simulink model "model3robots"  (R2022a)
settings: Solver=VariableStepAuto  StartTime=0.0  StopTime=Inf  RelTol=1e-3
(part 2 of 2)

== stateflow chart model3robots/Supervisor ==
  settings: executeAtInitialization=1
  state s1
  state s2
  state s3
  state s4
  state s5
  state s6
  state s7
  state s8
  state s9
  state s10
  state s11
  state s12
  state s13
  state s14
  state s15
  state s16
  state s17
  state s18
  state s19
  state s20
  state s21
  state s22
  state s23
  state s24
  state s25
  state s26
  state s27
  state s28
  state s29
  state s30
  state s31
  state s32
  state s33
  state s34
  state s35
  state s36
  state s37
  state s38
  state s39
  state s40
  state s41
  state s42
  state s43
  state s44
  state s45
  state s46
  state s47
  state s48
  state s49
  state s50
  state s51
  state s52
  state s53
  state s54
  state s55
  state s56
  state s57
  state s58
  state s59
  state s60
  state s61
  state s62
  state s63
  state s64
  state s65
  state s66
  state s67
  state s68
  state s69
  state s70
  state s71
  state s72
  state s73
  state s74
  state s75
  state s76
  state s77
  state s78
  state s79
  state s80
  state s81
  state s82
  state s83
  state s84
  state s85
  state s86
  state s87
  state s88
  state s89
  state s90
  state s91
  state s92
  state s93
  state s94
  state s95
  state s96
  state s97
  state s98
  state s99
  state s100
  state s101
  state s102
  state s103
  state s104
  state s105
  state s106
  state s107
  state s108
  state s109
  state s110
  state s111
  state s112
  state s113
  state s114
  state s115
  state s116
  state s117
  state s118
  state s119
  state s120
  state s121
  state s122
  state s123
  state s124
  state s125
  state s126
  state s127
  state s128
  state s129
  state s130
  state s131
  state s132
  state s133
  state s134
  state s135
  state s136
  state s137
  state s138
  state s139
  state s140
  state s141
  state s142
  state s143
  state s144
  state s145
  state s146
  state s147
  state s148
  state s149
  state s150
  state s151
  state s152
  state s153
  state s154
  state s155
  state s156
  state s157
  state s158
  state s159
  state s160
  state s161
  state s162
  state s163
  state s164
  state s165
  state s166
  state s167
  state s168
  state s169
  state s170
  state s171
  state s172
  state s173
  state s174
  state s175
  state s176
  state s177
  state s178
  state s179
  state s180
  state s181
  state s182
  state s183
  state s184
  state s185
  state s186
  state s187
  state s188
  state s189
  state s190
  state s191
  state s192
  state s193
  state s194
  state s195
  state s196
  state s197
  state s198
  state s199
  state s200
  state s201
  state s202
  state s203
  state s204
  state s205
  state s206
  state s207
  state s208
  state s209
  state s210
  state s211
  state s212
  state s213
  state s214
  state s215
  state s216
  state s217
  state s218
  state s219
  state s220
  state s221
  state s222
  state s223
  state s224
  state s225
  state s226
  state s227
  state s228
  state s229
  state s230
  state s231
  state s232
  state s233
  state s234
  state s235
  state s236
  state s237
  state s238
  state s239
  state s240
  state s241
  state s242
  state s243
  state s244
  state s245
  state s246
  state s247
  state s248
  state s249
  state s250
  state s251
  state s252
  state s253
  state s254
  state s255
  state s256
  state s257
  state s258
  state s259
  state s260
  state s261
  state s262
  state s263
  state s264
  state s265
  state s266
  state s267
  state s268
  state s269
  state s270
  state s271
  state s272
  state s273
  state s274
  state s275
  state s276
  state s277
  state s278
  state s279
  state s280
  state s281
  state s282
  state s283
  state s284
  state s285
  state s286
  state s287
  state s288
  state s289
  state s290
  state s291
  state s292
  state s293
  state s294
  state s295
  state s296
  state s297
  state s298
  state s299
  state s300
  state s301
  state s302
  state s303
  state s304
  state s305
  state s306
  state s307
  state s308
  state s309
  state s310
  state s311
  state s312
  state s313
  state s314
  state s315
  state s316
  state s317
  state s318
  state s319
  state s320
  state s321
  state s322
  state s323
  state s324
  state s325
  state s326
  state s327
  state s328
  state s329
  state s330
  state s331
  state s332
  state s333
  state s334
  state s335
  state s336
  state s337
  state s338
  state s339
  state s340
  state s341
  state s342
  state s343
  state s344
  state s345
  state s346
  state s347
  state s348
  state s349
  state s350
  state s351
  state s352
  state s353
  state s354
  state s355
  state s356
  state s357
  state s358
  state s359
  state s360
  state s361
  state s362
  state s363
  state s364
  state s365
  state s366
  state s367
  state s368
  state s369
  state s370
  state s371
  state s372
  state s373
  state s374
  state s375
  state s376
  state s377
  state s378
  state s379
  state s380
  state s381
  state s382
  state s383
  state s384
  state s385
  state s386
  state s387
  state s388
  state s389
  state s390
  state s391
  state s392
  state s393
  state s394
  state s395
  state s396
  state s397
  state s398
  state s399
  state s400
  state s401
  state s402
  state s403
  state s404
  state s405
  state s406
  state s407
  state s408
  state s409
  state s410
  state s411
  state s412
  state s413
  state s414
  state s415
  state s416
  state s417
  state s418
  state s419
  state s420
  state s421
  state s422
  state s423
  state s424
  state s425
  state s426
  state s427
  state s428
  state s429
  state s430
  state s431
  state s432
  state s433
  state s434
  state s435
  state s436
  state s437
  state s438
  state s439
  state s440
  state s441
  state s442
  state s443
  state s444
  state s445
  state s446
  state s447
  state s448
  state s449
  state s450
  state s451
  state s452
  state s453
  state s454
  state s455
  state s456
  state s457
  state s458
  state s459
  state s460
  state s461
  state s462
  (default) -> s19
  s4 -> s1 [order 4] : R3l {send(R3l_o);}
  s23 -> s1 [order 3] : R2l {send(R2l_o);}
  s157 -> s1 [order 1] : R1l {send(R1l_o);}
  s1 -> s157 [order 1] : R1r {send(R1r_o);}
  s1 -> s23 [order 2] : R2r {send(R2r_o);}
  s1 -> s4 [order 3] : R3r {send(R3r_o);}
  s3 -> s2 [order 3] : R3d {send(R3d_o);}
  s5 -> s2 [order 4] : R3l {send(R3l_o);}
  s9 -> s2 [order 1] : R2d {send(R2d_o);}
  s24 -> s2 [order 2] : R2l {send(R2l_o);}
  s2 -> s24 [order 1] : R2r {send(R2r_o);}
  s2 -> s9 [order 2] : R2u {send(R2u_o);}
  s2 -> s5 [order 3] : R3r {send(R3r_o);}
  s2 -> s3 [order 4] : R3u {send(R3u_o);}
  s4 -> s3 [order 3] : R3d {send(R3d_o);}
  s6 -> s3 [order 5] : R3l {send(R3l_o);}
  s10 -> s3 [order 2] : R2d {send(R2d_o);}
  s158 -> s3 [order 1] : R1l {send(R1l_o);}
  s3 -> s158 [order 1] : R1r {send(R1r_o);}
  s3 -> s10 [order 2] : R2u {send(R2u_o);}
  s3 -> s6 [order 4] : R3r {send(R3r_o);}
  s3 -> s4 [order 5] : R3u {send(R3u_o);}
  s7 -> s4 [order 5] : R3l {send(R3l_o);}
  s11 -> s4 [order 2] : R2d {send(R2d_o);}
  s159 -> s4 [order 1] : R1l {send(R1l_o);}
  s4 -> s159 [order 1] : R1r {send(R1r_o);}
  s4 -> s11 [order 2] : R2u {send(R2u_o);}
  s4 -> s7 [order 5] : R3r {send(R3r_o);}
  s6 -> s5 [order 4] : R3d {send(R3d_o);}
  s12 -> s5 [order 2] : R2d {send(R2d_o);}
  s25 -> s5 [order 4] : R2l {send(R2l_o);}
  s160 -> s5 [order 1] : R1l {send(R1l_o);}
  s5 -> s160 [order 1] : R1r {send(R1r_o);}
  s5 -> s25 [order 2] : R2r {send(R2r_o);}
  s5 -> s12 [order 3] : R2u {send(R2u_o);}
  s5 -> s6 [order 5] : R3u {send(R3u_o);}
  s7 -> s6 [order 4] : R3d {send(R3d_o);}
  s13 -> s6 [order 2] : R2d {send(R2d_o);}
  s26 -> s6 [order 4] : R2l {send(R2l_o);}
  s161 -> s6 [order 1] : R1l {send(R1l_o);}
  s6 -> s161 [order 1] : R1r {send(R1r_o);}
  s6 -> s26 [order 2] : R2r {send(R2r_o);}
  s6 -> s13 [order 3] : R2u {send(R2u_o);}
  s6 -> s7 [order 6] : R3u {send(R3u_o);}
  s6 -> s7 [order 7] : R3ureq {send(R3ureq_o);}
  s14 -> s7 [order 2] : R2d {send(R2d_o);}
  s27 -> s7 [order 4] : R2l {send(R2l_o);}
  s162 -> s7 [order 1] : R1l {send(R1l_o);}
  s7 -> s162 [order 1] : R1r {send(R1r_o);}
  s7 -> s27 [order 2] : R2r {send(R2r_o);}
  s7 -> s14 [order 3] : R2u {send(R2u_o);}
  s10 -> s8 [order 5] : R3l {send(R3l_o);}
  s28 -> s8 [order 3] : R2l {send(R2l_o);}
  s164 -> s8 [order 1] : R1l {send(R1l_o);}
  s8 -> s164 [order 1] : R1r {send(R1r_o);}
  s8 -> s28 [order 2] : R2r {send(R2r_o);}
  s8 -> s10 [order 3] : R3r {send(R3r_o);}
  s10 -> s9 [order 4] : R3d {send(R3d_o);}
  s12 -> s9 [order 4] : R3l {send(R3l_o);}
  s30 -> s9 [order 3] : R2l {send(R2l_o);}
  s9 -> s30 [order 2] : R2r {send(R2r_o);}
  s9 -> s12 [order 3] : R3r {send(R3r_o);}
  s9 -> s10 [order 4] : R3u {send(R3u_o);}
  s11 -> s10 [order 3] : R3d {send(R3d_o);}
  s13 -> s10 [order 5] : R3l {send(R3l_o);}
  s31 -> s10 [order 3] : R2l {send(R2l_o);}
  s165 -> s10 [order 1] : R1l {send(R1l_o);}
  s10 -> s165 [order 1] : R1r {send(R1r_o);}
  s10 -> s31 [order 3] : R2r {send(R2r_o);}
  s10 -> s13 [order 6] : R3r {send(R3r_o);}
  s10 -> s11 [order 7] : R3u {send(R3u_o);}
  s14 -> s11 [order 5] : R3l {send(R3l_o);}
  s166 -> s11 [order 1] : R1l {send(R1l_o);}
  s11 -> s166 [order 1] : R1r {send(R1r_o);}
  s11 -> s14 [order 4] : R3r {send(R3r_o);}
  s13 -> s12 [order 4] : R3d {send(R3d_o);}
  s32 -> s12 [order 4] : R2l {send(R2l_o);}
  s167 -> s12 [order 1] : R1l {send(R1l_o);}
  s12 -> s167 [order 1] : R1r {send(R1r_o);}
  s12 -> s32 [order 3] : R2r {send(R2r_o);}
  s12 -> s13 [order 5] : R3u {send(R3u_o);}
  s14 -> s13 [order 4] : R3d {send(R3d_o);}
  s33 -> s13 [order 4] : R2l {send(R2l_o);}
  s168 -> s13 [order 1] : R1l {send(R1l_o);}
  s13 -> s168 [order 1] : R1r {send(R1r_o);}
  s13 -> s33 [order 3] : R2r {send(R2r_o);}
  s13 -> s14 [order 6] : R3u {send(R3u_o);}
  s13 -> s14 [order 7] : R3ureq {send(R3ureq_o);}
  s34 -> s14 [order 4] : R2l {send(R2l_o);}
  s169 -> s14 [order 1] : R1l {send(R1l_o);}
  s14 -> s169 [order 1] : R1r {send(R1r_o);}
  s14 -> s34 [order 3] : R2r {send(R2r_o);}
  s16 -> s15 [order 3] : R3d {send(R3d_o);}
  s17 -> s15 [order 3] : R3l {send(R3l_o);}
  s22 -> s15 [order 2] : R2d {send(R2d_o);}
  s35 -> s15 [order 2] : R2l {send(R2l_o);}
  s15 -> s35 [order 1] : R2r {send(R2r_o);}
  s15 -> s22 [order 2] : R2u {send(R2u_o);}
  s15 -> s17 [order 3] : R3r {send(R3r_o);}
  s15 -> s16 [order 4] : R3u {send(R3u_o);}
  s18 -> s16 [order 4] : R3l {send(R3l_o);}
  s23 -> s16 [order 2] : R2d {send(R2d_o);}
  s36 -> s16 [order 2] : R2l {send(R2l_o);}
  s16 -> s36 [order 1] : R2r {send(R2r_o);}
  s16 -> s23 [order 2] : R2u {send(R2u_o);}
  s16 -> s18 [order 4] : R3r {send(R3r_o);}
  s18 -> s17 [order 3] : R3d {send(R3d_o);}
  s20 -> s17 [order 5] : R3l {send(R3l_o);}
  s38 -> s17 [order 3] : R2l {send(R2l_o);}
  s62 -> s17 [order 1] : R1d {send(R1d_o);}
  s17 -> s62 [order 1] : R1u {send(R1u_o);}
  s17 -> s38 [order 2] : R2r {send(R2r_o);}
  s17 -> s20 [order 4] : R3r {send(R3r_o);}
  s17 -> s18 [order 5] : R3u {send(R3u_o);}
  s21 -> s18 [order 5] : R3l {send(R3l_o);}
  s39 -> s18 [order 3] : R2l {send(R2l_o);}
  s63 -> s18 [order 1] : R1d {send(R1d_o);}
  s18 -> s63 [order 1] : R1u {send(R1u_o);}
  s18 -> s39 [order 2] : R2r {send(R2r_o);}
  s18 -> s21 [order 5] : R3r {send(R3r_o);}
  s20 -> s19 [order 4] : R3d {send(R3d_o);}
  s25 -> s19 [order 3] : R2d {send(R2d_o);}
  s64 -> s19 [order 1] : R1d {send(R1d_o);}
  s19 -> s64 [order 1] : R1u {send(R1u_o);}
  s19 -> s25 [order 2] : R2u {send(R2u_o);}
  s19 -> s20 [order 3] : R3u {send(R3u_o);}
  s21 -> s20 [order 4] : R3d {send(R3d_o);}
  s26 -> s20 [order 3] : R2d {send(R2d_o);}
  s40 -> s20 [order 3] : R2l {send(R2l_o);}
  s65 -> s20 [order 1] : R1d {send(R1d_o);}
  s20 -> s65 [order 1] : R1u {send(R1u_o);}
  s20 -> s40 [order 2] : R2r {send(R2r_o);}
  s20 -> s26 [order 3] : R2u {send(R2u_o);}
  s20 -> s21 [order 6] : R3u {send(R3u_o);}
  s20 -> s21 [order 7] : R3ureq {send(R3ureq_o);}
  s27 -> s21 [order 3] : R2d {send(R2d_o);}
  s41 -> s21 [order 3] : R2l {send(R2l_o);}
  s66 -> s21 [order 1] : R1d {send(R1d_o);}
  s21 -> s66 [order 1] : R1u {send(R1u_o);}
  s21 -> s41 [order 2] : R2r {send(R2r_o);}
  s21 -> s27 [order 3] : R2u {send(R2u_o);}
  s23 -> s22 [order 7] : R3d {send(R3d_o);}
  s28 -> s22 [order 2] : R2d {send(R2d_o);}
  s42 -> s22 [order 3] : R2l {send(R2l_o);}
  s171 -> s22 [order 1] : R1l {send(R1l_o);}
  s22 -> s171 [order 1] : R1r {send(R1r_o);}
  s22 -> s42 [order 3] : R2r {send(R2r_o);}
  s22 -> s28 [order 4] : R2u {send(R2u_o);}
  s22 -> s28 [order 5] : R2ureq {send(R2ureq_o);}
  s22 -> s23 [order 6] : R3u {send(R3u_o);}
  s29 -> s23 [order 2] : R2d {send(R2d_o);}
  s43 -> s23 [order 3] : R2l {send(R2l_o);}
  s172 -> s23 [order 1] : R1l {send(R1l_o);}
  s23 -> s172 [order 1] : R1r {send(R1r_o);}
  s23 -> s43 [order 4] : R2r {send(R2r_o);}
  s23 -> s29 [order 5] : R2u {send(R2u_o);}
  s23 -> s29 [order 6] : R2ureq {send(R2ureq_o);}
  s25 -> s24 [order 8] : R3l {send(R3l_o);}
  s30 -> s24 [order 2] : R2d {send(R2d_o);}
  s44 -> s24 [order 3] : R2l {send(R2l_o);}
  s68 -> s24 [order 1] : R1d {send(R1d_o);}
  s24 -> s68 [order 1] : R1u {send(R1u_o);}
  s24 -> s44 [order 3] : R2r {send(R2r_o);}
  s24 -> s30 [order 4] : R2u {send(R2u_o);}
  s24 -> s30 [order 5] : R2ureq {send(R2ureq_o);}
  s24 -> s25 [order 6] : R3r {send(R3r_o);}
  s26 -> s25 [order 7] : R3d {send(R3d_o);}
  s32 -> s25 [order 3] : R2d {send(R2d_o);}
  s47 -> s25 [order 3] : R2l {send(R2l_o);}
  s69 -> s25 [order 1] : R1d {send(R1d_o);}
  s173 -> s25 [order 1] : R1l {send(R1l_o);}
  s25 -> s173 [order 1] : R1r {send(R1r_o);}
  s25 -> s69 [order 2] : R1u {send(R1u_o);}
  s25 -> s47 [order 5] : R2r {send(R2r_o);}
  s25 -> s32 [order 6] : R2u {send(R2u_o);}
  s25 -> s32 [order 7] : R2ureq {send(R2ureq_o);}
  s25 -> s26 [order 9] : R3u {send(R3u_o);}
  s27 -> s26 [order 8] : R3d {send(R3d_o);}
  s33 -> s26 [order 3] : R2d {send(R2d_o);}
  s70 -> s26 [order 1] : R1d {send(R1d_o);}
  s174 -> s26 [order 1] : R1l {send(R1l_o);}
  s26 -> s174 [order 1] : R1r {send(R1r_o);}
  s26 -> s70 [order 2] : R1u {send(R1u_o);}
  s26 -> s33 [order 5] : R2u {send(R2u_o);}
  s26 -> s33 [order 6] : R2ureq {send(R2ureq_o);}
  s26 -> s27 [order 8] : R3u {send(R3u_o);}
  s26 -> s27 [order 9] : R3ureq {send(R3ureq_o);}
  s34 -> s27 [order 3] : R2d {send(R2d_o);}
  s48 -> s27 [order 4] : R2l {send(R2l_o);}
  s71 -> s27 [order 1] : R1d {send(R1d_o);}
  s175 -> s27 [order 1] : R1l {send(R1l_o);}
  s27 -> s175 [order 1] : R1r {send(R1r_o);}
  s27 -> s71 [order 2] : R1u {send(R1u_o);}
  s27 -> s48 [order 5] : R2r {send(R2r_o);}
  s27 -> s34 [order 6] : R2u {send(R2u_o);}
  s27 -> s34 [order 7] : R2ureq {send(R2ureq_o);}
  s29 -> s28 [order 4] : R3d {send(R3d_o);}
  s31 -> s28 [order 6] : R3l {send(R3l_o);}
  s49 -> s28 [order 3] : R2l {send(R2l_o);}
  s177 -> s28 [order 1] : R1l {send(R1l_o);}
  s28 -> s177 [order 1] : R1r {send(R1r_o);}
  s28 -> s49 [order 4] : R2r {send(R2r_o);}
  s28 -> s31 [order 5] : R3r {send(R3r_o);}
  s28 -> s29 [order 6] : R3u {send(R3u_o);}
  s50 -> s29 [order 3] : R2l {send(R2l_o);}
  s178 -> s29 [order 1] : R1l {send(R1l_o);}
  s29 -> s178 [order 1] : R1r {send(R1r_o);}
  s29 -> s50 [order 3] : R2r {send(R2r_o);}
  s31 -> s30 [order 5] : R3d {send(R3d_o);}
  s32 -> s30 [order 6] : R3l {send(R3l_o);}
  s51 -> s30 [order 3] : R2l {send(R2l_o);}
  s73 -> s30 [order 1] : R1d {send(R1d_o);}
  s30 -> s73 [order 1] : R1u {send(R1u_o);}
  s30 -> s51 [order 4] : R2r {send(R2r_o);}
  s30 -> s32 [order 5] : R3r {send(R3r_o);}
  s30 -> s31 [order 6] : R3u {send(R3u_o);}
  s33 -> s31 [order 6] : R3l {send(R3l_o);}
  s52 -> s31 [order 4] : R2l {send(R2l_o);}
  s74 -> s31 [order 1] : R1d {send(R1d_o);}
  s179 -> s31 [order 1] : R1l {send(R1l_o);}
  s31 -> s179 [order 1] : R1r {send(R1r_o);}
  s31 -> s74 [order 2] : R1u {send(R1u_o);}
  s31 -> s52 [order 4] : R2r {send(R2r_o);}
  s31 -> s33 [order 7] : R3r {send(R3r_o);}
  s33 -> s32 [order 5] : R3d {send(R3d_o);}
  s54 -> s32 [order 4] : R2l {send(R2l_o);}
  s75 -> s32 [order 1] : R1d {send(R1d_o);}
  s180 -> s32 [order 1] : R1l {send(R1l_o);}
  s32 -> s180 [order 1] : R1r {send(R1r_o);}
  s32 -> s75 [order 2] : R1u {send(R1u_o);}
  s32 -> s54 [order 5] : R2r {send(R2r_o);}
  s32 -> s33 [order 7] : R3u {send(R3u_o);}
  s34 -> s33 [order 5] : R3d {send(R3d_o);}
  s76 -> s33 [order 1] : R1d {send(R1d_o);}
  s181 -> s33 [order 1] : R1l {send(R1l_o);}
  s33 -> s181 [order 1] : R1r {send(R1r_o);}
  s33 -> s76 [order 2] : R1u {send(R1u_o);}
  s33 -> s34 [order 7] : R3u {send(R3u_o);}
  s33 -> s34 [order 8] : R3ureq {send(R3ureq_o);}
  s77 -> s34 [order 1] : R1d {send(R1d_o);}
  s182 -> s34 [order 1] : R1l {send(R1l_o);}
  s34 -> s182 [order 1] : R1r {send(R1r_o);}
  s34 -> s77 [order 2] : R1u {send(R1u_o);}
  s36 -> s35 [order 4] : R3d {send(R3d_o);}
  s38 -> s35 [order 6] : R3l {send(R3l_o);}
  s42 -> s35 [order 2] : R2d {send(R2d_o);}
  s184 -> s35 [order 1] : R1l {send(R1l_o);}
  s35 -> s184 [order 1] : R1r {send(R1r_o);}
  s35 -> s42 [order 3] : R2u {send(R2u_o);}
  s35 -> s38 [order 4] : R3r {send(R3r_o);}
  s35 -> s36 [order 5] : R3u {send(R3u_o);}
  s39 -> s36 [order 6] : R3l {send(R3l_o);}
  s43 -> s36 [order 2] : R2d {send(R2d_o);}
  s185 -> s36 [order 1] : R1l {send(R1l_o);}
  s36 -> s185 [order 1] : R1r {send(R1r_o);}
  s36 -> s43 [order 3] : R2u {send(R2u_o);}
  s36 -> s39 [order 5] : R3r {send(R3r_o);}
  s38 -> s37 [order 5] : R3d {send(R3d_o);}
  s44 -> s37 [order 2] : R2d {send(R2d_o);}
  s79 -> s37 [order 1] : R1d {send(R1d_o);}
  s37 -> s79 [order 1] : R1u {send(R1u_o);}
  s37 -> s44 [order 2] : R2u {send(R2u_o);}
  s37 -> s38 [order 3] : R3u {send(R3u_o);}
  s39 -> s38 [order 5] : R3d {send(R3d_o);}
  s40 -> s38 [order 4] : R3l {send(R3l_o);}
  s45 -> s38 [order 3] : R2d {send(R2d_o);}
  s80 -> s38 [order 1] : R1d {send(R1d_o);}
  s186 -> s38 [order 1] : R1l {send(R1l_o);}
  s38 -> s186 [order 1] : R1r {send(R1r_o);}
  s38 -> s80 [order 2] : R1u {send(R1u_o);}
  s38 -> s45 [order 4] : R2u {send(R2u_o);}
  s38 -> s40 [order 7] : R3r {send(R3r_o);}
  s38 -> s39 [order 8] : R3u {send(R3u_o);}
  s41 -> s39 [order 6] : R3l {send(R3l_o);}
  s46 -> s39 [order 3] : R2d {send(R2d_o);}
  s81 -> s39 [order 1] : R1d {send(R1d_o);}
  s187 -> s39 [order 1] : R1l {send(R1l_o);}
  s39 -> s187 [order 1] : R1r {send(R1r_o);}
  s39 -> s81 [order 2] : R1u {send(R1u_o);}
  s39 -> s46 [order 4] : R2u {send(R2u_o);}
  s39 -> s41 [order 7] : R3r {send(R3r_o);}
  s41 -> s40 [order 5] : R3d {send(R3d_o);}
  s82 -> s40 [order 1] : R1d {send(R1d_o);}
  s188 -> s40 [order 1] : R1l {send(R1l_o);}
  s40 -> s188 [order 1] : R1r {send(R1r_o);}
  s40 -> s82 [order 2] : R1u {send(R1u_o);}
  s40 -> s41 [order 5] : R3u {send(R3u_o);}
  s40 -> s41 [order 6] : R3ureq {send(R3ureq_o);}
  s48 -> s41 [order 3] : R2d {send(R2d_o);}
  s83 -> s41 [order 1] : R1d {send(R1d_o);}
  s189 -> s41 [order 1] : R1l {send(R1l_o);}
  s41 -> s189 [order 1] : R1r {send(R1r_o);}
  s41 -> s83 [order 2] : R1u {send(R1u_o);}
  s41 -> s48 [order 4] : R2u {send(R2u_o);}
  s43 -> s42 [order 5] : R3d {send(R3d_o);}
  s45 -> s42 [order 6] : R3l {send(R3l_o);}
  s49 -> s42 [order 2] : R2d {send(R2d_o);}
  s191 -> s42 [order 1] : R1l {send(R1l_o);}
  s42 -> s191 [order 1] : R1r {send(R1r_o);}
  s42 -> s49 [order 4] : R2u {send(R2u_o);}
  s42 -> s45 [order 5] : R3r {send(R3r_o);}
  s42 -> s43 [order 6] : R3u {send(R3u_o);}
  s46 -> s43 [order 6] : R3l {send(R3l_o);}
  s50 -> s43 [order 2] : R2d {send(R2d_o);}
  s192 -> s43 [order 1] : R1l {send(R1l_o);}
  s43 -> s192 [order 1] : R1r {send(R1r_o);}
  s43 -> s50 [order 4] : R2u {send(R2u_o);}
  s43 -> s46 [order 6] : R3r {send(R3r_o);}
  s45 -> s44 [order 5] : R3d {send(R3d_o);}
  s47 -> s44 [order 5] : R3l {send(R3l_o);}
  s51 -> s44 [order 2] : R2d {send(R2d_o);}
  s85 -> s44 [order 1] : R1d {send(R1d_o);}
  s44 -> s85 [order 1] : R1u {send(R1u_o);}
  s44 -> s51 [order 4] : R2u {send(R2u_o);}
  s44 -> s47 [order 5] : R3r {send(R3r_o);}
  s44 -> s45 [order 6] : R3u {send(R3u_o);}
  s46 -> s45 [order 5] : R3d {send(R3d_o);}
  s52 -> s45 [order 3] : R2d {send(R2d_o);}
  s86 -> s45 [order 1] : R1d {send(R1d_o);}
  s193 -> s45 [order 1] : R1l {send(R1l_o);}
  s45 -> s193 [order 1] : R1r {send(R1r_o);}
  s45 -> s86 [order 2] : R1u {send(R1u_o);}
  s45 -> s52 [order 4] : R2u {send(R2u_o);}
  s45 -> s46 [order 7] : R3u {send(R3u_o);}
  s48 -> s46 [order 5] : R3l {send(R3l_o);}
  s53 -> s46 [order 3] : R2d {send(R2d_o);}
  s87 -> s46 [order 1] : R1d {send(R1d_o);}
  s194 -> s46 [order 1] : R1l {send(R1l_o);}
  s46 -> s194 [order 1] : R1r {send(R1r_o);}
  s46 -> s87 [order 2] : R1u {send(R1u_o);}
  s46 -> s53 [order 4] : R2u {send(R2u_o);}
  s46 -> s48 [order 7] : R3r {send(R3r_o);}
  s54 -> s47 [order 3] : R2d {send(R2d_o);}
  s88 -> s47 [order 1] : R1d {send(R1d_o);}
  s195 -> s47 [order 1] : R1l {send(R1l_o);}
  s47 -> s195 [order 1] : R1r {send(R1r_o);}
  s47 -> s88 [order 2] : R1u {send(R1u_o);}
  s47 -> s54 [order 4] : R2u {send(R2u_o);}
  s89 -> s48 [order 1] : R1d {send(R1d_o);}
  s196 -> s48 [order 1] : R1l {send(R1l_o);}
  s48 -> s196 [order 1] : R1r {send(R1r_o);}
  s48 -> s89 [order 2] : R1u {send(R1u_o);}
  s50 -> s49 [order 4] : R3d {send(R3d_o);}
  s52 -> s49 [order 6] : R3l {send(R3l_o);}
  s198 -> s49 [order 1] : R1l {send(R1l_o);}
  s49 -> s198 [order 1] : R1r {send(R1r_o);}
  s49 -> s52 [order 4] : R3r {send(R3r_o);}
  s49 -> s50 [order 5] : R3u {send(R3u_o);}
  s53 -> s50 [order 5] : R3l {send(R3l_o);}
  s199 -> s50 [order 1] : R1l {send(R1l_o);}
  s50 -> s199 [order 1] : R1r {send(R1r_o);}
  s50 -> s53 [order 5] : R3r {send(R3r_o);}
  s52 -> s51 [order 5] : R3d {send(R3d_o);}
  s54 -> s51 [order 5] : R3l {send(R3l_o);}
  s91 -> s51 [order 1] : R1d {send(R1d_o);}
  s51 -> s91 [order 1] : R1u {send(R1u_o);}
  s51 -> s54 [order 4] : R3r {send(R3r_o);}
  s51 -> s52 [order 5] : R3u {send(R3u_o);}
  s53 -> s52 [order 4] : R3d {send(R3d_o);}
  s92 -> s52 [order 1] : R1d {send(R1d_o);}
  s200 -> s52 [order 1] : R1l {send(R1l_o);}
  s52 -> s200 [order 1] : R1r {send(R1r_o);}
  s52 -> s92 [order 2] : R1u {send(R1u_o);}
  s52 -> s53 [order 7] : R3u {send(R3u_o);}
  s93 -> s53 [order 1] : R1d {send(R1d_o);}
  s201 -> s53 [order 1] : R1l {send(R1l_o);}
  s53 -> s201 [order 1] : R1r {send(R1r_o);}
  s53 -> s93 [order 2] : R1u {send(R1u_o);}
  s94 -> s54 [order 1] : R1d {send(R1d_o);}
  s202 -> s54 [order 1] : R1l {send(R1l_o);}
  s54 -> s202 [order 1] : R1r {send(R1r_o);}
  s54 -> s94 [order 2] : R1u {send(R1u_o);}
  s56 -> s55 [order 4] : R3d {send(R3d_o);}
  s58 -> s55 [order 5] : R3l {send(R3l_o);}
  s96 -> s55 [order 1] : R1d {send(R1d_o);}
  s205 -> s55 [order 1] : R1l {send(R1l_o);}
  s55 -> s205 [order 1] : R1r {send(R1r_o);}
  s55 -> s96 [order 2] : R1u {send(R1u_o);}
  s55 -> s96 [order 3] : R1ureq {send(R1ureq_o);}
  s55 -> s58 [order 4] : R3r {send(R3r_o);}
  s55 -> s56 [order 5] : R3u {send(R3u_o);}
  s57 -> s56 [order 5] : R3d {send(R3d_o);}
  s59 -> s56 [order 6] : R3l {send(R3l_o);}
  s62 -> s56 [order 4] : R2l {send(R2l_o);}
  s97 -> s56 [order 1] : R1d {send(R1d_o);}
  s56 -> s97 [order 1] : R1u {send(R1u_o);}
  s56 -> s97 [order 2] : R1ureq {send(R1ureq_o);}
  s56 -> s62 [order 3] : R2r {send(R2r_o);}
  s56 -> s59 [order 5] : R3r {send(R3r_o);}
  s56 -> s57 [order 6] : R3u {send(R3u_o);}
  s60 -> s57 [order 6] : R3l {send(R3l_o);}
  s63 -> s57 [order 5] : R2l {send(R2l_o);}
  s98 -> s57 [order 1] : R1d {send(R1d_o);}
  s206 -> s57 [order 2] : R1l {send(R1l_o);}
  s57 -> s206 [order 1] : R1r {send(R1r_o);}
  s57 -> s98 [order 2] : R1u {send(R1u_o);}
  s57 -> s98 [order 3] : R1ureq {send(R1ureq_o);}
  s57 -> s63 [order 4] : R2r {send(R2r_o);}
  s57 -> s60 [order 6] : R3r {send(R3r_o);}
  s59 -> s58 [order 5] : R3d {send(R3d_o);}
  s64 -> s58 [order 5] : R2l {send(R2l_o);}
  s99 -> s58 [order 1] : R1d {send(R1d_o);}
  s207 -> s58 [order 2] : R1l {send(R1l_o);}
  s58 -> s207 [order 1] : R1r {send(R1r_o);}
  s58 -> s99 [order 2] : R1u {send(R1u_o);}
  s58 -> s99 [order 3] : R1ureq {send(R1ureq_o);}
  s58 -> s64 [order 4] : R2r {send(R2r_o);}
  s58 -> s59 [order 6] : R3u {send(R3u_o);}
  s60 -> s59 [order 5] : R3d {send(R3d_o);}
  s65 -> s59 [order 5] : R2l {send(R2l_o);}
  s100 -> s59 [order 1] : R1d {send(R1d_o);}
  s208 -> s59 [order 2] : R1l {send(R1l_o);}
  s59 -> s208 [order 1] : R1r {send(R1r_o);}
  s59 -> s100 [order 2] : R1u {send(R1u_o);}
  s59 -> s100 [order 3] : R1ureq {send(R1ureq_o);}
  s59 -> s65 [order 4] : R2r {send(R2r_o);}
  s59 -> s60 [order 7] : R3u {send(R3u_o);}
  s59 -> s60 [order 8] : R3ureq {send(R3ureq_o);}
  s66 -> s60 [order 5] : R2l {send(R2l_o);}
  s101 -> s60 [order 1] : R1d {send(R1d_o);}
  s209 -> s60 [order 2] : R1l {send(R1l_o);}
  s60 -> s209 [order 1] : R1r {send(R1r_o);}
  s60 -> s101 [order 2] : R1u {send(R1u_o);}
  s60 -> s101 [order 3] : R1ureq {send(R1ureq_o);}
  s60 -> s66 [order 4] : R2r {send(R2r_o);}
  s67 -> s61 [order 3] : R2d {send(R2d_o);}
  s78 -> s61 [order 4] : R2l {send(R2l_o);}
  s109 -> s61 [order 1] : R1d {send(R1d_o);}
  s224 -> s61 [order 1] : R1l {send(R1l_o);}
  s61 -> s224 [order 1] : R1r {send(R1r_o);}
  s61 -> s109 [order 2] : R1u {send(R1u_o);}
  s61 -> s109 [order 3] : R1ureq {send(R1ureq_o);}
  s61 -> s78 [order 4] : R2r {send(R2r_o);}
  s61 -> s67 [order 5] : R2u {send(R2u_o);}
  s63 -> s62 [order 7] : R3d {send(R3d_o);}
  s65 -> s62 [order 9] : R3l {send(R3l_o);}
  s80 -> s62 [order 4] : R2l {send(R2l_o);}
  s111 -> s62 [order 1] : R1d {send(R1d_o);}
  s62 -> s111 [order 2] : R1u {send(R1u_o);}
  s62 -> s111 [order 3] : R1ureq {send(R1ureq_o);}
  s62 -> s80 [order 5] : R2r {send(R2r_o);}
  s62 -> s65 [order 6] : R3r {send(R3r_o);}
  s62 -> s63 [order 7] : R3u {send(R3u_o);}
  s66 -> s63 [order 9] : R3l {send(R3l_o);}
  s81 -> s63 [order 5] : R2l {send(R2l_o);}
  s112 -> s63 [order 1] : R1d {send(R1d_o);}
  s227 -> s63 [order 1] : R1l {send(R1l_o);}
  s63 -> s227 [order 2] : R1r {send(R1r_o);}
  s63 -> s112 [order 3] : R1u {send(R1u_o);}
  s63 -> s112 [order 4] : R1ureq {send(R1ureq_o);}
  s63 -> s81 [order 6] : R2r {send(R2r_o);}
  s63 -> s66 [order 8] : R3r {send(R3r_o);}
  s65 -> s64 [order 8] : R3d {send(R3d_o);}
  s69 -> s64 [order 4] : R2d {send(R2d_o);}
  s113 -> s64 [order 1] : R1d {send(R1d_o);}
  s228 -> s64 [order 1] : R1l {send(R1l_o);}
  s64 -> s228 [order 2] : R1r {send(R1r_o);}
  s64 -> s113 [order 3] : R1u {send(R1u_o);}
  s64 -> s113 [order 4] : R1ureq {send(R1ureq_o);}
  s64 -> s69 [order 6] : R2u {send(R2u_o);}
  s64 -> s65 [order 7] : R3u {send(R3u_o);}
  s66 -> s65 [order 8] : R3d {send(R3d_o);}
  s70 -> s65 [order 4] : R2d {send(R2d_o);}
  s82 -> s65 [order 5] : R2l {send(R2l_o);}
  s114 -> s65 [order 1] : R1d {send(R1d_o);}
  s229 -> s65 [order 1] : R1l {send(R1l_o);}
  s65 -> s229 [order 2] : R1r {send(R1r_o);}
  s65 -> s114 [order 3] : R1u {send(R1u_o);}
  s65 -> s114 [order 4] : R1ureq {send(R1ureq_o);}
  s65 -> s82 [order 6] : R2r {send(R2r_o);}
  s65 -> s70 [order 7] : R2u {send(R2u_o);}
  s65 -> s66 [order 10] : R3u {send(R3u_o);}
  s65 -> s66 [order 11] : R3ureq {send(R3ureq_o);}
  s71 -> s66 [order 4] : R2d {send(R2d_o);}
  s83 -> s66 [order 5] : R2l {send(R2l_o);}
  s115 -> s66 [order 1] : R1d {send(R1d_o);}
  s230 -> s66 [order 1] : R1l {send(R1l_o);}
  s66 -> s230 [order 2] : R1r {send(R1r_o);}
  s66 -> s115 [order 3] : R1u {send(R1u_o);}
  s66 -> s115 [order 4] : R1ureq {send(R1ureq_o);}
  s66 -> s83 [order 6] : R2r {send(R2r_o);}
  s66 -> s71 [order 7] : R2u {send(R2u_o);}
  s68 -> s67 [order 7] : R3l {send(R3l_o);}
  s72 -> s67 [order 4] : R2d {send(R2d_o);}
  s84 -> s67 [order 5] : R2l {send(R2l_o);}
  s116 -> s67 [order 1] : R1d {send(R1d_o);}
  s67 -> s116 [order 1] : R1u {send(R1u_o);}
  s67 -> s116 [order 2] : R1ureq {send(R1ureq_o);}
  s67 -> s84 [order 4] : R2r {send(R2r_o);}
  s67 -> s72 [order 5] : R2u {send(R2u_o);}
  s67 -> s72 [order 6] : R2ureq {send(R2ureq_o);}
  s67 -> s68 [order 7] : R3r {send(R3r_o);}
  s69 -> s68 [order 8] : R3l {send(R3l_o);}
  s73 -> s68 [order 5] : R2d {send(R2d_o);}
  s85 -> s68 [order 6] : R2l {send(R2l_o);}
  s118 -> s68 [order 1] : R1d {send(R1d_o);}
  s68 -> s118 [order 2] : R1u {send(R1u_o);}
  s68 -> s118 [order 3] : R1ureq {send(R1ureq_o);}
  s68 -> s85 [order 4] : R2r {send(R2r_o);}
  s68 -> s73 [order 5] : R2u {send(R2u_o);}
  s68 -> s73 [order 6] : R2ureq {send(R2ureq_o);}
  s68 -> s69 [order 8] : R3r {send(R3r_o);}
  s70 -> s69 [order 7] : R3d {send(R3d_o);}
  s75 -> s69 [order 5] : R2d {send(R2d_o);}
  s88 -> s69 [order 5] : R2l {send(R2l_o);}
  s119 -> s69 [order 1] : R1d {send(R1d_o);}
  s69 -> s119 [order 2] : R1u {send(R1u_o);}
  s69 -> s119 [order 3] : R1ureq {send(R1ureq_o);}
  s69 -> s88 [order 5] : R2r {send(R2r_o);}
  s69 -> s75 [order 6] : R2u {send(R2u_o);}
  s69 -> s75 [order 7] : R2ureq {send(R2ureq_o);}
  s69 -> s70 [order 9] : R3u {send(R3u_o);}
  s71 -> s70 [order 8] : R3d {send(R3d_o);}
  s76 -> s70 [order 5] : R2d {send(R2d_o);}
  s120 -> s70 [order 1] : R1d {send(R1d_o);}
  s70 -> s120 [order 2] : R1u {send(R1u_o);}
  s70 -> s120 [order 3] : R1ureq {send(R1ureq_o);}
  s70 -> s76 [order 5] : R2u {send(R2u_o);}
  s70 -> s76 [order 6] : R2ureq {send(R2ureq_o);}
  s70 -> s71 [order 8] : R3u {send(R3u_o);}
  s70 -> s71 [order 9] : R3ureq {send(R3ureq_o);}
  s77 -> s71 [order 5] : R2d {send(R2d_o);}
  s89 -> s71 [order 6] : R2l {send(R2l_o);}
  s121 -> s71 [order 1] : R1d {send(R1d_o);}
  s71 -> s121 [order 2] : R1u {send(R1u_o);}
  s71 -> s121 [order 3] : R1ureq {send(R1ureq_o);}
  s71 -> s89 [order 5] : R2r {send(R2r_o);}
  s71 -> s77 [order 6] : R2u {send(R2u_o);}
  s71 -> s77 [order 7] : R2ureq {send(R2ureq_o);}
  s73 -> s72 [order 7] : R3l {send(R3l_o);}
  s90 -> s72 [order 5] : R2l {send(R2l_o);}
  s122 -> s72 [order 1] : R1d {send(R1d_o);}
  s231 -> s72 [order 2] : R1l {send(R1l_o);}
  s72 -> s231 [order 1] : R1r {send(R1r_o);}
  s72 -> s122 [order 2] : R1u {send(R1u_o);}
  s72 -> s122 [order 3] : R1ureq {send(R1ureq_o);}
  s72 -> s90 [order 5] : R2r {send(R2r_o);}
  s72 -> s73 [order 6] : R3r {send(R3r_o);}
  s74 -> s73 [order 5] : R3d {send(R3d_o);}
  s75 -> s73 [order 7] : R3l {send(R3l_o);}
  s91 -> s73 [order 6] : R2l {send(R2l_o);}
  s124 -> s73 [order 1] : R1d {send(R1d_o);}
  s234 -> s73 [order 1] : R1l {send(R1l_o);}
  s73 -> s234 [order 2] : R1r {send(R1r_o);}
  s73 -> s124 [order 3] : R1u {send(R1u_o);}
  s73 -> s124 [order 4] : R1ureq {send(R1ureq_o);}
  s73 -> s91 [order 6] : R2r {send(R2r_o);}
  s73 -> s75 [order 8] : R3r {send(R3r_o);}
  s73 -> s74 [order 9] : R3u {send(R3u_o);}
  s76 -> s74 [order 7] : R3l {send(R3l_o);}
  s92 -> s74 [order 5] : R2l {send(R2l_o);}
  s125 -> s74 [order 1] : R1d {send(R1d_o);}
  s74 -> s125 [order 2] : R1u {send(R1u_o);}
  s74 -> s125 [order 3] : R1ureq {send(R1ureq_o);}
  s74 -> s92 [order 4] : R2r {send(R2r_o);}
  s74 -> s76 [order 6] : R3r {send(R3r_o);}
  s76 -> s75 [order 6] : R3d {send(R3d_o);}
  s94 -> s75 [order 6] : R2l {send(R2l_o);}
  s126 -> s75 [order 1] : R1d {send(R1d_o);}
  s235 -> s75 [order 2] : R1l {send(R1l_o);}
  s75 -> s235 [order 2] : R1r {send(R1r_o);}
  s75 -> s126 [order 3] : R1u {send(R1u_o);}
  s75 -> s126 [order 4] : R1ureq {send(R1ureq_o);}
  s75 -> s94 [order 6] : R2r {send(R2r_o);}
  s75 -> s76 [order 8] : R3u {send(R3u_o);}
  s77 -> s76 [order 6] : R3d {send(R3d_o);}
  s127 -> s76 [order 1] : R1d {send(R1d_o);}
  s236 -> s76 [order 2] : R1l {send(R1l_o);}
  s76 -> s236 [order 2] : R1r {send(R1r_o);}
  s76 -> s127 [order 3] : R1u {send(R1u_o);}
  s76 -> s127 [order 4] : R1ureq {send(R1ureq_o);}
  s76 -> s77 [order 8] : R3u {send(R3u_o);}
  s76 -> s77 [order 9] : R3ureq {send(R3ureq_o);}
  s128 -> s77 [order 1] : R1d {send(R1d_o);}
  s237 -> s77 [order 2] : R1l {send(R1l_o);}
  s77 -> s237 [order 2] : R1r {send(R1r_o);}
  s77 -> s128 [order 3] : R1u {send(R1u_o);}
  s77 -> s128 [order 4] : R1ureq {send(R1ureq_o);}
  s79 -> s78 [order 6] : R3l {send(R3l_o);}
  s84 -> s78 [order 4] : R2d {send(R2d_o);}
  s129 -> s78 [order 1] : R1d {send(R1d_o);}
  s238 -> s78 [order 2] : R1l {send(R1l_o);}
  s78 -> s238 [order 1] : R1r {send(R1r_o);}
  s78 -> s129 [order 2] : R1u {send(R1u_o);}
  s78 -> s129 [order 3] : R1ureq {send(R1ureq_o);}
  s78 -> s84 [order 5] : R2u {send(R2u_o);}
  s78 -> s79 [order 6] : R3r {send(R3r_o);}
  s80 -> s79 [order 6] : R3d {send(R3d_o);}
  s85 -> s79 [order 5] : R2d {send(R2d_o);}
  s131 -> s79 [order 1] : R1d {send(R1d_o);}
  s241 -> s79 [order 1] : R1l {send(R1l_o);}
  s79 -> s241 [order 2] : R1r {send(R1r_o);}
  s79 -> s131 [order 3] : R1u {send(R1u_o);}
  s79 -> s131 [order 4] : R1ureq {send(R1ureq_o);}
  s79 -> s85 [order 5] : R2u {send(R2u_o);}
  s79 -> s80 [order 7] : R3u {send(R3u_o);}
  s81 -> s80 [order 7] : R3d {send(R3d_o);}
  s82 -> s80 [order 6] : R3l {send(R3l_o);}
  s86 -> s80 [order 4] : R2d {send(R2d_o);}
  s132 -> s80 [order 1] : R1d {send(R1d_o);}
  s80 -> s132 [order 2] : R1u {send(R1u_o);}
  s80 -> s132 [order 3] : R1ureq {send(R1ureq_o);}
  s80 -> s86 [order 5] : R2u {send(R2u_o);}
  s80 -> s82 [order 7] : R3r {send(R3r_o);}
  s80 -> s81 [order 8] : R3u {send(R3u_o);}
  s83 -> s81 [order 8] : R3l {send(R3l_o);}
  s87 -> s81 [order 5] : R2d {send(R2d_o);}
  s133 -> s81 [order 1] : R1d {send(R1d_o);}
  s242 -> s81 [order 2] : R1l {send(R1l_o);}
  s81 -> s242 [order 2] : R1r {send(R1r_o);}
  s81 -> s133 [order 3] : R1u {send(R1u_o);}
  s81 -> s133 [order 4] : R1ureq {send(R1ureq_o);}
  s81 -> s87 [order 6] : R2u {send(R2u_o);}
  s81 -> s83 [order 8] : R3r {send(R3r_o);}
  s83 -> s82 [order 7] : R3d {send(R3d_o);}
  s134 -> s82 [order 1] : R1d {send(R1d_o);}
  s243 -> s82 [order 2] : R1l {send(R1l_o);}
  s82 -> s243 [order 2] : R1r {send(R1r_o);}
  s82 -> s134 [order 3] : R1u {send(R1u_o);}
  s82 -> s134 [order 4] : R1ureq {send(R1ureq_o);}
  s82 -> s83 [order 7] : R3u {send(R3u_o);}
  s82 -> s83 [order 8] : R3ureq {send(R3ureq_o);}
  s89 -> s83 [order 5] : R2d {send(R2d_o);}
  s135 -> s83 [order 1] : R1d {send(R1d_o);}
  s244 -> s83 [order 2] : R1l {send(R1l_o);}
  s83 -> s244 [order 2] : R1r {send(R1r_o);}
  s83 -> s135 [order 3] : R1u {send(R1u_o);}
  s83 -> s135 [order 4] : R1ureq {send(R1ureq_o);}
  s83 -> s89 [order 6] : R2u {send(R2u_o);}
  s85 -> s84 [order 8] : R3l {send(R3l_o);}
  s90 -> s84 [order 4] : R2d {send(R2d_o);}
  s136 -> s84 [order 1] : R1d {send(R1d_o);}
  s245 -> s84 [order 2] : R1l {send(R1l_o);}
  s84 -> s245 [order 1] : R1r {send(R1r_o);}
  s84 -> s136 [order 2] : R1u {send(R1u_o);}
  s84 -> s136 [order 3] : R1ureq {send(R1ureq_o);}
  s84 -> s90 [order 6] : R2u {send(R2u_o);}
  s84 -> s85 [order 7] : R3r {send(R3r_o);}
  s86 -> s85 [order 6] : R3d {send(R3d_o);}
  s88 -> s85 [order 7] : R3l {send(R3l_o);}
  s91 -> s85 [order 5] : R2d {send(R2d_o);}
  s138 -> s85 [order 1] : R1d {send(R1d_o);}
  s248 -> s85 [order 1] : R1l {send(R1l_o);}
  s85 -> s248 [order 2] : R1r {send(R1r_o);}
  s85 -> s138 [order 3] : R1u {send(R1u_o);}
  s85 -> s138 [order 4] : R1ureq {send(R1ureq_o);}
  s85 -> s91 [order 7] : R2u {send(R2u_o);}
  s85 -> s88 [order 9] : R3r {send(R3r_o);}
  s85 -> s86 [order 10] : R3u {send(R3u_o);}
  s87 -> s86 [order 7] : R3d {send(R3d_o);}
  s92 -> s86 [order 4] : R2d {send(R2d_o);}
  s139 -> s86 [order 1] : R1d {send(R1d_o);}
  s86 -> s139 [order 2] : R1u {send(R1u_o);}
  s86 -> s139 [order 3] : R1ureq {send(R1ureq_o);}
  s86 -> s92 [order 5] : R2u {send(R2u_o);}
  s86 -> s87 [order 7] : R3u {send(R3u_o);}
  s89 -> s87 [order 7] : R3l {send(R3l_o);}
  s93 -> s87 [order 5] : R2d {send(R2d_o);}
  s140 -> s87 [order 1] : R1d {send(R1d_o);}
  s249 -> s87 [order 2] : R1l {send(R1l_o);}
  s87 -> s249 [order 2] : R1r {send(R1r_o);}
  s87 -> s140 [order 3] : R1u {send(R1u_o);}
  s87 -> s140 [order 4] : R1ureq {send(R1ureq_o);}
  s87 -> s93 [order 6] : R2u {send(R2u_o);}
  s87 -> s89 [order 8] : R3r {send(R3r_o);}
  s94 -> s88 [order 5] : R2d {send(R2d_o);}
  s141 -> s88 [order 1] : R1d {send(R1d_o);}
  s250 -> s88 [order 2] : R1l {send(R1l_o);}
  s88 -> s250 [order 2] : R1r {send(R1r_o);}
  s88 -> s141 [order 3] : R1u {send(R1u_o);}
  s88 -> s141 [order 4] : R1ureq {send(R1ureq_o);}
  s88 -> s94 [order 6] : R2u {send(R2u_o);}
  s142 -> s89 [order 1] : R1d {send(R1d_o);}
  s251 -> s89 [order 2] : R1l {send(R1l_o);}
  s89 -> s251 [order 2] : R1r {send(R1r_o);}
  s89 -> s142 [order 3] : R1u {send(R1u_o);}
  s89 -> s142 [order 4] : R1ureq {send(R1ureq_o);}
  s91 -> s90 [order 7] : R3l {send(R3l_o);}
  s143 -> s90 [order 1] : R1d {send(R1d_o);}
  s252 -> s90 [order 2] : R1l {send(R1l_o);}
  s90 -> s252 [order 1] : R1r {send(R1r_o);}
  s90 -> s143 [order 2] : R1u {send(R1u_o);}
  s90 -> s143 [order 3] : R1ureq {send(R1ureq_o);}
  s90 -> s91 [order 6] : R3r {send(R3r_o);}
  s92 -> s91 [order 6] : R3d {send(R3d_o);}
  s94 -> s91 [order 7] : R3l {send(R3l_o);}
  s145 -> s91 [order 1] : R1d {send(R1d_o);}
  s255 -> s91 [order 1] : R1l {send(R1l_o);}
  s91 -> s255 [order 2] : R1r {send(R1r_o);}
  s91 -> s145 [order 3] : R1u {send(R1u_o);}
  s91 -> s145 [order 4] : R1ureq {send(R1ureq_o);}
  s91 -> s94 [order 8] : R3r {send(R3r_o);}
  s91 -> s92 [order 9] : R3u {send(R3u_o);}
  s93 -> s92 [order 6] : R3d {send(R3d_o);}
  s146 -> s92 [order 1] : R1d {send(R1d_o);}
  s92 -> s146 [order 2] : R1u {send(R1u_o);}
  s92 -> s146 [order 3] : R1ureq {send(R1ureq_o);}
  s92 -> s93 [order 7] : R3u {send(R3u_o);}
  s147 -> s93 [order 1] : R1d {send(R1d_o);}
  s256 -> s93 [order 2] : R1l {send(R1l_o);}
  s93 -> s256 [order 2] : R1r {send(R1r_o);}
  s93 -> s147 [order 3] : R1u {send(R1u_o);}
  s93 -> s147 [order 4] : R1ureq {send(R1ureq_o);}
  s148 -> s94 [order 1] : R1d {send(R1d_o);}
  s257 -> s94 [order 2] : R1l {send(R1l_o);}
  s94 -> s257 [order 2] : R1r {send(R1r_o);}
  s94 -> s148 [order 3] : R1u {send(R1u_o);}
  s94 -> s148 [order 4] : R1ureq {send(R1ureq_o);}
  s97 -> s95 [order 6] : R3l {send(R3l_o);}
  s110 -> s95 [order 2] : R2l {send(R2l_o);}
  s258 -> s95 [order 2] : R1l {send(R1l_o);}
  s95 -> s258 [order 1] : R1r {send(R1r_o);}
  s95 -> s110 [order 2] : R2r {send(R2r_o);}
  s95 -> s97 [order 3] : R3r {send(R3r_o);}
  s97 -> s96 [order 5] : R3d {send(R3d_o);}
  s99 -> s96 [order 5] : R3l {send(R3l_o);}
  s103 -> s96 [order 2] : R2d {send(R2d_o);}
  s260 -> s96 [order 2] : R1l {send(R1l_o);}
  s96 -> s260 [order 2] : R1r {send(R1r_o);}
  s96 -> s103 [order 3] : R2u {send(R2u_o);}
  s96 -> s99 [order 4] : R3r {send(R3r_o);}
  s96 -> s97 [order 5] : R3u {send(R3u_o);}
  s98 -> s97 [order 4] : R3d {send(R3d_o);}
  s100 -> s97 [order 6] : R3l {send(R3l_o);}
  s104 -> s97 [order 2] : R2d {send(R2d_o);}
  s111 -> s97 [order 3] : R2l {send(R2l_o);}
  s261 -> s97 [order 1] : R1l {send(R1l_o);}
  s97 -> s261 [order 2] : R1r {send(R1r_o);}
  s97 -> s111 [order 3] : R2r {send(R2r_o);}
  s97 -> s104 [order 4] : R2u {send(R2u_o);}
  s97 -> s100 [order 7] : R3r {send(R3r_o);}
  s97 -> s98 [order 8] : R3u {send(R3u_o);}
  s101 -> s98 [order 6] : R3l {send(R3l_o);}
  s105 -> s98 [order 1] : R2d {send(R2d_o);}
  s112 -> s98 [order 2] : R2l {send(R2l_o);}
  s98 -> s112 [order 2] : R2r {send(R2r_o);}
  s98 -> s105 [order 3] : R2u {send(R2u_o);}
  s98 -> s101 [order 5] : R3r {send(R3r_o);}
  s100 -> s99 [order 5] : R3d {send(R3d_o);}
  s106 -> s99 [order 2] : R2d {send(R2d_o);}
  s113 -> s99 [order 3] : R2l {send(R2l_o);}
  s262 -> s99 [order 2] : R1l {send(R1l_o);}
  s99 -> s262 [order 2] : R1r {send(R1r_o);}
  s99 -> s113 [order 3] : R2r {send(R2r_o);}
  s99 -> s106 [order 4] : R2u {send(R2u_o);}
  s99 -> s100 [order 6] : R3u {send(R3u_o);}
  s101 -> s100 [order 5] : R3d {send(R3d_o);}
  s107 -> s100 [order 2] : R2d {send(R2d_o);}
  s114 -> s100 [order 3] : R2l {send(R2l_o);}
  s263 -> s100 [order 2] : R1l {send(R1l_o);}
  s100 -> s263 [order 2] : R1r {send(R1r_o);}
  s100 -> s114 [order 3] : R2r {send(R2r_o);}
  s100 -> s107 [order 4] : R2u {send(R2u_o);}
  s100 -> s101 [order 7] : R3u {send(R3u_o);}
  s100 -> s101 [order 8] : R3ureq {send(R3ureq_o);}
  s108 -> s101 [order 2] : R2d {send(R2d_o);}
  s115 -> s101 [order 3] : R2l {send(R2l_o);}
  s264 -> s101 [order 2] : R1l {send(R1l_o);}
  s101 -> s264 [order 2] : R1r {send(R1r_o);}
  s101 -> s115 [order 3] : R2r {send(R2r_o);}
  s101 -> s108 [order 4] : R2u {send(R2u_o);}
  s103 -> s102 [order 4] : R3l {send(R3l_o);}
  s116 -> s102 [order 3] : R2l {send(R2l_o);}
  s265 -> s102 [order 2] : R1l {send(R1l_o);}
  s102 -> s265 [order 1] : R1r {send(R1r_o);}
  s102 -> s116 [order 2] : R2r {send(R2r_o);}
  s102 -> s103 [order 3] : R3r {send(R3r_o);}
  s104 -> s103 [order 3] : R3d {send(R3d_o);}
  s106 -> s103 [order 4] : R3l {send(R3l_o);}
  s118 -> s103 [order 2] : R2l {send(R2l_o);}
  s267 -> s103 [order 2] : R1l {send(R1l_o);}
  s103 -> s267 [order 1] : R1r {send(R1r_o);}
  s103 -> s118 [order 3] : R2r {send(R2r_o);}
  s103 -> s106 [order 5] : R3r {send(R3r_o);}
  s103 -> s104 [order 6] : R3u {send(R3u_o);}
  s105 -> s104 [order 2] : R3d {send(R3d_o);}
  s107 -> s104 [order 5] : R3l {send(R3l_o);}
  s268 -> s104 [order 1] : R1l {send(R1l_o);}
  s104 -> s268 [order 1] : R1r {send(R1r_o);}
  s104 -> s107 [order 4] : R3r {send(R3r_o);}
  s104 -> s105 [order 5] : R3u {send(R3u_o);}
  s108 -> s105 [order 5] : R3l {send(R3l_o);}
  s105 -> s108 [order 3] : R3r {send(R3r_o);}
  s107 -> s106 [order 4] : R3d {send(R3d_o);}
  s119 -> s106 [order 3] : R2l {send(R2l_o);}
  s269 -> s106 [order 2] : R1l {send(R1l_o);}
  s106 -> s269 [order 1] : R1r {send(R1r_o);}
  s106 -> s119 [order 3] : R2r {send(R2r_o);}
  s106 -> s107 [order 5] : R3u {send(R3u_o);}
  s108 -> s107 [order 4] : R3d {send(R3d_o);}
  s120 -> s107 [order 3] : R2l {send(R2l_o);}
  s270 -> s107 [order 2] : R1l {send(R1l_o);}
  s107 -> s270 [order 1] : R1r {send(R1r_o);}
  s107 -> s120 [order 3] : R2r {send(R2r_o);}
  s107 -> s108 [order 6] : R3u {send(R3u_o);}
  s107 -> s108 [order 7] : R3ureq {send(R3ureq_o);}
  s121 -> s108 [order 3] : R2l {send(R2l_o);}
  s271 -> s108 [order 2] : R1l {send(R1l_o);}
  s108 -> s271 [order 1] : R1r {send(R1r_o);}
  s108 -> s121 [order 3] : R2r {send(R2r_o);}
  s110 -> s109 [order 5] : R3d {send(R3d_o);}
  s116 -> s109 [order 2] : R2d {send(R2d_o);}
  s129 -> s109 [order 3] : R2l {send(R2l_o);}
  s279 -> s109 [order 2] : R1l {send(R1l_o);}
  s109 -> s279 [order 2] : R1r {send(R1r_o);}
  s109 -> s129 [order 3] : R2r {send(R2r_o);}
  s109 -> s116 [order 4] : R2u {send(R2u_o);}
  s109 -> s110 [order 5] : R3u {send(R3u_o);}
  s111 -> s110 [order 5] : R3l {send(R3l_o);}
  s117 -> s110 [order 1] : R2d {send(R2d_o);}
  s130 -> s110 [order 2] : R2l {send(R2l_o);}
  s280 -> s110 [order 2] : R1l {send(R1l_o);}
  s110 -> s280 [order 1] : R1r {send(R1r_o);}
  s110 -> s130 [order 3] : R2r {send(R2r_o);}
  s110 -> s117 [order 4] : R2u {send(R2u_o);}
  s110 -> s111 [order 6] : R3r {send(R3r_o);}
  s112 -> s111 [order 4] : R3d {send(R3d_o);}
  s114 -> s111 [order 7] : R3l {send(R3l_o);}
  s132 -> s111 [order 3] : R2l {send(R2l_o);}
  s282 -> s111 [order 1] : R1l {send(R1l_o);}
  s111 -> s282 [order 2] : R1r {send(R1r_o);}
  s111 -> s132 [order 4] : R2r {send(R2r_o);}
  s111 -> s114 [order 6] : R3r {send(R3r_o);}
  s111 -> s112 [order 7] : R3u {send(R3u_o);}
  s115 -> s112 [order 7] : R3l {send(R3l_o);}
  s133 -> s112 [order 2] : R2l {send(R2l_o);}
  s112 -> s133 [order 3] : R2r {send(R2r_o);}
  s112 -> s115 [order 5] : R3r {send(R3r_o);}
  s114 -> s113 [order 6] : R3d {send(R3d_o);}
  s119 -> s113 [order 2] : R2d {send(R2d_o);}
  s283 -> s113 [order 2] : R1l {send(R1l_o);}
  s113 -> s283 [order 2] : R1r {send(R1r_o);}
  s113 -> s119 [order 4] : R2u {send(R2u_o);}
  s113 -> s114 [order 5] : R3u {send(R3u_o);}
  s115 -> s114 [order 6] : R3d {send(R3d_o);}
  s120 -> s114 [order 2] : R2d {send(R2d_o);}
  s134 -> s114 [order 3] : R2l {send(R2l_o);}
  s284 -> s114 [order 2] : R1l {send(R1l_o);}
  s114 -> s284 [order 2] : R1r {send(R1r_o);}
  s114 -> s134 [order 4] : R2r {send(R2r_o);}
  s114 -> s120 [order 5] : R2u {send(R2u_o);}
  s114 -> s115 [order 8] : R3u {send(R3u_o);}
  s114 -> s115 [order 9] : R3ureq {send(R3ureq_o);}
  s121 -> s115 [order 2] : R2d {send(R2d_o);}
  s135 -> s115 [order 3] : R2l {send(R2l_o);}
  s285 -> s115 [order 2] : R1l {send(R1l_o);}
  s115 -> s285 [order 2] : R1r {send(R1r_o);}
  s115 -> s135 [order 4] : R2r {send(R2r_o);}
  s115 -> s121 [order 5] : R2u {send(R2u_o);}
  s117 -> s116 [order 5] : R3d {send(R3d_o);}
  s118 -> s116 [order 6] : R3l {send(R3l_o);}
  s122 -> s116 [order 2] : R2d {send(R2d_o);}
  s136 -> s116 [order 4] : R2l {send(R2l_o);}
  s116 -> s136 [order 4] : R2r {send(R2r_o);}
  s116 -> s122 [order 5] : R2u {send(R2u_o);}
  s116 -> s122 [order 6] : R2ureq {send(R2ureq_o);}
  s116 -> s118 [order 7] : R3r {send(R3r_o);}
  s116 -> s117 [order 8] : R3u {send(R3u_o);}
  s123 -> s117 [order 1] : R2d {send(R2d_o);}
  s137 -> s117 [order 3] : R2l {send(R2l_o);}
  s117 -> s137 [order 2] : R2r {send(R2r_o);}
  s117 -> s123 [order 3] : R2u {send(R2u_o);}
  s117 -> s123 [order 4] : R2ureq {send(R2ureq_o);}
  s119 -> s118 [order 7] : R3l {send(R3l_o);}
  s124 -> s118 [order 2] : R2d {send(R2d_o);}
  s138 -> s118 [order 4] : R2l {send(R2l_o);}
  s118 -> s138 [order 3] : R2r {send(R2r_o);}
  s118 -> s124 [order 4] : R2u {send(R2u_o);}
  s118 -> s124 [order 5] : R2ureq {send(R2ureq_o);}
  s118 -> s119 [order 7] : R3r {send(R3r_o);}
  s120 -> s119 [order 6] : R3d {send(R3d_o);}
  s126 -> s119 [order 2] : R2d {send(R2d_o);}
  s141 -> s119 [order 3] : R2l {send(R2l_o);}
  s119 -> s141 [order 4] : R2r {send(R2r_o);}
  s119 -> s126 [order 5] : R2u {send(R2u_o);}
  s119 -> s126 [order 6] : R2ureq {send(R2ureq_o);}
  s119 -> s120 [order 8] : R3u {send(R3u_o);}
  s121 -> s120 [order 7] : R3d {send(R3d_o);}
  s127 -> s120 [order 2] : R2d {send(R2d_o);}
  s120 -> s127 [order 4] : R2u {send(R2u_o);}
  s120 -> s127 [order 5] : R2ureq {send(R2ureq_o);}
  s120 -> s121 [order 7] : R3u {send(R3u_o);}
  s120 -> s121 [order 8] : R3ureq {send(R3ureq_o);}
  s128 -> s121 [order 2] : R2d {send(R2d_o);}
  s142 -> s121 [order 4] : R2l {send(R2l_o);}
  s121 -> s142 [order 4] : R2r {send(R2r_o);}
  s121 -> s128 [order 5] : R2u {send(R2u_o);}
  s121 -> s128 [order 6] : R2ureq {send(R2ureq_o);}
  s123 -> s122 [order 3] : R3d {send(R3d_o);}
  s124 -> s122 [order 4] : R3l {send(R3l_o);}
  s143 -> s122 [order 4] : R2l {send(R2l_o);}
  s122 -> s143 [order 3] : R2r {send(R2r_o);}
  s122 -> s124 [order 4] : R3r {send(R3r_o);}
  s122 -> s123 [order 5] : R3u {send(R3u_o);}
  s125 -> s123 [order 4] : R3l {send(R3l_o);}
  s144 -> s123 [order 3] : R2l {send(R2l_o);}
  s123 -> s144 [order 2] : R2r {send(R2r_o);}
  s123 -> s125 [order 4] : R3r {send(R3r_o);}
  s125 -> s124 [order 3] : R3d {send(R3d_o);}
  s126 -> s124 [order 4] : R3l {send(R3l_o);}
  s145 -> s124 [order 4] : R2l {send(R2l_o);}
  s124 -> s145 [order 3] : R2r {send(R2r_o);}
  s124 -> s126 [order 5] : R3r {send(R3r_o);}
  s124 -> s125 [order 6] : R3u {send(R3u_o);}
  s127 -> s125 [order 4] : R3l {send(R3l_o);}
  s146 -> s125 [order 4] : R2l {send(R2l_o);}
  s125 -> s146 [order 2] : R2r {send(R2r_o);}
  s125 -> s127 [order 5] : R3r {send(R3r_o);}
  s127 -> s126 [order 3] : R3d {send(R3d_o);}
  s148 -> s126 [order 4] : R2l {send(R2l_o);}
  s126 -> s148 [order 3] : R2r {send(R2r_o);}
  s126 -> s127 [order 5] : R3u {send(R3u_o);}
  s128 -> s127 [order 3] : R3d {send(R3d_o);}
  s127 -> s128 [order 5] : R3u {send(R3u_o);}
  s127 -> s128 [order 6] : R3ureq {send(R3ureq_o);}
  s130 -> s129 [order 4] : R3d {send(R3d_o);}
  s131 -> s129 [order 4] : R3l {send(R3l_o);}
  s136 -> s129 [order 3] : R2d {send(R2d_o);}
  s286 -> s129 [order 2] : R1l {send(R1l_o);}
  s129 -> s286 [order 2] : R1r {send(R1r_o);}
  s129 -> s136 [order 4] : R2u {send(R2u_o);}
  s129 -> s131 [order 5] : R3r {send(R3r_o);}
  s129 -> s130 [order 6] : R3u {send(R3u_o);}
  s132 -> s130 [order 6] : R3l {send(R3l_o);}
  s137 -> s130 [order 2] : R2d {send(R2d_o);}
  s287 -> s130 [order 2] : R1l {send(R1l_o);}
  s130 -> s287 [order 1] : R1r {send(R1r_o);}
  s130 -> s137 [order 3] : R2u {send(R2u_o);}
  s130 -> s132 [order 5] : R3r {send(R3r_o);}
  s132 -> s131 [order 5] : R3d {send(R3d_o);}
  s138 -> s131 [order 3] : R2d {send(R2d_o);}
  s289 -> s131 [order 2] : R1l {send(R1l_o);}
  s131 -> s289 [order 2] : R1r {send(R1r_o);}
  s131 -> s138 [order 3] : R2u {send(R2u_o);}
  s131 -> s132 [order 5] : R3u {send(R3u_o);}
  s133 -> s132 [order 4] : R3d {send(R3d_o);}
  s134 -> s132 [order 4] : R3l {send(R3l_o);}
  s139 -> s132 [order 3] : R2d {send(R2d_o);}
  s290 -> s132 [order 1] : R1l {send(R1l_o);}
  s132 -> s290 [order 2] : R1r {send(R1r_o);}
  s132 -> s139 [order 4] : R2u {send(R2u_o);}
  s132 -> s134 [order 7] : R3r {send(R3r_o);}
  s132 -> s133 [order 8] : R3u {send(R3u_o);}
  s135 -> s133 [order 6] : R3l {send(R3l_o);}
  s140 -> s133 [order 2] : R2d {send(R2d_o);}
  s133 -> s140 [order 3] : R2u {send(R2u_o);}
  s133 -> s135 [order 5] : R3r {send(R3r_o);}
  s135 -> s134 [order 5] : R3d {send(R3d_o);}
  s291 -> s134 [order 2] : R1l {send(R1l_o);}
  s134 -> s291 [order 2] : R1r {send(R1r_o);}
  s134 -> s135 [order 5] : R3u {send(R3u_o);}
  s134 -> s135 [order 6] : R3ureq {send(R3ureq_o);}
  s142 -> s135 [order 3] : R2d {send(R2d_o);}
  s292 -> s135 [order 2] : R1l {send(R1l_o);}
  s135 -> s292 [order 2] : R1r {send(R1r_o);}
  s135 -> s142 [order 4] : R2u {send(R2u_o);}
  s137 -> s136 [order 5] : R3d {send(R3d_o);}
  s138 -> s136 [order 6] : R3l {send(R3l_o);}
  s143 -> s136 [order 3] : R2d {send(R2d_o);}
  s293 -> s136 [order 2] : R1l {send(R1l_o);}
  s136 -> s293 [order 2] : R1r {send(R1r_o);}
  s136 -> s143 [order 5] : R2u {send(R2u_o);}
  s136 -> s138 [order 6] : R3r {send(R3r_o);}
  s136 -> s137 [order 7] : R3u {send(R3u_o);}
  s139 -> s137 [order 6] : R3l {send(R3l_o);}
  s144 -> s137 [order 2] : R2d {send(R2d_o);}
  s294 -> s137 [order 2] : R1l {send(R1l_o);}
  s137 -> s294 [order 1] : R1r {send(R1r_o);}
  s137 -> s144 [order 4] : R2u {send(R2u_o);}
  s137 -> s139 [order 6] : R3r {send(R3r_o);}
  s139 -> s138 [order 5] : R3d {send(R3d_o);}
  s141 -> s138 [order 5] : R3l {send(R3l_o);}
  s145 -> s138 [order 3] : R2d {send(R2d_o);}
  s296 -> s138 [order 2] : R1l {send(R1l_o);}
  s138 -> s296 [order 2] : R1r {send(R1r_o);}
  s138 -> s145 [order 5] : R2u {send(R2u_o);}
  s138 -> s141 [order 7] : R3r {send(R3r_o);}
  s138 -> s139 [order 8] : R3u {send(R3u_o);}
  s140 -> s139 [order 4] : R3d {send(R3d_o);}
  s146 -> s139 [order 3] : R2d {send(R2d_o);}
  s297 -> s139 [order 1] : R1l {send(R1l_o);}
  s139 -> s297 [order 2] : R1r {send(R1r_o);}
  s139 -> s146 [order 4] : R2u {send(R2u_o);}
  s139 -> s140 [order 7] : R3u {send(R3u_o);}
  s142 -> s140 [order 5] : R3l {send(R3l_o);}
  s147 -> s140 [order 2] : R2d {send(R2d_o);}
  s140 -> s147 [order 3] : R2u {send(R2u_o);}
  s140 -> s142 [order 5] : R3r {send(R3r_o);}
  s148 -> s141 [order 3] : R2d {send(R2d_o);}
  s298 -> s141 [order 2] : R1l {send(R1l_o);}
  s141 -> s298 [order 2] : R1r {send(R1r_o);}
  s141 -> s148 [order 4] : R2u {send(R2u_o);}
  s299 -> s142 [order 2] : R1l {send(R1l_o);}
  s142 -> s299 [order 2] : R1r {send(R1r_o);}
  s144 -> s143 [order 4] : R3d {send(R3d_o);}
  s145 -> s143 [order 5] : R3l {send(R3l_o);}
  s300 -> s143 [order 2] : R1l {send(R1l_o);}
  s143 -> s300 [order 2] : R1r {send(R1r_o);}
  s143 -> s145 [order 5] : R3r {send(R3r_o);}
  s143 -> s144 [order 6] : R3u {send(R3u_o);}
  s146 -> s144 [order 6] : R3l {send(R3l_o);}
  s301 -> s144 [order 2] : R1l {send(R1l_o);}
  s144 -> s301 [order 1] : R1r {send(R1r_o);}
  s144 -> s146 [order 5] : R3r {send(R3r_o);}
  s146 -> s145 [order 5] : R3d {send(R3d_o);}
  s148 -> s145 [order 5] : R3l {send(R3l_o);}
  s303 -> s145 [order 2] : R1l {send(R1l_o);}
  s145 -> s303 [order 2] : R1r {send(R1r_o);}
  s145 -> s148 [order 6] : R3r {send(R3r_o);}
  s145 -> s146 [order 7] : R3u {send(R3u_o);}
  s147 -> s146 [order 3] : R3d {send(R3d_o);}
  s304 -> s146 [order 1] : R1l {send(R1l_o);}
  s146 -> s304 [order 2] : R1r {send(R1r_o);}
  s146 -> s147 [order 7] : R3u {send(R3u_o);}
  s305 -> s148 [order 2] : R1l {send(R1l_o);}
  s148 -> s305 [order 2] : R1r {send(R1r_o);}
  s150 -> s149 [order 4] : R3d {send(R3d_o);}
  s151 -> s149 [order 3] : R3l {send(R3l_o);}
  s203 -> s149 [order 1] : R1d {send(R1d_o);}
  s306 -> s149 [order 1] : R1l {send(R1l_o);}
  s149 -> s306 [order 1] : R1r {send(R1r_o);}
  s149 -> s203 [order 2] : R1u {send(R1u_o);}
  s149 -> s151 [order 3] : R3r {send(R3r_o);}
  s149 -> s150 [order 4] : R3u {send(R3u_o);}
  s152 -> s150 [order 5] : R3l {send(R3l_o);}
  s157 -> s150 [order 4] : R2d {send(R2d_o);}
  s204 -> s150 [order 1] : R1d {send(R1d_o);}
  s307 -> s150 [order 1] : R1l {send(R1l_o);}
  s150 -> s307 [order 1] : R1r {send(R1r_o);}
  s150 -> s204 [order 2] : R1u {send(R1u_o);}
  s150 -> s157 [order 3] : R2u {send(R2u_o);}
  s150 -> s152 [order 5] : R3r {send(R3r_o);}
  s152 -> s151 [order 4] : R3d {send(R3d_o);}
  s154 -> s151 [order 5] : R3l {send(R3l_o);}
  s158 -> s151 [order 3] : R2d {send(R2d_o);}
  s309 -> s151 [order 1] : R1l {send(R1l_o);}
  s151 -> s309 [order 1] : R1r {send(R1r_o);}
  s151 -> s158 [order 2] : R2u {send(R2u_o);}
  s151 -> s154 [order 4] : R3r {send(R3r_o);}
  s151 -> s152 [order 5] : R3u {send(R3u_o);}
  s155 -> s152 [order 5] : R3l {send(R3l_o);}
  s159 -> s152 [order 4] : R2d {send(R2d_o);}
  s206 -> s152 [order 1] : R1d {send(R1d_o);}
  s310 -> s152 [order 1] : R1l {send(R1l_o);}
  s152 -> s310 [order 1] : R1r {send(R1r_o);}
  s152 -> s206 [order 2] : R1u {send(R1u_o);}
  s152 -> s159 [order 3] : R2u {send(R2u_o);}
  s152 -> s155 [order 6] : R3r {send(R3r_o);}
  s154 -> s153 [order 4] : R3d {send(R3d_o);}
  s160 -> s153 [order 3] : R2d {send(R2d_o);}
  s207 -> s153 [order 1] : R1d {send(R1d_o);}
  s153 -> s207 [order 1] : R1u {send(R1u_o);}
  s153 -> s160 [order 2] : R2u {send(R2u_o);}
  s153 -> s154 [order 3] : R3u {send(R3u_o);}
  s155 -> s154 [order 4] : R3d {send(R3d_o);}
  s161 -> s154 [order 4] : R2d {send(R2d_o);}
  s208 -> s154 [order 1] : R1d {send(R1d_o);}
  s311 -> s154 [order 1] : R1l {send(R1l_o);}
  s154 -> s311 [order 1] : R1r {send(R1r_o);}
  s154 -> s208 [order 2] : R1u {send(R1u_o);}
  s154 -> s161 [order 3] : R2u {send(R2u_o);}
  s154 -> s155 [order 6] : R3u {send(R3u_o);}
  s154 -> s155 [order 7] : R3ureq {send(R3ureq_o);}
  s162 -> s155 [order 4] : R2d {send(R2d_o);}
  s209 -> s155 [order 1] : R1d {send(R1d_o);}
  s312 -> s155 [order 1] : R1l {send(R1l_o);}
  s155 -> s312 [order 1] : R1r {send(R1r_o);}
  s155 -> s209 [order 2] : R1u {send(R1u_o);}
  s155 -> s162 [order 3] : R2u {send(R2u_o);}
  s163 -> s156 [order 3] : R2d {send(R2d_o);}
  s170 -> s156 [order 2] : R2l {send(R2l_o);}
  s210 -> s156 [order 1] : R1d {send(R1d_o);}
  s313 -> s156 [order 1] : R1l {send(R1l_o);}
  s156 -> s313 [order 1] : R1r {send(R1r_o);}
  s156 -> s210 [order 2] : R1u {send(R1u_o);}
  s156 -> s170 [order 3] : R2r {send(R2r_o);}
  s156 -> s163 [order 4] : R2u {send(R2u_o);}
  s159 -> s157 [order 7] : R3l {send(R3l_o);}
  s172 -> s157 [order 3] : R2l {send(R2l_o);}
  s211 -> s157 [order 1] : R1d {send(R1d_o);}
  s314 -> s157 [order 1] : R1l {send(R1l_o);}
  s157 -> s314 [order 2] : R1r {send(R1r_o);}
  s157 -> s211 [order 3] : R1u {send(R1u_o);}
  s157 -> s172 [order 5] : R2r {send(R2r_o);}
  s157 -> s159 [order 6] : R3r {send(R3r_o);}
  s159 -> s158 [order 6] : R3d {send(R3d_o);}
  s161 -> s158 [order 8] : R3l {send(R3l_o);}
  s165 -> s158 [order 3] : R2d {send(R2d_o);}
  s316 -> s158 [order 1] : R1l {send(R1l_o);}
  s158 -> s316 [order 2] : R1r {send(R1r_o);}
  s158 -> s165 [order 4] : R2u {send(R2u_o);}
  s158 -> s161 [order 5] : R3r {send(R3r_o);}
  s158 -> s159 [order 6] : R3u {send(R3u_o);}
  s162 -> s159 [order 8] : R3l {send(R3l_o);}
  s166 -> s159 [order 4] : R2d {send(R2d_o);}
  s213 -> s159 [order 1] : R1d {send(R1d_o);}
  s317 -> s159 [order 1] : R1l {send(R1l_o);}
  s159 -> s317 [order 2] : R1r {send(R1r_o);}
  s159 -> s213 [order 3] : R1u {send(R1u_o);}
  s159 -> s166 [order 5] : R2u {send(R2u_o);}
  s159 -> s162 [order 8] : R3r {send(R3r_o);}
  s161 -> s160 [order 7] : R3d {send(R3d_o);}
  s167 -> s160 [order 3] : R2d {send(R2d_o);}
  s173 -> s160 [order 2] : R2l {send(R2l_o);}
  s214 -> s160 [order 1] : R1d {send(R1d_o);}
  s160 -> s214 [order 2] : R1u {send(R1u_o);}
  s160 -> s173 [order 4] : R2r {send(R2r_o);}
  s160 -> s167 [order 5] : R2u {send(R2u_o);}
  s160 -> s161 [order 6] : R3u {send(R3u_o);}
  s162 -> s161 [order 7] : R3d {send(R3d_o);}
  s168 -> s161 [order 4] : R2d {send(R2d_o);}
  s174 -> s161 [order 3] : R2l {send(R2l_o);}
  s215 -> s161 [order 1] : R1d {send(R1d_o);}
  s318 -> s161 [order 1] : R1l {send(R1l_o);}
  s161 -> s318 [order 2] : R1r {send(R1r_o);}
  s161 -> s215 [order 3] : R1u {send(R1u_o);}
  s161 -> s174 [order 5] : R2r {send(R2r_o);}
  s161 -> s168 [order 6] : R2u {send(R2u_o);}
  s161 -> s162 [order 9] : R3u {send(R3u_o);}
  s161 -> s162 [order 10] : R3ureq {send(R3ureq_o);}
  s169 -> s162 [order 4] : R2d {send(R2d_o);}
  s175 -> s162 [order 3] : R2l {send(R2l_o);}
  s216 -> s162 [order 1] : R1d {send(R1d_o);}
  s319 -> s162 [order 1] : R1l {send(R1l_o);}
  s162 -> s319 [order 2] : R1r {send(R1r_o);}
  s162 -> s216 [order 3] : R1u {send(R1u_o);}
  s162 -> s175 [order 5] : R2r {send(R2r_o);}
  s162 -> s169 [order 6] : R2u {send(R2u_o);}
  s164 -> s163 [order 5] : R3d {send(R3d_o);}
  s176 -> s163 [order 4] : R2l {send(R2l_o);}
  s217 -> s163 [order 1] : R1d {send(R1d_o);}
  s320 -> s163 [order 1] : R1l {send(R1l_o);}
  s163 -> s320 [order 1] : R1r {send(R1r_o);}
  s163 -> s217 [order 2] : R1u {send(R1u_o);}
  s163 -> s176 [order 4] : R2r {send(R2r_o);}
  s163 -> s164 [order 5] : R3u {send(R3u_o);}
  s165 -> s164 [order 5] : R3l {send(R3l_o);}
  s177 -> s164 [order 5] : R2l {send(R2l_o);}
  s218 -> s164 [order 1] : R1d {send(R1d_o);}
  s321 -> s164 [order 1] : R1l {send(R1l_o);}
  s164 -> s321 [order 2] : R1r {send(R1r_o);}
  s164 -> s218 [order 3] : R1u {send(R1u_o);}
  s164 -> s177 [order 4] : R2r {send(R2r_o);}
  s164 -> s165 [order 6] : R3r {send(R3r_o);}
  s166 -> s165 [order 5] : R3d {send(R3d_o);}
  s168 -> s165 [order 7] : R3l {send(R3l_o);}
  s179 -> s165 [order 3] : R2l {send(R2l_o);}
  s323 -> s165 [order 1] : R1l {send(R1l_o);}
  s165 -> s323 [order 2] : R1r {send(R1r_o);}
  s165 -> s179 [order 4] : R2r {send(R2r_o);}
  s165 -> s168 [order 6] : R3r {send(R3r_o);}
  s165 -> s166 [order 7] : R3u {send(R3u_o);}
  s169 -> s166 [order 7] : R3l {send(R3l_o);}
  s220 -> s166 [order 1] : R1d {send(R1d_o);}
  s324 -> s166 [order 1] : R1l {send(R1l_o);}
  s166 -> s324 [order 2] : R1r {send(R1r_o);}
  s166 -> s220 [order 3] : R1u {send(R1u_o);}
  s166 -> s169 [order 6] : R3r {send(R3r_o);}
  s168 -> s167 [order 6] : R3d {send(R3d_o);}
  s180 -> s167 [order 4] : R2l {send(R2l_o);}
  s221 -> s167 [order 1] : R1d {send(R1d_o);}
  s167 -> s221 [order 2] : R1u {send(R1u_o);}
  s167 -> s180 [order 4] : R2r {send(R2r_o);}
  s167 -> s168 [order 5] : R3u {send(R3u_o);}
  s169 -> s168 [order 6] : R3d {send(R3d_o);}
  s181 -> s168 [order 5] : R2l {send(R2l_o);}
  s222 -> s168 [order 1] : R1d {send(R1d_o);}
  s325 -> s168 [order 1] : R1l {send(R1l_o);}
  s168 -> s325 [order 2] : R1r {send(R1r_o);}
  s168 -> s222 [order 3] : R1u {send(R1u_o);}
  s168 -> s181 [order 5] : R2r {send(R2r_o);}
  s168 -> s169 [order 8] : R3u {send(R3u_o);}
  s168 -> s169 [order 9] : R3ureq {send(R3ureq_o);}
  s182 -> s169 [order 5] : R2l {send(R2l_o);}
  s223 -> s169 [order 1] : R1d {send(R1d_o);}
  s326 -> s169 [order 1] : R1l {send(R1l_o);}
  s169 -> s326 [order 2] : R1r {send(R1r_o);}
  s169 -> s223 [order 3] : R1u {send(R1u_o);}
  s169 -> s182 [order 5] : R2r {send(R2r_o);}
  s171 -> s170 [order 6] : R3d {send(R3d_o);}
  s176 -> s170 [order 3] : R2d {send(R2d_o);}
  s190 -> s170 [order 4] : R2l {send(R2l_o);}
  s334 -> s170 [order 1] : R1l {send(R1l_o);}
  s170 -> s334 [order 1] : R1r {send(R1r_o);}
  s170 -> s190 [order 3] : R2r {send(R2r_o);}
  s170 -> s176 [order 4] : R2u {send(R2u_o);}
  s170 -> s176 [order 5] : R2ureq {send(R2ureq_o);}
  s170 -> s171 [order 6] : R3u {send(R3u_o);}
  s172 -> s171 [order 7] : R3d {send(R3d_o);}
  s177 -> s171 [order 4] : R2d {send(R2d_o);}
  s191 -> s171 [order 5] : R2l {send(R2l_o);}
  s335 -> s171 [order 1] : R1l {send(R1l_o);}
  s171 -> s335 [order 2] : R1r {send(R1r_o);}
  s171 -> s191 [order 3] : R2r {send(R2r_o);}
  s171 -> s177 [order 4] : R2u {send(R2u_o);}
  s171 -> s177 [order 5] : R2ureq {send(R2ureq_o);}
  s171 -> s172 [order 7] : R3u {send(R3u_o);}
  s178 -> s172 [order 4] : R2d {send(R2d_o);}
  s192 -> s172 [order 5] : R2l {send(R2l_o);}
  s336 -> s172 [order 1] : R1l {send(R1l_o);}
  s172 -> s336 [order 2] : R1r {send(R1r_o);}
  s172 -> s192 [order 4] : R2r {send(R2r_o);}
  s172 -> s178 [order 5] : R2u {send(R2u_o);}
  s172 -> s178 [order 6] : R2ureq {send(R2ureq_o);}
  s174 -> s173 [order 6] : R3d {send(R3d_o);}
  s180 -> s173 [order 3] : R2d {send(R2d_o);}
  s195 -> s173 [order 3] : R2l {send(R2l_o);}
  s173 -> s195 [order 3] : R2r {send(R2r_o);}
  s173 -> s180 [order 4] : R2u {send(R2u_o);}
  s173 -> s180 [order 5] : R2ureq {send(R2ureq_o);}
  s173 -> s174 [order 6] : R3u {send(R3u_o);}
  s175 -> s174 [order 7] : R3d {send(R3d_o);}
  s181 -> s174 [order 4] : R2d {send(R2d_o);}
  s338 -> s174 [order 1] : R1l {send(R1l_o);}
  s174 -> s338 [order 2] : R1r {send(R1r_o);}
  s174 -> s181 [order 4] : R2u {send(R2u_o);}
  s174 -> s181 [order 5] : R2ureq {send(R2ureq_o);}
  s174 -> s175 [order 7] : R3u {send(R3u_o);}
  s174 -> s175 [order 8] : R3ureq {send(R3ureq_o);}
  s182 -> s175 [order 4] : R2d {send(R2d_o);}
  s196 -> s175 [order 5] : R2l {send(R2l_o);}
  s339 -> s175 [order 1] : R1l {send(R1l_o);}
  s175 -> s339 [order 2] : R1r {send(R1r_o);}
  s175 -> s196 [order 4] : R2r {send(R2r_o);}
  s175 -> s182 [order 5] : R2u {send(R2u_o);}
  s175 -> s182 [order 6] : R2ureq {send(R2ureq_o);}
  s177 -> s176 [order 7] : R3d {send(R3d_o);}
  s197 -> s176 [order 4] : R2l {send(R2l_o);}
  s231 -> s176 [order 1] : R1d {send(R1d_o);}
  s340 -> s176 [order 1] : R1l {send(R1l_o);}
  s176 -> s340 [order 1] : R1r {send(R1r_o);}
  s176 -> s231 [order 2] : R1u {send(R1u_o);}
  s176 -> s197 [order 5] : R2r {send(R2r_o);}
  s176 -> s177 [order 6] : R3u {send(R3u_o);}
  s178 -> s177 [order 6] : R3d {send(R3d_o);}
  s179 -> s177 [order 5] : R3l {send(R3l_o);}
  s198 -> s177 [order 5] : R2l {send(R2l_o);}
  s232 -> s177 [order 1] : R1d {send(R1d_o);}
  s341 -> s177 [order 1] : R1l {send(R1l_o);}
  s177 -> s341 [order 2] : R1r {send(R1r_o);}
  s177 -> s232 [order 3] : R1u {send(R1u_o);}
  s177 -> s198 [order 6] : R2r {send(R2r_o);}
  s177 -> s179 [order 8] : R3r {send(R3r_o);}
  s177 -> s178 [order 9] : R3u {send(R3u_o);}
  s199 -> s178 [order 5] : R2l {send(R2l_o);}
  s233 -> s178 [order 1] : R1d {send(R1d_o);}
  s342 -> s178 [order 1] : R1l {send(R1l_o);}
  s178 -> s342 [order 2] : R1r {send(R1r_o);}
  s178 -> s233 [order 3] : R1u {send(R1u_o);}
  s178 -> s199 [order 5] : R2r {send(R2r_o);}
  s181 -> s179 [order 7] : R3l {send(R3l_o);}
  s200 -> s179 [order 4] : R2l {send(R2l_o);}
  s344 -> s179 [order 1] : R1l {send(R1l_o);}
  s179 -> s344 [order 2] : R1r {send(R1r_o);}
  s179 -> s200 [order 4] : R2r {send(R2r_o);}
  s179 -> s181 [order 6] : R3r {send(R3r_o);}
  s181 -> s180 [order 6] : R3d {send(R3d_o);}
  s202 -> s180 [order 4] : R2l {send(R2l_o);}
  s235 -> s180 [order 1] : R1d {send(R1d_o);}
  s180 -> s235 [order 2] : R1u {send(R1u_o);}
  s180 -> s202 [order 5] : R2r {send(R2r_o);}
  s180 -> s181 [order 6] : R3u {send(R3u_o);}
  s182 -> s181 [order 6] : R3d {send(R3d_o);}
  s236 -> s181 [order 1] : R1d {send(R1d_o);}
  s345 -> s181 [order 1] : R1l {send(R1l_o);}
  s181 -> s345 [order 2] : R1r {send(R1r_o);}
  s181 -> s236 [order 3] : R1u {send(R1u_o);}
  s181 -> s182 [order 8] : R3u {send(R3u_o);}
  s181 -> s182 [order 9] : R3ureq {send(R3ureq_o);}
  s237 -> s182 [order 1] : R1d {send(R1d_o);}
  s346 -> s182 [order 1] : R1l {send(R1l_o);}
  s182 -> s346 [order 2] : R1r {send(R1r_o);}
  s182 -> s237 [order 3] : R1u {send(R1u_o);}
  s184 -> s183 [order 4] : R3d {send(R3d_o);}
  s190 -> s183 [order 3] : R2d {send(R2d_o);}
  s238 -> s183 [order 1] : R1d {send(R1d_o);}
  s183 -> s238 [order 1] : R1u {send(R1u_o);}
  s183 -> s190 [order 2] : R2u {send(R2u_o);}
  s183 -> s184 [order 3] : R3u {send(R3u_o);}
  s185 -> s184 [order 4] : R3d {send(R3d_o);}
  s186 -> s184 [order 3] : R3l {send(R3l_o);}
  s191 -> s184 [order 4] : R2d {send(R2d_o);}
  s239 -> s184 [order 1] : R1d {send(R1d_o);}
  s184 -> s239 [order 2] : R1u {send(R1u_o);}
  s184 -> s191 [order 3] : R2u {send(R2u_o);}
  s184 -> s186 [order 5] : R3r {send(R3r_o);}
  s184 -> s185 [order 6] : R3u {send(R3u_o);}
  s187 -> s185 [order 5] : R3l {send(R3l_o);}
  s192 -> s185 [order 4] : R2d {send(R2d_o);}
  s240 -> s185 [order 1] : R1d {send(R1d_o);}
  s185 -> s240 [order 2] : R1u {send(R1u_o);}
  s185 -> s192 [order 3] : R2u {send(R2u_o);}
  s185 -> s187 [order 5] : R3r {send(R3r_o);}
  s187 -> s186 [order 4] : R3d {send(R3d_o);}
  s188 -> s186 [order 3] : R3l {send(R3l_o);}
  s193 -> s186 [order 3] : R2d {send(R2d_o);}
  s186 -> s193 [order 2] : R2u {send(R2u_o);}
  s186 -> s188 [order 4] : R3r {send(R3r_o);}
  s186 -> s187 [order 5] : R3u {send(R3u_o);}
  s189 -> s187 [order 5] : R3l {send(R3l_o);}
  s194 -> s187 [order 4] : R2d {send(R2d_o);}
  s242 -> s187 [order 1] : R1d {send(R1d_o);}
  s187 -> s242 [order 2] : R1u {send(R1u_o);}
  s187 -> s194 [order 3] : R2u {send(R2u_o);}
  s187 -> s189 [order 6] : R3r {send(R3r_o);}
  s189 -> s188 [order 4] : R3d {send(R3d_o);}
  s243 -> s188 [order 1] : R1d {send(R1d_o);}
  s188 -> s243 [order 2] : R1u {send(R1u_o);}
  s188 -> s189 [order 4] : R3u {send(R3u_o);}
  s188 -> s189 [order 5] : R3ureq {send(R3ureq_o);}
  s196 -> s189 [order 4] : R2d {send(R2d_o);}
  s244 -> s189 [order 1] : R1d {send(R1d_o);}
  s189 -> s244 [order 2] : R1u {send(R1u_o);}
  s189 -> s196 [order 3] : R2u {send(R2u_o);}
  s191 -> s190 [order 7] : R3d {send(R3d_o);}
  s197 -> s190 [order 3] : R2d {send(R2d_o);}
  s245 -> s190 [order 1] : R1d {send(R1d_o);}
  s347 -> s190 [order 1] : R1l {send(R1l_o);}
  s190 -> s347 [order 1] : R1r {send(R1r_o);}
  s190 -> s245 [order 2] : R1u {send(R1u_o);}
  s190 -> s197 [order 5] : R2u {send(R2u_o);}
  s190 -> s191 [order 6] : R3u {send(R3u_o);}
  s192 -> s191 [order 7] : R3d {send(R3d_o);}
  s193 -> s191 [order 5] : R3l {send(R3l_o);}
  s198 -> s191 [order 4] : R2d {send(R2d_o);}
  s246 -> s191 [order 1] : R1d {send(R1d_o);}
  s348 -> s191 [order 1] : R1l {send(R1l_o);}
  s191 -> s348 [order 2] : R1r {send(R1r_o);}
  s191 -> s246 [order 3] : R1u {send(R1u_o);}
  s191 -> s198 [order 6] : R2u {send(R2u_o);}
  s191 -> s193 [order 8] : R3r {send(R3r_o);}
  s191 -> s192 [order 9] : R3u {send(R3u_o);}
  s194 -> s192 [order 7] : R3l {send(R3l_o);}
  s199 -> s192 [order 4] : R2d {send(R2d_o);}
  s247 -> s192 [order 1] : R1d {send(R1d_o);}
  s349 -> s192 [order 1] : R1l {send(R1l_o);}
  s192 -> s349 [order 2] : R1r {send(R1r_o);}
  s192 -> s247 [order 3] : R1u {send(R1u_o);}
  s192 -> s199 [order 6] : R2u {send(R2u_o);}
  s192 -> s194 [order 8] : R3r {send(R3r_o);}
  s194 -> s193 [order 6] : R3d {send(R3d_o);}
  s200 -> s193 [order 3] : R2d {send(R2d_o);}
  s351 -> s193 [order 1] : R1l {send(R1l_o);}
  s193 -> s351 [order 2] : R1r {send(R1r_o);}
  s193 -> s200 [order 4] : R2u {send(R2u_o);}
  s193 -> s194 [order 6] : R3u {send(R3u_o);}
  s196 -> s194 [order 6] : R3l {send(R3l_o);}
  s201 -> s194 [order 4] : R2d {send(R2d_o);}
  s249 -> s194 [order 1] : R1d {send(R1d_o);}
  s352 -> s194 [order 1] : R1l {send(R1l_o);}
  s194 -> s352 [order 2] : R1r {send(R1r_o);}
  s194 -> s249 [order 3] : R1u {send(R1u_o);}
  s194 -> s201 [order 5] : R2u {send(R2u_o);}
  s194 -> s196 [order 8] : R3r {send(R3r_o);}
  s202 -> s195 [order 3] : R2d {send(R2d_o);}
  s250 -> s195 [order 1] : R1d {send(R1d_o);}
  s195 -> s250 [order 2] : R1u {send(R1u_o);}
  s195 -> s202 [order 4] : R2u {send(R2u_o);}
  s251 -> s196 [order 1] : R1d {send(R1d_o);}
  s353 -> s196 [order 1] : R1l {send(R1l_o);}
  s196 -> s353 [order 2] : R1r {send(R1r_o);}
  s196 -> s251 [order 3] : R1u {send(R1u_o);}
  s198 -> s197 [order 6] : R3d {send(R3d_o);}
  s252 -> s197 [order 1] : R1d {send(R1d_o);}
  s354 -> s197 [order 1] : R1l {send(R1l_o);}
  s197 -> s354 [order 1] : R1r {send(R1r_o);}
  s197 -> s252 [order 2] : R1u {send(R1u_o);}
  s197 -> s198 [order 5] : R3u {send(R3u_o);}
  s199 -> s198 [order 6] : R3d {send(R3d_o);}
  s200 -> s198 [order 5] : R3l {send(R3l_o);}
  s253 -> s198 [order 1] : R1d {send(R1d_o);}
  s355 -> s198 [order 1] : R1l {send(R1l_o);}
  s198 -> s355 [order 2] : R1r {send(R1r_o);}
  s198 -> s253 [order 3] : R1u {send(R1u_o);}
  s198 -> s200 [order 7] : R3r {send(R3r_o);}
  s198 -> s199 [order 8] : R3u {send(R3u_o);}
  s201 -> s199 [order 6] : R3l {send(R3l_o);}
  s254 -> s199 [order 1] : R1d {send(R1d_o);}
  s356 -> s199 [order 1] : R1l {send(R1l_o);}
  s199 -> s356 [order 2] : R1r {send(R1r_o);}
  s199 -> s254 [order 3] : R1u {send(R1u_o);}
  s199 -> s201 [order 7] : R3r {send(R3r_o);}
  s201 -> s200 [order 5] : R3d {send(R3d_o);}
  s358 -> s200 [order 1] : R1l {send(R1l_o);}
  s200 -> s358 [order 2] : R1r {send(R1r_o);}
  s200 -> s201 [order 6] : R3u {send(R3u_o);}
  s256 -> s201 [order 1] : R1d {send(R1d_o);}
  s359 -> s201 [order 1] : R1l {send(R1l_o);}
  s201 -> s359 [order 2] : R1r {send(R1r_o);}
  s201 -> s256 [order 3] : R1u {send(R1u_o);}
  s257 -> s202 [order 1] : R1d {send(R1d_o);}
  s202 -> s257 [order 2] : R1u {send(R1u_o);}
  s204 -> s203 [order 6] : R3d {send(R3d_o);}
  s225 -> s203 [order 3] : R2l {send(R2l_o);}
  s258 -> s203 [order 1] : R1d {send(R1d_o);}
  s360 -> s203 [order 2] : R1l {send(R1l_o);}
  s203 -> s360 [order 2] : R1r {send(R1r_o);}
  s203 -> s258 [order 3] : R1u {send(R1u_o);}
  s203 -> s225 [order 4] : R2r {send(R2r_o);}
  s203 -> s204 [order 5] : R3u {send(R3u_o);}
  s206 -> s204 [order 6] : R3l {send(R3l_o);}
  s211 -> s204 [order 4] : R2d {send(R2d_o);}
  s226 -> s204 [order 3] : R2l {send(R2l_o);}
  s259 -> s204 [order 1] : R1d {send(R1d_o);}
  s361 -> s204 [order 2] : R1l {send(R1l_o);}
  s204 -> s361 [order 2] : R1r {send(R1r_o);}
  s204 -> s259 [order 3] : R1u {send(R1u_o);}
  s204 -> s226 [order 4] : R2r {send(R2r_o);}
  s204 -> s211 [order 5] : R2u {send(R2u_o);}
  s204 -> s206 [order 7] : R3r {send(R3r_o);}
  s207 -> s205 [order 7] : R3l {send(R3l_o);}
  s212 -> s205 [order 3] : R2d {send(R2d_o);}
  s260 -> s205 [order 1] : R1d {send(R1d_o);}
  s362 -> s205 [order 2] : R1l {send(R1l_o);}
  s205 -> s362 [order 2] : R1r {send(R1r_o);}
  s205 -> s260 [order 3] : R1u {send(R1u_o);}
  s205 -> s212 [order 4] : R2u {send(R2u_o);}
  s205 -> s207 [order 5] : R3r {send(R3r_o);}
  s209 -> s206 [order 8] : R3l {send(R3l_o);}
  s213 -> s206 [order 3] : R2d {send(R2d_o);}
  s227 -> s206 [order 3] : R2l {send(R2l_o);}
  s364 -> s206 [order 2] : R1l {send(R1l_o);}
  s206 -> s364 [order 3] : R1r {send(R1r_o);}
  s206 -> s227 [order 4] : R2r {send(R2r_o);}
  s206 -> s213 [order 5] : R2u {send(R2u_o);}
  s206 -> s209 [order 7] : R3r {send(R3r_o);}
  s208 -> s207 [order 6] : R3d {send(R3d_o);}
  s214 -> s207 [order 4] : R2d {send(R2d_o);}
  s228 -> s207 [order 4] : R2l {send(R2l_o);}
  s262 -> s207 [order 1] : R1d {send(R1d_o);}
  s365 -> s207 [order 1] : R1l {send(R1l_o);}
  s207 -> s365 [order 3] : R1r {send(R1r_o);}
  s207 -> s262 [order 4] : R1u {send(R1u_o);}
  s207 -> s228 [order 5] : R2r {send(R2r_o);}
  s207 -> s214 [order 6] : R2u {send(R2u_o);}
  s207 -> s208 [order 8] : R3u {send(R3u_o);}
  s209 -> s208 [order 7] : R3d {send(R3d_o);}
  s215 -> s208 [order 3] : R2d {send(R2d_o);}
  s229 -> s208 [order 3] : R2l {send(R2l_o);}
  s263 -> s208 [order 1] : R1d {send(R1d_o);}
  s208 -> s263 [order 3] : R1u {send(R1u_o);}
  s208 -> s229 [order 4] : R2r {send(R2r_o);}
  s208 -> s215 [order 5] : R2u {send(R2u_o);}
  s208 -> s209 [order 7] : R3u {send(R3u_o);}
  s208 -> s209 [order 8] : R3ureq {send(R3ureq_o);}
  s216 -> s209 [order 4] : R2d {send(R2d_o);}
  s230 -> s209 [order 4] : R2l {send(R2l_o);}
  s264 -> s209 [order 1] : R1d {send(R1d_o);}
  s366 -> s209 [order 2] : R1l {send(R1l_o);}
  s209 -> s366 [order 3] : R1r {send(R1r_o);}
  s209 -> s264 [order 4] : R1u {send(R1u_o);}
  s209 -> s230 [order 5] : R2r {send(R2r_o);}
  s209 -> s216 [order 6] : R2u {send(R2u_o);}
  s212 -> s210 [order 5] : R3l {send(R3l_o);}
  s217 -> s210 [order 4] : R2d {send(R2d_o);}
  s265 -> s210 [order 1] : R1d {send(R1d_o);}
  s367 -> s210 [order 2] : R1l {send(R1l_o);}
  s210 -> s367 [order 2] : R1r {send(R1r_o);}
  s210 -> s265 [order 3] : R1u {send(R1u_o);}
  s210 -> s217 [order 4] : R2u {send(R2u_o);}
  s210 -> s212 [order 5] : R3r {send(R3r_o);}
  s213 -> s211 [order 5] : R3l {send(R3l_o);}
  s266 -> s211 [order 1] : R1d {send(R1d_o);}
  s368 -> s211 [order 2] : R1l {send(R1l_o);}
  s211 -> s368 [order 2] : R1r {send(R1r_o);}
  s211 -> s266 [order 3] : R1u {send(R1u_o);}
  s211 -> s213 [order 5] : R3r {send(R3r_o);}
  s214 -> s212 [order 6] : R3l {send(R3l_o);}
  s219 -> s212 [order 3] : R2d {send(R2d_o);}
  s267 -> s212 [order 1] : R1d {send(R1d_o);}
  s369 -> s212 [order 2] : R1l {send(R1l_o);}
  s212 -> s369 [order 1] : R1r {send(R1r_o);}
  s212 -> s267 [order 2] : R1u {send(R1u_o);}
  s212 -> s219 [order 4] : R2u {send(R2u_o);}
  s212 -> s214 [order 6] : R3r {send(R3r_o);}
  s216 -> s213 [order 7] : R3l {send(R3l_o);}
  s220 -> s213 [order 3] : R2d {send(R2d_o);}
  s371 -> s213 [order 2] : R1l {send(R1l_o);}
  s213 -> s371 [order 2] : R1r {send(R1r_o);}
  s213 -> s220 [order 4] : R2u {send(R2u_o);}
  s213 -> s216 [order 6] : R3r {send(R3r_o);}
  s215 -> s214 [order 5] : R3d {send(R3d_o);}
  s221 -> s214 [order 4] : R2d {send(R2d_o);}
  s269 -> s214 [order 1] : R1d {send(R1d_o);}
  s372 -> s214 [order 1] : R1l {send(R1l_o);}
  s214 -> s372 [order 2] : R1r {send(R1r_o);}
  s214 -> s269 [order 3] : R1u {send(R1u_o);}
  s214 -> s221 [order 5] : R2u {send(R2u_o);}
  s214 -> s215 [order 7] : R3u {send(R3u_o);}
  s216 -> s215 [order 6] : R3d {send(R3d_o);}
  s222 -> s215 [order 3] : R2d {send(R2d_o);}
  s270 -> s215 [order 1] : R1d {send(R1d_o);}
  s215 -> s270 [order 2] : R1u {send(R1u_o);}
  s215 -> s222 [order 4] : R2u {send(R2u_o);}
  s215 -> s216 [order 6] : R3u {send(R3u_o);}
  s215 -> s216 [order 7] : R3ureq {send(R3ureq_o);}
  s223 -> s216 [order 4] : R2d {send(R2d_o);}
  s271 -> s216 [order 1] : R1d {send(R1d_o);}
  s373 -> s216 [order 2] : R1l {send(R1l_o);}
  s216 -> s373 [order 2] : R1r {send(R1r_o);}
  s216 -> s271 [order 3] : R1u {send(R1u_o);}
  s216 -> s223 [order 5] : R2u {send(R2u_o);}
  s218 -> s217 [order 5] : R3d {send(R3d_o);}
  s219 -> s217 [order 5] : R3l {send(R3l_o);}
  s231 -> s217 [order 4] : R2l {send(R2l_o);}
  s272 -> s217 [order 1] : R1d {send(R1d_o);}
  s374 -> s217 [order 2] : R1l {send(R1l_o);}
  s217 -> s374 [order 2] : R1r {send(R1r_o);}
  s217 -> s272 [order 3] : R1u {send(R1u_o);}
  s217 -> s231 [order 5] : R2r {send(R2r_o);}
  s217 -> s219 [order 6] : R3r {send(R3r_o);}
  s217 -> s218 [order 7] : R3u {send(R3u_o);}
  s232 -> s218 [order 3] : R2l {send(R2l_o);}
  s273 -> s218 [order 1] : R1d {send(R1d_o);}
  s375 -> s218 [order 2] : R1l {send(R1l_o);}
  s218 -> s375 [order 2] : R1r {send(R1r_o);}
  s218 -> s273 [order 3] : R1u {send(R1u_o);}
  s218 -> s232 [order 4] : R2r {send(R2r_o);}
  s221 -> s219 [order 6] : R3l {send(R3l_o);}
  s234 -> s219 [order 3] : R2l {send(R2l_o);}
  s274 -> s219 [order 1] : R1d {send(R1d_o);}
  s376 -> s219 [order 2] : R1l {send(R1l_o);}
  s219 -> s376 [order 1] : R1r {send(R1r_o);}
  s219 -> s274 [order 2] : R1u {send(R1u_o);}
  s219 -> s234 [order 4] : R2r {send(R2r_o);}
  s219 -> s221 [order 6] : R3r {send(R3r_o);}
  s223 -> s220 [order 7] : R3l {send(R3l_o);}
  s378 -> s220 [order 2] : R1l {send(R1l_o);}
  s220 -> s378 [order 2] : R1r {send(R1r_o);}
  s220 -> s223 [order 4] : R3r {send(R3r_o);}
  s222 -> s221 [order 5] : R3d {send(R3d_o);}
  s235 -> s221 [order 4] : R2l {send(R2l_o);}
  s276 -> s221 [order 1] : R1d {send(R1d_o);}
  s379 -> s221 [order 1] : R1l {send(R1l_o);}
  s221 -> s379 [order 2] : R1r {send(R1r_o);}
  s221 -> s276 [order 3] : R1u {send(R1u_o);}
  s221 -> s235 [order 5] : R2r {send(R2r_o);}
  s221 -> s222 [order 7] : R3u {send(R3u_o);}
  s223 -> s222 [order 6] : R3d {send(R3d_o);}
  s236 -> s222 [order 3] : R2l {send(R2l_o);}
  s277 -> s222 [order 1] : R1d {send(R1d_o);}
  s222 -> s277 [order 2] : R1u {send(R1u_o);}
  s222 -> s236 [order 4] : R2r {send(R2r_o);}
  s222 -> s223 [order 6] : R3u {send(R3u_o);}
  s222 -> s223 [order 7] : R3ureq {send(R3ureq_o);}
  s237 -> s223 [order 4] : R2l {send(R2l_o);}
  s278 -> s223 [order 1] : R1d {send(R1d_o);}
  s380 -> s223 [order 2] : R1l {send(R1l_o);}
  s223 -> s380 [order 2] : R1r {send(R1r_o);}
  s223 -> s278 [order 3] : R1u {send(R1u_o);}
  s223 -> s237 [order 5] : R2r {send(R2r_o);}
  s225 -> s224 [order 5] : R3d {send(R3d_o);}
  s238 -> s224 [order 5] : R2l {send(R2l_o);}
  s279 -> s224 [order 1] : R1d {send(R1d_o);}
  s381 -> s224 [order 2] : R1l {send(R1l_o);}
  s224 -> s381 [order 2] : R1r {send(R1r_o);}
  s224 -> s279 [order 3] : R1u {send(R1u_o);}
  s224 -> s238 [order 4] : R2r {send(R2r_o);}
  s224 -> s225 [order 5] : R3u {send(R3u_o);}
  s226 -> s225 [order 5] : R3d {send(R3d_o);}
  s239 -> s225 [order 4] : R2l {send(R2l_o);}
  s280 -> s225 [order 1] : R1d {send(R1d_o);}
  s382 -> s225 [order 2] : R1l {send(R1l_o);}
  s225 -> s382 [order 1] : R1r {send(R1r_o);}
  s225 -> s280 [order 2] : R1u {send(R1u_o);}
  s225 -> s239 [order 4] : R2r {send(R2r_o);}
  s225 -> s226 [order 6] : R3u {send(R3u_o);}
  s227 -> s226 [order 5] : R3l {send(R3l_o);}
  s240 -> s226 [order 4] : R2l {send(R2l_o);}
  s281 -> s226 [order 1] : R1d {send(R1d_o);}
  s383 -> s226 [order 2] : R1l {send(R1l_o);}
  s226 -> s383 [order 1] : R1r {send(R1r_o);}
  s226 -> s281 [order 2] : R1u {send(R1u_o);}
  s226 -> s240 [order 4] : R2r {send(R2r_o);}
  s226 -> s227 [order 6] : R3r {send(R3r_o);}
  s230 -> s227 [order 7] : R3l {send(R3l_o);}
  s242 -> s227 [order 4] : R2l {send(R2l_o);}
  s385 -> s227 [order 2] : R1l {send(R1l_o);}
  s227 -> s385 [order 2] : R1r {send(R1r_o);}
  s227 -> s242 [order 4] : R2r {send(R2r_o);}
  s227 -> s230 [order 6] : R3r {send(R3r_o);}
  s229 -> s228 [order 5] : R3d {send(R3d_o);}
  s283 -> s228 [order 1] : R1d {send(R1d_o);}
  s386 -> s228 [order 1] : R1l {send(R1l_o);}
  s228 -> s386 [order 2] : R1r {send(R1r_o);}
  s228 -> s283 [order 3] : R1u {send(R1u_o);}
  s228 -> s229 [order 5] : R3u {send(R3u_o);}
  s230 -> s229 [order 6] : R3d {send(R3d_o);}
  s243 -> s229 [order 4] : R2l {send(R2l_o);}
  s284 -> s229 [order 1] : R1d {send(R1d_o);}
  s229 -> s284 [order 2] : R1u {send(R1u_o);}
  s229 -> s243 [order 4] : R2r {send(R2r_o);}
  s229 -> s230 [order 6] : R3u {send(R3u_o);}
  s229 -> s230 [order 7] : R3ureq {send(R3ureq_o);}
  s244 -> s230 [order 5] : R2l {send(R2l_o);}
  s285 -> s230 [order 1] : R1d {send(R1d_o);}
  s387 -> s230 [order 2] : R1l {send(R1l_o);}
  s230 -> s387 [order 2] : R1r {send(R1r_o);}
  s230 -> s285 [order 3] : R1u {send(R1u_o);}
  s230 -> s244 [order 5] : R2r {send(R2r_o);}
  s232 -> s231 [order 5] : R3d {send(R3d_o);}
  s234 -> s231 [order 5] : R3l {send(R3l_o);}
  s252 -> s231 [order 6] : R2l {send(R2l_o);}
  s394 -> s231 [order 2] : R1l {send(R1l_o);}
  s231 -> s394 [order 3] : R1r {send(R1r_o);}
  s231 -> s252 [order 5] : R2r {send(R2r_o);}
  s231 -> s234 [order 6] : R3r {send(R3r_o);}
  s231 -> s232 [order 7] : R3u {send(R3u_o);}
  s233 -> s232 [order 4] : R3d {send(R3d_o);}
  s253 -> s232 [order 5] : R2l {send(R2l_o);}
  s395 -> s232 [order 2] : R1l {send(R1l_o);}
  s232 -> s395 [order 2] : R1r {send(R1r_o);}
  s232 -> s253 [order 4] : R2r {send(R2r_o);}
  s232 -> s233 [order 6] : R3u {send(R3u_o);}
  s254 -> s233 [order 5] : R2l {send(R2l_o);}
  s396 -> s233 [order 2] : R1l {send(R1l_o);}
  s233 -> s396 [order 2] : R1r {send(R1r_o);}
  s233 -> s254 [order 3] : R2r {send(R2r_o);}
  s235 -> s234 [order 6] : R3l {send(R3l_o);}
  s255 -> s234 [order 5] : R2l {send(R2l_o);}
  s397 -> s234 [order 2] : R1l {send(R1l_o);}
  s234 -> s397 [order 2] : R1r {send(R1r_o);}
  s234 -> s255 [order 4] : R2r {send(R2r_o);}
  s234 -> s235 [order 6] : R3r {send(R3r_o);}
  s236 -> s235 [order 4] : R3d {send(R3d_o);}
  s257 -> s235 [order 6] : R2l {send(R2l_o);}
  s399 -> s235 [order 1] : R1l {send(R1l_o);}
  s235 -> s399 [order 3] : R1r {send(R1r_o);}
  s235 -> s257 [order 5] : R2r {send(R2r_o);}
  s235 -> s236 [order 7] : R3u {send(R3u_o);}
  s237 -> s236 [order 5] : R3d {send(R3d_o);}
  s236 -> s237 [order 5] : R3u {send(R3u_o);}
  s236 -> s237 [order 6] : R3ureq {send(R3ureq_o);}
  s400 -> s237 [order 2] : R1l {send(R1l_o);}
  s237 -> s400 [order 3] : R1r {send(R1r_o);}
  s239 -> s238 [order 6] : R3d {send(R3d_o);}
  s241 -> s238 [order 5] : R3l {send(R3l_o);}
  s245 -> s238 [order 4] : R2d {send(R2d_o);}
  s286 -> s238 [order 1] : R1d {send(R1d_o);}
  s401 -> s238 [order 1] : R1l {send(R1l_o);}
  s238 -> s401 [order 3] : R1r {send(R1r_o);}
  s238 -> s286 [order 4] : R1u {send(R1u_o);}
  s238 -> s245 [order 6] : R2u {send(R2u_o);}
  s238 -> s241 [order 7] : R3r {send(R3r_o);}
  s238 -> s239 [order 8] : R3u {send(R3u_o);}
  s240 -> s239 [order 6] : R3d {send(R3d_o);}
  s246 -> s239 [order 3] : R2d {send(R2d_o);}
  s287 -> s239 [order 1] : R1d {send(R1d_o);}
  s402 -> s239 [order 1] : R1l {send(R1l_o);}
  s239 -> s402 [order 2] : R1r {send(R1r_o);}
  s239 -> s287 [order 3] : R1u {send(R1u_o);}
  s239 -> s246 [order 5] : R2u {send(R2u_o);}
  s239 -> s240 [order 7] : R3u {send(R3u_o);}
  s242 -> s240 [order 6] : R3l {send(R3l_o);}
  s247 -> s240 [order 3] : R2d {send(R2d_o);}
  s288 -> s240 [order 1] : R1d {send(R1d_o);}
  s403 -> s240 [order 1] : R1l {send(R1l_o);}
  s240 -> s403 [order 2] : R1r {send(R1r_o);}
  s240 -> s288 [order 3] : R1u {send(R1u_o);}
  s240 -> s247 [order 5] : R2u {send(R2u_o);}
  s240 -> s242 [order 7] : R3r {send(R3r_o);}
  s248 -> s241 [order 3] : R2d {send(R2d_o);}
  s289 -> s241 [order 1] : R1d {send(R1d_o);}
  s404 -> s241 [order 1] : R1l {send(R1l_o);}
  s241 -> s404 [order 2] : R1r {send(R1r_o);}
  s241 -> s289 [order 3] : R1u {send(R1u_o);}
  s241 -> s248 [order 4] : R2u {send(R2u_o);}
  s244 -> s242 [order 8] : R3l {send(R3l_o);}
  s249 -> s242 [order 3] : R2d {send(R2d_o);}
  s406 -> s242 [order 1] : R1l {send(R1l_o);}
  s242 -> s406 [order 3] : R1r {send(R1r_o);}
  s242 -> s249 [order 5] : R2u {send(R2u_o);}
  s242 -> s244 [order 7] : R3r {send(R3r_o);}
  s244 -> s243 [order 7] : R3d {send(R3d_o);}
  s291 -> s243 [order 1] : R1d {send(R1d_o);}
  s243 -> s291 [order 3] : R1u {send(R1u_o);}
  s243 -> s244 [order 5] : R3u {send(R3u_o);}
  s243 -> s244 [order 6] : R3ureq {send(R3ureq_o);}
  s251 -> s244 [order 4] : R2d {send(R2d_o);}
  s292 -> s244 [order 1] : R1d {send(R1d_o);}
  s407 -> s244 [order 1] : R1l {send(R1l_o);}
  s244 -> s407 [order 3] : R1r {send(R1r_o);}
  s244 -> s292 [order 4] : R1u {send(R1u_o);}
  s244 -> s251 [order 6] : R2u {send(R2u_o);}
  s246 -> s245 [order 5] : R3d {send(R3d_o);}
  s248 -> s245 [order 5] : R3l {send(R3l_o);}
  s252 -> s245 [order 5] : R2d {send(R2d_o);}
  s293 -> s245 [order 1] : R1d {send(R1d_o);}
  s245 -> s293 [order 3] : R1u {send(R1u_o);}
  s245 -> s252 [order 5] : R2u {send(R2u_o);}
  s245 -> s248 [order 6] : R3r {send(R3r_o);}
  s245 -> s246 [order 7] : R3u {send(R3u_o);}
  s247 -> s246 [order 5] : R3d {send(R3d_o);}
  s253 -> s246 [order 4] : R2d {send(R2d_o);}
  s294 -> s246 [order 1] : R1d {send(R1d_o);}
  s246 -> s294 [order 2] : R1u {send(R1u_o);}
  s246 -> s253 [order 4] : R2u {send(R2u_o);}
  s246 -> s247 [order 6] : R3u {send(R3u_o);}
  s249 -> s247 [order 5] : R3l {send(R3l_o);}
  s254 -> s247 [order 4] : R2d {send(R2d_o);}
  s295 -> s247 [order 1] : R1d {send(R1d_o);}
  s247 -> s295 [order 2] : R1u {send(R1u_o);}
  s247 -> s254 [order 4] : R2u {send(R2u_o);}
  s247 -> s249 [order 6] : R3r {send(R3r_o);}
  s250 -> s248 [order 5] : R3l {send(R3l_o);}
  s255 -> s248 [order 4] : R2d {send(R2d_o);}
  s296 -> s248 [order 1] : R1d {send(R1d_o);}
  s248 -> s296 [order 2] : R1u {send(R1u_o);}
  s248 -> s255 [order 4] : R2u {send(R2u_o);}
  s248 -> s250 [order 6] : R3r {send(R3r_o);}
  s251 -> s249 [order 5] : R3l {send(R3l_o);}
  s256 -> s249 [order 4] : R2d {send(R2d_o);}
  s249 -> s256 [order 4] : R2u {send(R2u_o);}
  s249 -> s251 [order 6] : R3r {send(R3r_o);}
  s257 -> s250 [order 5] : R2d {send(R2d_o);}
  s298 -> s250 [order 1] : R1d {send(R1d_o);}
  s250 -> s298 [order 3] : R1u {send(R1u_o);}
  s250 -> s257 [order 4] : R2u {send(R2u_o);}
  s299 -> s251 [order 1] : R1d {send(R1d_o);}
  s251 -> s299 [order 3] : R1u {send(R1u_o);}
  s253 -> s252 [order 6] : R3d {send(R3d_o);}
  s255 -> s252 [order 6] : R3l {send(R3l_o);}
  s300 -> s252 [order 1] : R1d {send(R1d_o);}
  s408 -> s252 [order 2] : R1l {send(R1l_o);}
  s252 -> s408 [order 3] : R1r {send(R1r_o);}
  s252 -> s300 [order 4] : R1u {send(R1u_o);}
  s252 -> s255 [order 7] : R3r {send(R3r_o);}
  s252 -> s253 [order 8] : R3u {send(R3u_o);}
  s254 -> s253 [order 6] : R3d {send(R3d_o);}
  s301 -> s253 [order 1] : R1d {send(R1d_o);}
  s409 -> s253 [order 2] : R1l {send(R1l_o);}
  s253 -> s409 [order 2] : R1r {send(R1r_o);}
  s253 -> s301 [order 3] : R1u {send(R1u_o);}
  s253 -> s254 [order 7] : R3u {send(R3u_o);}
  s256 -> s254 [order 5] : R3l {send(R3l_o);}
  s302 -> s254 [order 1] : R1d {send(R1d_o);}
  s410 -> s254 [order 2] : R1l {send(R1l_o);}
  s254 -> s410 [order 2] : R1r {send(R1r_o);}
  s254 -> s302 [order 3] : R1u {send(R1u_o);}
  s254 -> s256 [order 7] : R3r {send(R3r_o);}
  s257 -> s255 [order 7] : R3l {send(R3l_o);}
  s303 -> s255 [order 1] : R1d {send(R1d_o);}
  s411 -> s255 [order 2] : R1l {send(R1l_o);}
  s255 -> s411 [order 2] : R1r {send(R1r_o);}
  s255 -> s303 [order 3] : R1u {send(R1u_o);}
  s255 -> s257 [order 7] : R3r {send(R3r_o);}
  s413 -> s256 [order 2] : R1l {send(R1l_o);}
  s256 -> s413 [order 3] : R1r {send(R1r_o);}
  s305 -> s257 [order 1] : R1d {send(R1d_o);}
  s414 -> s257 [order 1] : R1l {send(R1l_o);}
  s257 -> s414 [order 3] : R1r {send(R1r_o);}
  s257 -> s305 [order 4] : R1u {send(R1u_o);}
  s259 -> s258 [order 5] : R3d {send(R3d_o);}
  s261 -> s258 [order 6] : R3l {send(R3l_o);}
  s280 -> s258 [order 4] : R2l {send(R2l_o);}
  s415 -> s258 [order 2] : R1l {send(R1l_o);}
  s258 -> s415 [order 3] : R1r {send(R1r_o);}
  s258 -> s280 [order 4] : R2r {send(R2r_o);}
  s258 -> s261 [order 5] : R3r {send(R3r_o);}
  s258 -> s259 [order 6] : R3u {send(R3u_o);}
  s266 -> s259 [order 3] : R2d {send(R2d_o);}
  s281 -> s259 [order 3] : R2l {send(R2l_o);}
  s416 -> s259 [order 2] : R1l {send(R1l_o);}
  s259 -> s416 [order 2] : R1r {send(R1r_o);}
  s259 -> s281 [order 3] : R2r {send(R2r_o);}
  s259 -> s266 [order 4] : R2u {send(R2u_o);}
  s261 -> s260 [order 5] : R3d {send(R3d_o);}
  s262 -> s260 [order 6] : R3l {send(R3l_o);}
  s267 -> s260 [order 4] : R2d {send(R2d_o);}
  s417 -> s260 [order 2] : R1l {send(R1l_o);}
  s260 -> s417 [order 3] : R1r {send(R1r_o);}
  s260 -> s267 [order 4] : R2u {send(R2u_o);}
  s260 -> s262 [order 5] : R3r {send(R3r_o);}
  s260 -> s261 [order 6] : R3u {send(R3u_o);}
  s263 -> s261 [order 6] : R3l {send(R3l_o);}
  s268 -> s261 [order 3] : R2d {send(R2d_o);}
  s282 -> s261 [order 3] : R2l {send(R2l_o);}
  s418 -> s261 [order 2] : R1l {send(R1l_o);}
  s261 -> s418 [order 2] : R1r {send(R1r_o);}
  s261 -> s282 [order 3] : R2r {send(R2r_o);}
  s261 -> s268 [order 4] : R2u {send(R2u_o);}
  s261 -> s263 [order 7] : R3r {send(R3r_o);}
  s263 -> s262 [order 5] : R3d {send(R3d_o);}
  s269 -> s262 [order 4] : R2d {send(R2d_o);}
  s283 -> s262 [order 4] : R2l {send(R2l_o);}
  s420 -> s262 [order 2] : R1l {send(R1l_o);}
  s262 -> s420 [order 3] : R1r {send(R1r_o);}
  s262 -> s283 [order 4] : R2r {send(R2r_o);}
  s262 -> s269 [order 5] : R2u {send(R2u_o);}
  s262 -> s263 [order 7] : R3u {send(R3u_o);}
  s264 -> s263 [order 5] : R3d {send(R3d_o);}
  s270 -> s263 [order 3] : R2d {send(R2d_o);}
  s284 -> s263 [order 3] : R2l {send(R2l_o);}
  s263 -> s284 [order 3] : R2r {send(R2r_o);}
  s263 -> s270 [order 4] : R2u {send(R2u_o);}
  s263 -> s264 [order 7] : R3u {send(R3u_o);}
  s263 -> s264 [order 8] : R3ureq {send(R3ureq_o);}
  s271 -> s264 [order 3] : R2d {send(R2d_o);}
  s285 -> s264 [order 3] : R2l {send(R2l_o);}
  s264 -> s285 [order 3] : R2r {send(R2r_o);}
  s264 -> s271 [order 4] : R2u {send(R2u_o);}
  s267 -> s265 [order 6] : R3l {send(R3l_o);}
  s272 -> s265 [order 3] : R2d {send(R2d_o);}
  s421 -> s265 [order 2] : R1l {send(R1l_o);}
  s265 -> s421 [order 3] : R1r {send(R1r_o);}
  s265 -> s272 [order 4] : R2u {send(R2u_o);}
  s265 -> s267 [order 5] : R3r {send(R3r_o);}
  s422 -> s266 [order 2] : R1l {send(R1l_o);}
  s266 -> s422 [order 2] : R1r {send(R1r_o);}
  s268 -> s267 [order 5] : R3d {send(R3d_o);}
  s269 -> s267 [order 6] : R3l {send(R3l_o);}
  s274 -> s267 [order 3] : R2d {send(R2d_o);}
  s423 -> s267 [order 2] : R1l {send(R1l_o);}
  s267 -> s423 [order 3] : R1r {send(R1r_o);}
  s267 -> s274 [order 5] : R2u {send(R2u_o);}
  s267 -> s269 [order 7] : R3r {send(R3r_o);}
  s267 -> s268 [order 8] : R3u {send(R3u_o);}
  s270 -> s268 [order 6] : R3l {send(R3l_o);}
  s275 -> s268 [order 2] : R2d {send(R2d_o);}
  s424 -> s268 [order 2] : R1l {send(R1l_o);}
  s268 -> s424 [order 2] : R1r {send(R1r_o);}
  s268 -> s275 [order 4] : R2u {send(R2u_o);}
  s268 -> s270 [order 6] : R3r {send(R3r_o);}
  s270 -> s269 [order 5] : R3d {send(R3d_o);}
  s276 -> s269 [order 3] : R2d {send(R2d_o);}
  s426 -> s269 [order 2] : R1l {send(R1l_o);}
  s269 -> s426 [order 3] : R1r {send(R1r_o);}
  s269 -> s276 [order 5] : R2u {send(R2u_o);}
  s269 -> s270 [order 7] : R3u {send(R3u_o);}
  s271 -> s270 [order 5] : R3d {send(R3d_o);}
  s277 -> s270 [order 2] : R2d {send(R2d_o);}
  s270 -> s277 [order 4] : R2u {send(R2u_o);}
  s270 -> s271 [order 7] : R3u {send(R3u_o);}
  s270 -> s271 [order 8] : R3ureq {send(R3ureq_o);}
  s278 -> s271 [order 2] : R2d {send(R2d_o);}
  s271 -> s278 [order 4] : R2u {send(R2u_o);}
  s273 -> s272 [order 3] : R3d {send(R3d_o);}
  s274 -> s272 [order 4] : R3l {send(R3l_o);}
  s427 -> s272 [order 2] : R1l {send(R1l_o);}
  s272 -> s427 [order 2] : R1r {send(R1r_o);}
  s272 -> s274 [order 4] : R3r {send(R3r_o);}
  s272 -> s273 [order 5] : R3u {send(R3u_o);}
  s275 -> s273 [order 4] : R3l {send(R3l_o);}
  s428 -> s273 [order 2] : R1l {send(R1l_o);}
  s273 -> s428 [order 2] : R1r {send(R1r_o);}
  s273 -> s275 [order 4] : R3r {send(R3r_o);}
  s275 -> s274 [order 3] : R3d {send(R3d_o);}
  s276 -> s274 [order 4] : R3l {send(R3l_o);}
  s429 -> s274 [order 2] : R1l {send(R1l_o);}
  s274 -> s429 [order 2] : R1r {send(R1r_o);}
  s274 -> s276 [order 5] : R3r {send(R3r_o);}
  s274 -> s275 [order 6] : R3u {send(R3u_o);}
  s277 -> s275 [order 4] : R3l {send(R3l_o);}
  s430 -> s275 [order 2] : R1l {send(R1l_o);}
  s275 -> s430 [order 1] : R1r {send(R1r_o);}
  s275 -> s277 [order 5] : R3r {send(R3r_o);}
  s277 -> s276 [order 3] : R3d {send(R3d_o);}
  s432 -> s276 [order 2] : R1l {send(R1l_o);}
  s276 -> s432 [order 2] : R1r {send(R1r_o);}
  s276 -> s277 [order 5] : R3u {send(R3u_o);}
  s278 -> s277 [order 3] : R3d {send(R3d_o);}
  s277 -> s278 [order 5] : R3u {send(R3u_o);}
  s277 -> s278 [order 6] : R3ureq {send(R3ureq_o);}
  s280 -> s279 [order 6] : R3d {send(R3d_o);}
  s286 -> s279 [order 4] : R2l {send(R2l_o);}
  s433 -> s279 [order 2] : R1l {send(R1l_o);}
  s279 -> s433 [order 3] : R1r {send(R1r_o);}
  s279 -> s286 [order 4] : R2r {send(R2r_o);}
  s279 -> s280 [order 5] : R3u {send(R3u_o);}
  s281 -> s280 [order 5] : R3d {send(R3d_o);}
  s282 -> s280 [order 5] : R3l {send(R3l_o);}
  s287 -> s280 [order 4] : R2l {send(R2l_o);}
  s434 -> s280 [order 2] : R1l {send(R1l_o);}
  s280 -> s434 [order 3] : R1r {send(R1r_o);}
  s280 -> s287 [order 5] : R2r {send(R2r_o);}
  s280 -> s282 [order 7] : R3r {send(R3r_o);}
  s280 -> s281 [order 8] : R3u {send(R3u_o);}
  s288 -> s281 [order 3] : R2l {send(R2l_o);}
  s435 -> s281 [order 2] : R1l {send(R1l_o);}
  s281 -> s435 [order 2] : R1r {send(R1r_o);}
  s281 -> s288 [order 4] : R2r {send(R2r_o);}
  s284 -> s282 [order 6] : R3l {send(R3l_o);}
  s290 -> s282 [order 3] : R2l {send(R2l_o);}
  s436 -> s282 [order 2] : R1l {send(R1l_o);}
  s282 -> s436 [order 2] : R1r {send(R1r_o);}
  s282 -> s290 [order 4] : R2r {send(R2r_o);}
  s282 -> s284 [order 6] : R3r {send(R3r_o);}
  s284 -> s283 [order 5] : R3d {send(R3d_o);}
  s438 -> s283 [order 2] : R1l {send(R1l_o);}
  s283 -> s438 [order 3] : R1r {send(R1r_o);}
  s283 -> s284 [order 5] : R3u {send(R3u_o);}
  s285 -> s284 [order 5] : R3d {send(R3d_o);}
  s291 -> s284 [order 3] : R2l {send(R2l_o);}
  s284 -> s291 [order 4] : R2r {send(R2r_o);}
  s284 -> s285 [order 7] : R3u {send(R3u_o);}
  s284 -> s285 [order 8] : R3ureq {send(R3ureq_o);}
  s292 -> s285 [order 3] : R2l {send(R2l_o);}
  s285 -> s292 [order 4] : R2r {send(R2r_o);}
  s287 -> s286 [order 6] : R3d {send(R3d_o);}
  s289 -> s286 [order 5] : R3l {send(R3l_o);}
  s293 -> s286 [order 4] : R2d {send(R2d_o);}
  s450 -> s286 [order 2] : R1l {send(R1l_o);}
  s286 -> s450 [order 3] : R1r {send(R1r_o);}
  s286 -> s293 [order 5] : R2u {send(R2u_o);}
  s286 -> s289 [order 6] : R3r {send(R3r_o);}
  s286 -> s287 [order 7] : R3u {send(R3u_o);}
  s288 -> s287 [order 5] : R3d {send(R3d_o);}
  s290 -> s287 [order 6] : R3l {send(R3l_o);}
  s294 -> s287 [order 4] : R2d {send(R2d_o);}
  s451 -> s287 [order 2] : R1l {send(R1l_o);}
  s287 -> s451 [order 3] : R1r {send(R1r_o);}
  s287 -> s294 [order 5] : R2u {send(R2u_o);}
  s287 -> s290 [order 7] : R3r {send(R3r_o);}
  s287 -> s288 [order 8] : R3u {send(R3u_o);}
  s295 -> s288 [order 3] : R2d {send(R2d_o);}
  s452 -> s288 [order 2] : R1l {send(R1l_o);}
  s288 -> s452 [order 2] : R1r {send(R1r_o);}
  s288 -> s295 [order 4] : R2u {send(R2u_o);}
  s290 -> s289 [order 5] : R3d {send(R3d_o);}
  s296 -> s289 [order 4] : R2d {send(R2d_o);}
  s453 -> s289 [order 2] : R1l {send(R1l_o);}
  s289 -> s453 [order 3] : R1r {send(R1r_o);}
  s289 -> s296 [order 4] : R2u {send(R2u_o);}
  s289 -> s290 [order 6] : R3u {send(R3u_o);}
  s291 -> s290 [order 4] : R3l {send(R3l_o);}
  s297 -> s290 [order 3] : R2d {send(R2d_o);}
  s454 -> s290 [order 2] : R1l {send(R1l_o);}
  s290 -> s454 [order 2] : R1r {send(R1r_o);}
  s290 -> s297 [order 4] : R2u {send(R2u_o);}
  s290 -> s291 [order 7] : R3r {send(R3r_o);}
  s292 -> s291 [order 5] : R3d {send(R3d_o);}
  s291 -> s292 [order 5] : R3u {send(R3u_o);}
  s291 -> s292 [order 6] : R3ureq {send(R3ureq_o);}
  s299 -> s292 [order 3] : R2d {send(R2d_o);}
  s292 -> s299 [order 4] : R2u {send(R2u_o);}
  s294 -> s293 [order 6] : R3d {send(R3d_o);}
  s296 -> s293 [order 6] : R3l {send(R3l_o);}
  s300 -> s293 [order 3] : R2d {send(R2d_o);}
  s456 -> s293 [order 1] : R1l {send(R1l_o);}
  s293 -> s456 [order 3] : R1r {send(R1r_o);}
  s293 -> s300 [order 5] : R2u {send(R2u_o);}
  s293 -> s296 [order 6] : R3r {send(R3r_o);}
  s293 -> s294 [order 7] : R3u {send(R3u_o);}
  s295 -> s294 [order 5] : R3d {send(R3d_o);}
  s297 -> s294 [order 6] : R3l {send(R3l_o);}
  s301 -> s294 [order 3] : R2d {send(R2d_o);}
  s457 -> s294 [order 1] : R1l {send(R1l_o);}
  s294 -> s457 [order 3] : R1r {send(R1r_o);}
  s294 -> s301 [order 5] : R2u {send(R2u_o);}
  s294 -> s297 [order 7] : R3r {send(R3r_o);}
  s294 -> s295 [order 8] : R3u {send(R3u_o);}
  s302 -> s295 [order 2] : R2d {send(R2d_o);}
  s458 -> s295 [order 1] : R1l {send(R1l_o);}
  s295 -> s458 [order 2] : R1r {send(R1r_o);}
  s295 -> s302 [order 4] : R2u {send(R2u_o);}
  s297 -> s296 [order 5] : R3d {send(R3d_o);}
  s298 -> s296 [order 5] : R3l {send(R3l_o);}
  s303 -> s296 [order 3] : R2d {send(R2d_o);}
  s459 -> s296 [order 1] : R1l {send(R1l_o);}
  s296 -> s459 [order 3] : R1r {send(R1r_o);}
  s296 -> s303 [order 5] : R2u {send(R2u_o);}
  s296 -> s298 [order 7] : R3r {send(R3r_o);}
  s296 -> s297 [order 8] : R3u {send(R3u_o);}
  s304 -> s297 [order 2] : R2d {send(R2d_o);}
  s460 -> s297 [order 1] : R1l {send(R1l_o);}
  s297 -> s460 [order 2] : R1r {send(R1r_o);}
  s297 -> s304 [order 4] : R2u {send(R2u_o);}
  s305 -> s298 [order 3] : R2d {send(R2d_o);}
  s462 -> s298 [order 1] : R1l {send(R1l_o);}
  s298 -> s462 [order 3] : R1r {send(R1r_o);}
  s298 -> s305 [order 4] : R2u {send(R2u_o);}
  s301 -> s300 [order 4] : R3d {send(R3d_o);}
  s303 -> s300 [order 4] : R3l {send(R3l_o);}
  s300 -> s303 [order 4] : R3r {send(R3r_o);}
  s300 -> s301 [order 5] : R3u {send(R3u_o);}
  s302 -> s301 [order 3] : R3d {send(R3d_o);}
  s304 -> s301 [order 4] : R3l {send(R3l_o);}
  s301 -> s304 [order 5] : R3r {send(R3r_o);}
  s301 -> s302 [order 6] : R3u {send(R3u_o);}
  s304 -> s303 [order 3] : R3d {send(R3d_o);}
  s305 -> s303 [order 4] : R3l {send(R3l_o);}
  s303 -> s305 [order 5] : R3r {send(R3r_o);}
  s303 -> s304 [order 6] : R3u {send(R3u_o);}
  s307 -> s306 [order 5] : R3d {send(R3d_o);}
  s309 -> s306 [order 6] : R3l {send(R3l_o);}
  s328 -> s306 [order 2] : R2l {send(R2l_o);}
  s360 -> s306 [order 1] : R1d {send(R1d_o);}
  s306 -> s360 [order 2] : R1u {send(R1u_o);}
  s306 -> s328 [order 3] : R2r {send(R2r_o);}
  s306 -> s309 [order 4] : R3r {send(R3r_o);}
  s306 -> s307 [order 5] : R3u {send(R3u_o);}
  s310 -> s307 [order 6] : R3l {send(R3l_o);}
  s314 -> s307 [order 3] : R2d {send(R2d_o);}
  s329 -> s307 [order 2] : R2l {send(R2l_o);}
  s361 -> s307 [order 1] : R1d {send(R1d_o);}
  s307 -> s361 [order 2] : R1u {send(R1u_o);}
  s307 -> s329 [order 3] : R2r {send(R2r_o);}
  s307 -> s314 [order 4] : R2u {send(R2u_o);}
  s307 -> s310 [order 6] : R3r {send(R3r_o);}
  s309 -> s308 [order 5] : R3d {send(R3d_o);}
  s315 -> s308 [order 2] : R2d {send(R2d_o);}
  s362 -> s308 [order 1] : R1d {send(R1d_o);}
  s308 -> s362 [order 1] : R1u {send(R1u_o);}
  s308 -> s315 [order 2] : R2u {send(R2u_o);}
  s308 -> s309 [order 3] : R3u {send(R3u_o);}
  s310 -> s309 [order 5] : R3d {send(R3d_o);}
  s311 -> s309 [order 4] : R3l {send(R3l_o);}
  s316 -> s309 [order 3] : R2d {send(R2d_o);}
  s330 -> s309 [order 2] : R2l {send(R2l_o);}
  s363 -> s309 [order 1] : R1d {send(R1d_o);}
  s309 -> s363 [order 2] : R1u {send(R1u_o);}
  s309 -> s330 [order 3] : R2r {send(R2r_o);}
  s309 -> s316 [order 4] : R2u {send(R2u_o);}
  s309 -> s311 [order 7] : R3r {send(R3r_o);}
  s309 -> s310 [order 8] : R3u {send(R3u_o);}
  s312 -> s310 [order 6] : R3l {send(R3l_o);}
  s317 -> s310 [order 3] : R2d {send(R2d_o);}
  s331 -> s310 [order 2] : R2l {send(R2l_o);}
  s364 -> s310 [order 1] : R1d {send(R1d_o);}
  s310 -> s364 [order 2] : R1u {send(R1u_o);}
  s310 -> s331 [order 3] : R2r {send(R2r_o);}
  s310 -> s317 [order 4] : R2u {send(R2u_o);}
  s310 -> s312 [order 7] : R3r {send(R3r_o);}
  s312 -> s311 [order 5] : R3d {send(R3d_o);}
  s318 -> s311 [order 2] : R2d {send(R2d_o);}
  s332 -> s311 [order 1] : R2l {send(R2l_o);}
  s311 -> s332 [order 2] : R2r {send(R2r_o);}
  s311 -> s318 [order 3] : R2u {send(R2u_o);}
  s311 -> s312 [order 5] : R3u {send(R3u_o);}
  s311 -> s312 [order 6] : R3ureq {send(R3ureq_o);}
  s319 -> s312 [order 3] : R2d {send(R2d_o);}
  s333 -> s312 [order 2] : R2l {send(R2l_o);}
  s366 -> s312 [order 1] : R1d {send(R1d_o);}
  s312 -> s366 [order 2] : R1u {send(R1u_o);}
  s312 -> s333 [order 3] : R2r {send(R2r_o);}
  s312 -> s319 [order 4] : R2u {send(R2u_o);}
  s315 -> s313 [order 5] : R3l {send(R3l_o);}
  s320 -> s313 [order 3] : R2d {send(R2d_o);}
  s334 -> s313 [order 4] : R2l {send(R2l_o);}
  s367 -> s313 [order 1] : R1d {send(R1d_o);}
  s313 -> s367 [order 2] : R1u {send(R1u_o);}
  s313 -> s334 [order 3] : R2r {send(R2r_o);}
  s313 -> s320 [order 4] : R2u {send(R2u_o);}
  s313 -> s315 [order 5] : R3r {send(R3r_o);}
  s317 -> s314 [order 6] : R3l {send(R3l_o);}
  s336 -> s314 [order 4] : R2l {send(R2l_o);}
  s368 -> s314 [order 1] : R1d {send(R1d_o);}
  s314 -> s368 [order 2] : R1u {send(R1u_o);}
  s314 -> s336 [order 4] : R2r {send(R2r_o);}
  s314 -> s317 [order 5] : R3r {send(R3r_o);}
  s316 -> s315 [order 5] : R3d {send(R3d_o);}
  s322 -> s315 [order 2] : R2d {send(R2d_o);}
  s337 -> s315 [order 2] : R2l {send(R2l_o);}
  s369 -> s315 [order 1] : R1d {send(R1d_o);}
  s315 -> s369 [order 1] : R1u {send(R1u_o);}
  s315 -> s337 [order 3] : R2r {send(R2r_o);}
  s315 -> s322 [order 4] : R2u {send(R2u_o);}
  s315 -> s316 [order 6] : R3u {send(R3u_o);}
  s317 -> s316 [order 5] : R3d {send(R3d_o);}
  s318 -> s316 [order 5] : R3l {send(R3l_o);}
  s323 -> s316 [order 3] : R2d {send(R2d_o);}
  s370 -> s316 [order 1] : R1d {send(R1d_o);}
  s316 -> s370 [order 2] : R1u {send(R1u_o);}
  s316 -> s323 [order 4] : R2u {send(R2u_o);}
  s316 -> s318 [order 6] : R3r {send(R3r_o);}
  s316 -> s317 [order 7] : R3u {send(R3u_o);}
  s319 -> s317 [order 7] : R3l {send(R3l_o);}
  s324 -> s317 [order 3] : R2d {send(R2d_o);}
  s371 -> s317 [order 1] : R1d {send(R1d_o);}
  s317 -> s371 [order 2] : R1u {send(R1u_o);}
  s317 -> s324 [order 4] : R2u {send(R2u_o);}
  s317 -> s319 [order 7] : R3r {send(R3r_o);}
  s319 -> s318 [order 6] : R3d {send(R3d_o);}
  s325 -> s318 [order 2] : R2d {send(R2d_o);}
  s338 -> s318 [order 3] : R2l {send(R2l_o);}
  s318 -> s338 [order 3] : R2r {send(R2r_o);}
  s318 -> s325 [order 4] : R2u {send(R2u_o);}
  s318 -> s319 [order 6] : R3u {send(R3u_o);}
  s318 -> s319 [order 7] : R3ureq {send(R3ureq_o);}
  s326 -> s319 [order 3] : R2d {send(R2d_o);}
  s339 -> s319 [order 4] : R2l {send(R2l_o);}
  s373 -> s319 [order 1] : R1d {send(R1d_o);}
  s319 -> s373 [order 2] : R1u {send(R1u_o);}
  s319 -> s339 [order 4] : R2r {send(R2r_o);}
  s319 -> s326 [order 5] : R2u {send(R2u_o);}
  s321 -> s320 [order 4] : R3d {send(R3d_o);}
  s322 -> s320 [order 4] : R3l {send(R3l_o);}
  s340 -> s320 [order 4] : R2l {send(R2l_o);}
  s374 -> s320 [order 1] : R1d {send(R1d_o);}
  s320 -> s374 [order 2] : R1u {send(R1u_o);}
  s320 -> s340 [order 4] : R2r {send(R2r_o);}
  s320 -> s322 [order 5] : R3r {send(R3r_o);}
  s320 -> s321 [order 6] : R3u {send(R3u_o);}
  s323 -> s321 [order 6] : R3l {send(R3l_o);}
  s341 -> s321 [order 4] : R2l {send(R2l_o);}
  s375 -> s321 [order 1] : R1d {send(R1d_o);}
  s321 -> s375 [order 2] : R1u {send(R1u_o);}
  s321 -> s341 [order 3] : R2r {send(R2r_o);}
  s321 -> s323 [order 5] : R3r {send(R3r_o);}
  s323 -> s322 [order 5] : R3d {send(R3d_o);}
  s343 -> s322 [order 3] : R2l {send(R2l_o);}
  s376 -> s322 [order 1] : R1d {send(R1d_o);}
  s322 -> s376 [order 1] : R1u {send(R1u_o);}
  s322 -> s343 [order 3] : R2r {send(R2r_o);}
  s322 -> s323 [order 5] : R3u {send(R3u_o);}
  s324 -> s323 [order 4] : R3d {send(R3d_o);}
  s325 -> s323 [order 4] : R3l {send(R3l_o);}
  s344 -> s323 [order 3] : R2l {send(R2l_o);}
  s377 -> s323 [order 1] : R1d {send(R1d_o);}
  s323 -> s377 [order 2] : R1u {send(R1u_o);}
  s323 -> s344 [order 4] : R2r {send(R2r_o);}
  s323 -> s325 [order 7] : R3r {send(R3r_o);}
  s323 -> s324 [order 8] : R3u {send(R3u_o);}
  s326 -> s324 [order 6] : R3l {send(R3l_o);}
  s378 -> s324 [order 1] : R1d {send(R1d_o);}
  s324 -> s378 [order 2] : R1u {send(R1u_o);}
  s324 -> s326 [order 5] : R3r {send(R3r_o);}
  s326 -> s325 [order 5] : R3d {send(R3d_o);}
  s345 -> s325 [order 3] : R2l {send(R2l_o);}
  s325 -> s345 [order 3] : R2r {send(R2r_o);}
  s325 -> s326 [order 5] : R3u {send(R3u_o);}
  s325 -> s326 [order 6] : R3ureq {send(R3ureq_o);}
  s346 -> s326 [order 4] : R2l {send(R2l_o);}
  s380 -> s326 [order 1] : R1d {send(R1d_o);}
  s326 -> s380 [order 2] : R1u {send(R1u_o);}
  s326 -> s346 [order 4] : R2r {send(R2r_o);}
  s328 -> s327 [order 4] : R3d {send(R3d_o);}
  s334 -> s327 [order 3] : R2d {send(R2d_o);}
  s381 -> s327 [order 1] : R1d {send(R1d_o);}
  s327 -> s381 [order 1] : R1u {send(R1u_o);}
  s327 -> s334 [order 2] : R2u {send(R2u_o);}
  s327 -> s328 [order 3] : R3u {send(R3u_o);}
  s329 -> s328 [order 4] : R3d {send(R3d_o);}
  s330 -> s328 [order 3] : R3l {send(R3l_o);}
  s335 -> s328 [order 3] : R2d {send(R2d_o);}
  s382 -> s328 [order 1] : R1d {send(R1d_o);}
  s328 -> s382 [order 1] : R1u {send(R1u_o);}
  s328 -> s335 [order 3] : R2u {send(R2u_o);}
  s328 -> s330 [order 5] : R3r {send(R3r_o);}
  s328 -> s329 [order 6] : R3u {send(R3u_o);}
  s331 -> s329 [order 4] : R3l {send(R3l_o);}
  s336 -> s329 [order 3] : R2d {send(R2d_o);}
  s383 -> s329 [order 1] : R1d {send(R1d_o);}
  s329 -> s383 [order 1] : R1u {send(R1u_o);}
  s329 -> s336 [order 3] : R2u {send(R2u_o);}
  s329 -> s331 [order 5] : R3r {send(R3r_o);}
  s331 -> s330 [order 3] : R3d {send(R3d_o);}
  s332 -> s330 [order 3] : R3l {send(R3l_o);}
  s384 -> s330 [order 1] : R1d {send(R1d_o);}
  s330 -> s384 [order 1] : R1u {send(R1u_o);}
  s330 -> s332 [order 4] : R3r {send(R3r_o);}
  s330 -> s331 [order 5] : R3u {send(R3u_o);}
  s333 -> s331 [order 5] : R3l {send(R3l_o);}
  s385 -> s331 [order 1] : R1d {send(R1d_o);}
  s331 -> s385 [order 1] : R1u {send(R1u_o);}
  s331 -> s333 [order 5] : R3r {send(R3r_o);}
  s333 -> s332 [order 4] : R3d {send(R3d_o);}
  s338 -> s332 [order 2] : R2d {send(R2d_o);}
  s332 -> s338 [order 2] : R2u {send(R2u_o);}
  s332 -> s333 [order 4] : R3u {send(R3u_o);}
  s332 -> s333 [order 5] : R3ureq {send(R3ureq_o);}
  s339 -> s333 [order 3] : R2d {send(R2d_o);}
  s387 -> s333 [order 1] : R1d {send(R1d_o);}
  s333 -> s387 [order 1] : R1u {send(R1u_o);}
  s333 -> s339 [order 3] : R2u {send(R2u_o);}
  s335 -> s334 [order 7] : R3d {send(R3d_o);}
  s337 -> s334 [order 6] : R3l {send(R3l_o);}
  s340 -> s334 [order 3] : R2d {send(R2d_o);}
  s347 -> s334 [order 2] : R2l {send(R2l_o);}
  s388 -> s334 [order 1] : R1d {send(R1d_o);}
  s334 -> s388 [order 2] : R1u {send(R1u_o);}
  s334 -> s347 [order 5] : R2r {send(R2r_o);}
  s334 -> s340 [order 6] : R2u {send(R2u_o);}
  s334 -> s340 [order 7] : R2ureq {send(R2ureq_o);}
  s334 -> s337 [order 8] : R3r {send(R3r_o);}
  s334 -> s335 [order 9] : R3u {send(R3u_o);}
  s336 -> s335 [order 8] : R3d {send(R3d_o);}
  s341 -> s335 [order 3] : R2d {send(R2d_o);}
  s348 -> s335 [order 2] : R2l {send(R2l_o);}
  s389 -> s335 [order 1] : R1d {send(R1d_o);}
  s335 -> s389 [order 2] : R1u {send(R1u_o);}
  s335 -> s348 [order 4] : R2r {send(R2r_o);}
  s335 -> s341 [order 5] : R2u {send(R2u_o);}
  s335 -> s341 [order 6] : R2ureq {send(R2ureq_o);}
  s335 -> s336 [order 8] : R3u {send(R3u_o);}
  s342 -> s336 [order 3] : R2d {send(R2d_o);}
  s349 -> s336 [order 2] : R2l {send(R2l_o);}
  s390 -> s336 [order 1] : R1d {send(R1d_o);}
  s336 -> s390 [order 2] : R1u {send(R1u_o);}
  s336 -> s349 [order 5] : R2r {send(R2r_o);}
  s336 -> s342 [order 6] : R2u {send(R2u_o);}
  s336 -> s342 [order 7] : R2ureq {send(R2ureq_o);}
  s343 -> s337 [order 2] : R2d {send(R2d_o);}
  s350 -> s337 [order 1] : R2l {send(R2l_o);}
  s391 -> s337 [order 1] : R1d {send(R1d_o);}
  s337 -> s391 [order 1] : R1u {send(R1u_o);}
  s337 -> s350 [order 3] : R2r {send(R2r_o);}
  s337 -> s343 [order 4] : R2u {send(R2u_o);}
  s337 -> s343 [order 5] : R2ureq {send(R2ureq_o);}
  s339 -> s338 [order 8] : R3d {send(R3d_o);}
  s345 -> s338 [order 2] : R2d {send(R2d_o);}
  s338 -> s345 [order 4] : R2u {send(R2u_o);}
  s338 -> s345 [order 5] : R2ureq {send(R2ureq_o);}
  s338 -> s339 [order 6] : R3u {send(R3u_o);}
  s338 -> s339 [order 7] : R3ureq {send(R3ureq_o);}
  s346 -> s339 [order 3] : R2d {send(R2d_o);}
  s353 -> s339 [order 2] : R2l {send(R2l_o);}
  s393 -> s339 [order 1] : R1d {send(R1d_o);}
  s339 -> s393 [order 2] : R1u {send(R1u_o);}
  s339 -> s353 [order 5] : R2r {send(R2r_o);}
  s339 -> s346 [order 6] : R2u {send(R2u_o);}
  s339 -> s346 [order 7] : R2ureq {send(R2ureq_o);}
  s341 -> s340 [order 6] : R3d {send(R3d_o);}
  s343 -> s340 [order 5] : R3l {send(R3l_o);}
  s354 -> s340 [order 4] : R2l {send(R2l_o);}
  s394 -> s340 [order 1] : R1d {send(R1d_o);}
  s340 -> s394 [order 2] : R1u {send(R1u_o);}
  s340 -> s354 [order 5] : R2r {send(R2r_o);}
  s340 -> s343 [order 6] : R3r {send(R3r_o);}
  s340 -> s341 [order 7] : R3u {send(R3u_o);}
  s342 -> s341 [order 5] : R3d {send(R3d_o);}
  s344 -> s341 [order 6] : R3l {send(R3l_o);}
  s355 -> s341 [order 4] : R2l {send(R2l_o);}
  s395 -> s341 [order 1] : R1d {send(R1d_o);}
  s341 -> s395 [order 2] : R1u {send(R1u_o);}
  s341 -> s355 [order 5] : R2r {send(R2r_o);}
  s341 -> s344 [order 7] : R3r {send(R3r_o);}
  s341 -> s342 [order 8] : R3u {send(R3u_o);}
  s356 -> s342 [order 4] : R2l {send(R2l_o);}
  s396 -> s342 [order 1] : R1d {send(R1d_o);}
  s342 -> s396 [order 2] : R1u {send(R1u_o);}
  s342 -> s356 [order 4] : R2r {send(R2r_o);}
  s344 -> s343 [order 5] : R3d {send(R3d_o);}
  s357 -> s343 [order 3] : R2l {send(R2l_o);}
  s397 -> s343 [order 1] : R1d {send(R1d_o);}
  s343 -> s397 [order 1] : R1u {send(R1u_o);}
  s343 -> s357 [order 4] : R2r {send(R2r_o);}
  s343 -> s344 [order 6] : R3u {send(R3u_o);}
  s345 -> s344 [order 4] : R3l {send(R3l_o);}
  s358 -> s344 [order 4] : R2l {send(R2l_o);}
  s398 -> s344 [order 1] : R1d {send(R1d_o);}
  s344 -> s398 [order 2] : R1u {send(R1u_o);}
  s344 -> s358 [order 4] : R2r {send(R2r_o);}
  s344 -> s345 [order 7] : R3r {send(R3r_o);}
  s346 -> s345 [order 5] : R3d {send(R3d_o);}
  s345 -> s346 [order 5] : R3u {send(R3u_o);}
  s345 -> s346 [order 6] : R3ureq {send(R3ureq_o);}
  s400 -> s346 [order 1] : R1d {send(R1d_o);}
  s346 -> s400 [order 2] : R1u {send(R1u_o);}
  s348 -> s347 [order 4] : R3d {send(R3d_o);}
  s350 -> s347 [order 3] : R3l {send(R3l_o);}
  s354 -> s347 [order 3] : R2d {send(R2d_o);}
  s347 -> s354 [order 3] : R2u {send(R2u_o);}
  s347 -> s350 [order 4] : R3r {send(R3r_o);}
  s347 -> s348 [order 5] : R3u {send(R3u_o);}
  s349 -> s348 [order 4] : R3d {send(R3d_o);}
  s351 -> s348 [order 4] : R3l {send(R3l_o);}
  s355 -> s348 [order 3] : R2d {send(R2d_o);}
  s348 -> s355 [order 3] : R2u {send(R2u_o);}
  s348 -> s351 [order 5] : R3r {send(R3r_o);}
  s348 -> s349 [order 6] : R3u {send(R3u_o);}
  s352 -> s349 [order 4] : R3l {send(R3l_o);}
  s356 -> s349 [order 3] : R2d {send(R2d_o);}
  s349 -> s356 [order 3] : R2u {send(R2u_o);}
  s349 -> s352 [order 5] : R3r {send(R3r_o);}
  s351 -> s350 [order 3] : R3d {send(R3d_o);}
  s357 -> s350 [order 2] : R2d {send(R2d_o);}
  s350 -> s357 [order 2] : R2u {send(R2u_o);}
  s350 -> s351 [order 4] : R3u {send(R3u_o);}
  s352 -> s351 [order 3] : R3d {send(R3d_o);}
  s358 -> s351 [order 3] : R2d {send(R2d_o);}
  s351 -> s358 [order 2] : R2u {send(R2u_o);}
  s351 -> s352 [order 5] : R3u {send(R3u_o);}
  s353 -> s352 [order 3] : R3l {send(R3l_o);}
  s359 -> s352 [order 3] : R2d {send(R2d_o);}
  s352 -> s359 [order 2] : R2u {send(R2u_o);}
  s352 -> s353 [order 5] : R3r {send(R3r_o);}
  s355 -> s354 [order 5] : R3d {send(R3d_o);}
  s357 -> s354 [order 4] : R3l {send(R3l_o);}
  s408 -> s354 [order 1] : R1d {send(R1d_o);}
  s354 -> s408 [order 2] : R1u {send(R1u_o);}
  s354 -> s357 [order 5] : R3r {send(R3r_o);}
  s354 -> s355 [order 6] : R3u {send(R3u_o);}
  s356 -> s355 [order 5] : R3d {send(R3d_o);}
  s358 -> s355 [order 6] : R3l {send(R3l_o);}
  s409 -> s355 [order 1] : R1d {send(R1d_o);}
  s355 -> s409 [order 2] : R1u {send(R1u_o);}
  s355 -> s358 [order 6] : R3r {send(R3r_o);}
  s355 -> s356 [order 7] : R3u {send(R3u_o);}
  s359 -> s356 [order 5] : R3l {send(R3l_o);}
  s410 -> s356 [order 1] : R1d {send(R1d_o);}
  s356 -> s410 [order 2] : R1u {send(R1u_o);}
  s356 -> s359 [order 6] : R3r {send(R3r_o);}
  s358 -> s357 [order 5] : R3d {send(R3d_o);}
  s411 -> s357 [order 1] : R1d {send(R1d_o);}
  s357 -> s411 [order 1] : R1u {send(R1u_o);}
  s357 -> s358 [order 5] : R3u {send(R3u_o);}
  s359 -> s358 [order 4] : R3d {send(R3d_o);}
  s412 -> s358 [order 1] : R1d {send(R1d_o);}
  s358 -> s412 [order 2] : R1u {send(R1u_o);}
  s358 -> s359 [order 7] : R3u {send(R3u_o);}
  s413 -> s359 [order 1] : R1d {send(R1d_o);}
  s359 -> s413 [order 2] : R1u {send(R1u_o);}
  s361 -> s360 [order 6] : R3d {send(R3d_o);}
  s363 -> s360 [order 6] : R3l {send(R3l_o);}
  s382 -> s360 [order 4] : R2l {send(R2l_o);}
  s415 -> s360 [order 1] : R1d {send(R1d_o);}
  s360 -> s415 [order 3] : R1u {send(R1u_o);}
  s360 -> s382 [order 4] : R2r {send(R2r_o);}
  s360 -> s363 [order 5] : R3r {send(R3r_o);}
  s360 -> s361 [order 6] : R3u {send(R3u_o);}
  s364 -> s361 [order 7] : R3l {send(R3l_o);}
  s368 -> s361 [order 4] : R2d {send(R2d_o);}
  s383 -> s361 [order 4] : R2l {send(R2l_o);}
  s416 -> s361 [order 1] : R1d {send(R1d_o);}
  s361 -> s416 [order 3] : R1u {send(R1u_o);}
  s361 -> s383 [order 4] : R2r {send(R2r_o);}
  s361 -> s368 [order 5] : R2u {send(R2u_o);}
  s361 -> s364 [order 7] : R3r {send(R3r_o);}
  s363 -> s362 [order 5] : R3d {send(R3d_o);}
  s365 -> s362 [order 5] : R3l {send(R3l_o);}
  s369 -> s362 [order 4] : R2d {send(R2d_o);}
  s417 -> s362 [order 1] : R1d {send(R1d_o);}
  s362 -> s417 [order 3] : R1u {send(R1u_o);}
  s362 -> s369 [order 4] : R2u {send(R2u_o);}
  s362 -> s365 [order 5] : R3r {send(R3r_o);}
  s362 -> s363 [order 6] : R3u {send(R3u_o);}
  s364 -> s363 [order 6] : R3d {send(R3d_o);}
  s370 -> s363 [order 3] : R2d {send(R2d_o);}
  s384 -> s363 [order 3] : R2l {send(R2l_o);}
  s418 -> s363 [order 1] : R1d {send(R1d_o);}
  s363 -> s418 [order 2] : R1u {send(R1u_o);}
  s363 -> s384 [order 3] : R2r {send(R2r_o);}
  s363 -> s370 [order 4] : R2u {send(R2u_o);}
  s363 -> s364 [order 7] : R3u {send(R3u_o);}
  s366 -> s364 [order 5] : R3l {send(R3l_o);}
  s371 -> s364 [order 4] : R2d {send(R2d_o);}
  s385 -> s364 [order 4] : R2l {send(R2l_o);}
  s419 -> s364 [order 1] : R1d {send(R1d_o);}
  s364 -> s419 [order 3] : R1u {send(R1u_o);}
  s364 -> s385 [order 4] : R2r {send(R2r_o);}
  s364 -> s371 [order 5] : R2u {send(R2u_o);}
  s364 -> s366 [order 8] : R3r {send(R3r_o);}
  s372 -> s365 [order 3] : R2d {send(R2d_o);}
  s386 -> s365 [order 3] : R2l {send(R2l_o);}
  s420 -> s365 [order 1] : R1d {send(R1d_o);}
  s365 -> s420 [order 2] : R1u {send(R1u_o);}
  s365 -> s386 [order 3] : R2r {send(R2r_o);}
  s365 -> s372 [order 4] : R2u {send(R2u_o);}
  s373 -> s366 [order 3] : R2d {send(R2d_o);}
  s387 -> s366 [order 3] : R2l {send(R2l_o);}
  s366 -> s387 [order 3] : R2r {send(R2r_o);}
  s366 -> s373 [order 4] : R2u {send(R2u_o);}
  s369 -> s367 [order 7] : R3l {send(R3l_o);}
  s374 -> s367 [order 4] : R2d {send(R2d_o);}
  s388 -> s367 [order 4] : R2l {send(R2l_o);}
  s421 -> s367 [order 1] : R1d {send(R1d_o);}
  s367 -> s421 [order 3] : R1u {send(R1u_o);}
  s367 -> s388 [order 4] : R2r {send(R2r_o);}
  s367 -> s374 [order 5] : R2u {send(R2u_o);}
  s367 -> s369 [order 6] : R3r {send(R3r_o);}
  s371 -> s368 [order 7] : R3l {send(R3l_o);}
  s390 -> s368 [order 4] : R2l {send(R2l_o);}
  s422 -> s368 [order 1] : R1d {send(R1d_o);}
  s368 -> s422 [order 3] : R1u {send(R1u_o);}
  s368 -> s390 [order 5] : R2r {send(R2r_o);}
  s368 -> s371 [order 6] : R3r {send(R3r_o);}
  s370 -> s369 [order 5] : R3d {send(R3d_o);}
  s372 -> s369 [order 6] : R3l {send(R3l_o);}
  s376 -> s369 [order 4] : R2d {send(R2d_o);}
  s391 -> s369 [order 3] : R2l {send(R2l_o);}
  s423 -> s369 [order 1] : R1d {send(R1d_o);}
  s369 -> s423 [order 3] : R1u {send(R1u_o);}
  s369 -> s391 [order 5] : R2r {send(R2r_o);}
  s369 -> s376 [order 6] : R2u {send(R2u_o);}
  s369 -> s372 [order 8] : R3r {send(R3r_o);}
  s369 -> s370 [order 9] : R3u {send(R3u_o);}
  s371 -> s370 [order 6] : R3d {send(R3d_o);}
  s377 -> s370 [order 3] : R2d {send(R2d_o);}
  s424 -> s370 [order 1] : R1d {send(R1d_o);}
  s370 -> s424 [order 2] : R1u {send(R1u_o);}
  s370 -> s377 [order 4] : R2u {send(R2u_o);}
  s370 -> s371 [order 6] : R3u {send(R3u_o);}
  s373 -> s371 [order 6] : R3l {send(R3l_o);}
  s378 -> s371 [order 4] : R2d {send(R2d_o);}
  s425 -> s371 [order 1] : R1d {send(R1d_o);}
  s371 -> s425 [order 3] : R1u {send(R1u_o);}
  s371 -> s378 [order 5] : R2u {send(R2u_o);}
  s371 -> s373 [order 8] : R3r {send(R3r_o);}
  s379 -> s372 [order 3] : R2d {send(R2d_o);}
  s392 -> s372 [order 3] : R2l {send(R2l_o);}
  s426 -> s372 [order 1] : R1d {send(R1d_o);}
  s372 -> s426 [order 2] : R1u {send(R1u_o);}
  s372 -> s392 [order 4] : R2r {send(R2r_o);}
  s372 -> s379 [order 5] : R2u {send(R2u_o);}
  s380 -> s373 [order 3] : R2d {send(R2d_o);}
  s393 -> s373 [order 3] : R2l {send(R2l_o);}
  s373 -> s393 [order 4] : R2r {send(R2r_o);}
  s373 -> s380 [order 5] : R2u {send(R2u_o);}
  s375 -> s374 [order 5] : R3d {send(R3d_o);}
  s376 -> s374 [order 6] : R3l {send(R3l_o);}
  s394 -> s374 [order 5] : R2l {send(R2l_o);}
  s427 -> s374 [order 1] : R1d {send(R1d_o);}
  s374 -> s427 [order 3] : R1u {send(R1u_o);}
  s374 -> s394 [order 5] : R2r {send(R2r_o);}
  s374 -> s376 [order 6] : R3r {send(R3r_o);}
  s374 -> s375 [order 7] : R3u {send(R3u_o);}
  s377 -> s375 [order 6] : R3l {send(R3l_o);}
  s395 -> s375 [order 5] : R2l {send(R2l_o);}
  s428 -> s375 [order 1] : R1d {send(R1d_o);}
  s375 -> s428 [order 3] : R1u {send(R1u_o);}
  s375 -> s395 [order 4] : R2r {send(R2r_o);}
  s375 -> s377 [order 6] : R3r {send(R3r_o);}
  s377 -> s376 [order 5] : R3d {send(R3d_o);}
  s379 -> s376 [order 5] : R3l {send(R3l_o);}
  s397 -> s376 [order 5] : R2l {send(R2l_o);}
  s429 -> s376 [order 1] : R1d {send(R1d_o);}
  s376 -> s429 [order 3] : R1u {send(R1u_o);}
  s376 -> s397 [order 5] : R2r {send(R2r_o);}
  s376 -> s379 [order 7] : R3r {send(R3r_o);}
  s376 -> s377 [order 8] : R3u {send(R3u_o);}
  s378 -> s377 [order 5] : R3d {send(R3d_o);}
  s398 -> s377 [order 3] : R2l {send(R2l_o);}
  s430 -> s377 [order 1] : R1d {send(R1d_o);}
  s377 -> s430 [order 2] : R1u {send(R1u_o);}
  s377 -> s398 [order 4] : R2r {send(R2r_o);}
  s377 -> s378 [order 7] : R3u {send(R3u_o);}
  s380 -> s378 [order 5] : R3l {send(R3l_o);}
  s431 -> s378 [order 1] : R1d {send(R1d_o);}
  s378 -> s431 [order 3] : R1u {send(R1u_o);}
  s378 -> s380 [order 6] : R3r {send(R3r_o);}
  s399 -> s379 [order 4] : R2l {send(R2l_o);}
  s432 -> s379 [order 1] : R1d {send(R1d_o);}
  s379 -> s432 [order 2] : R1u {send(R1u_o);}
  s379 -> s399 [order 4] : R2r {send(R2r_o);}
  s400 -> s380 [order 4] : R2l {send(R2l_o);}
  s380 -> s400 [order 4] : R2r {send(R2r_o);}
  s382 -> s381 [order 7] : R3d {send(R3d_o);}
  s388 -> s381 [order 3] : R2d {send(R2d_o);}
  s401 -> s381 [order 3] : R2l {send(R2l_o);}
  s433 -> s381 [order 1] : R1d {send(R1d_o);}
  s381 -> s433 [order 3] : R1u {send(R1u_o);}
  s381 -> s401 [order 4] : R2r {send(R2r_o);}
  s381 -> s388 [order 5] : R2u {send(R2u_o);}
  s381 -> s382 [order 6] : R3u {send(R3u_o);}
  s383 -> s382 [order 7] : R3d {send(R3d_o);}
  s384 -> s382 [order 5] : R3l {send(R3l_o);}
  s389 -> s382 [order 3] : R2d {send(R2d_o);}
  s402 -> s382 [order 3] : R2l {send(R2l_o);}
  s434 -> s382 [order 1] : R1d {send(R1d_o);}
  s382 -> s434 [order 3] : R1u {send(R1u_o);}
  s382 -> s402 [order 5] : R2r {send(R2r_o);}
  s382 -> s389 [order 6] : R2u {send(R2u_o);}
  s382 -> s384 [order 8] : R3r {send(R3r_o);}
  s382 -> s383 [order 9] : R3u {send(R3u_o);}
  s385 -> s383 [order 7] : R3l {send(R3l_o);}
  s390 -> s383 [order 3] : R2d {send(R2d_o);}
  s403 -> s383 [order 3] : R2l {send(R2l_o);}
  s435 -> s383 [order 1] : R1d {send(R1d_o);}
  s383 -> s435 [order 3] : R1u {send(R1u_o);}
  s383 -> s403 [order 5] : R2r {send(R2r_o);}
  s383 -> s390 [order 6] : R2u {send(R2u_o);}
  s383 -> s385 [order 8] : R3r {send(R3r_o);}
  s385 -> s384 [order 6] : R3d {send(R3d_o);}
  s405 -> s384 [order 2] : R2l {send(R2l_o);}
  s436 -> s384 [order 1] : R1d {send(R1d_o);}
  s384 -> s436 [order 2] : R1u {send(R1u_o);}
  s384 -> s405 [order 4] : R2r {send(R2r_o);}
  s384 -> s385 [order 6] : R3u {send(R3u_o);}
  s387 -> s385 [order 6] : R3l {send(R3l_o);}
  s406 -> s385 [order 3] : R2l {send(R2l_o);}
  s437 -> s385 [order 1] : R1d {send(R1d_o);}
  s385 -> s437 [order 3] : R1u {send(R1u_o);}
  s385 -> s406 [order 5] : R2r {send(R2r_o);}
  s385 -> s387 [order 8] : R3r {send(R3r_o);}
  s392 -> s386 [order 2] : R2d {send(R2d_o);}
  s438 -> s386 [order 1] : R1d {send(R1d_o);}
  s386 -> s438 [order 2] : R1u {send(R1u_o);}
  s386 -> s392 [order 4] : R2u {send(R2u_o);}
  s393 -> s387 [order 2] : R2d {send(R2d_o);}
  s407 -> s387 [order 2] : R2l {send(R2l_o);}
  s387 -> s407 [order 4] : R2r {send(R2r_o);}
  s387 -> s393 [order 5] : R2u {send(R2u_o);}
  s389 -> s388 [order 6] : R3d {send(R3d_o);}
  s391 -> s388 [order 6] : R3l {send(R3l_o);}
  s394 -> s388 [order 4] : R2d {send(R2d_o);}
  s439 -> s388 [order 1] : R1d {send(R1d_o);}
  s388 -> s439 [order 2] : R1u {send(R1u_o);}
  s388 -> s394 [order 5] : R2u {send(R2u_o);}
  s388 -> s394 [order 6] : R2ureq {send(R2ureq_o);}
  s388 -> s391 [order 7] : R3r {send(R3r_o);}
  s388 -> s389 [order 8] : R3u {send(R3u_o);}
  s390 -> s389 [order 7] : R3d {send(R3d_o);}
  s395 -> s389 [order 4] : R2d {send(R2d_o);}
  s440 -> s389 [order 1] : R1d {send(R1d_o);}
  s389 -> s440 [order 2] : R1u {send(R1u_o);}
  s389 -> s395 [order 4] : R2u {send(R2u_o);}
  s389 -> s395 [order 5] : R2ureq {send(R2ureq_o);}
  s389 -> s390 [order 7] : R3u {send(R3u_o);}
  s396 -> s390 [order 4] : R2d {send(R2d_o);}
  s441 -> s390 [order 1] : R1d {send(R1d_o);}
  s390 -> s441 [order 2] : R1u {send(R1u_o);}
  s390 -> s396 [order 5] : R2u {send(R2u_o);}
  s390 -> s396 [order 6] : R2ureq {send(R2ureq_o);}
  s392 -> s391 [order 6] : R3l {send(R3l_o);}
  s397 -> s391 [order 4] : R2d {send(R2d_o);}
  s442 -> s391 [order 1] : R1d {send(R1d_o);}
  s391 -> s442 [order 2] : R1u {send(R1u_o);}
  s391 -> s397 [order 4] : R2u {send(R2u_o);}
  s391 -> s397 [order 5] : R2ureq {send(R2ureq_o);}
  s391 -> s392 [order 7] : R3r {send(R3r_o);}
  s399 -> s392 [order 3] : R2d {send(R2d_o);}
  s443 -> s392 [order 1] : R1d {send(R1d_o);}
  s392 -> s443 [order 1] : R1u {send(R1u_o);}
  s392 -> s399 [order 4] : R2u {send(R2u_o);}
  s392 -> s399 [order 5] : R2ureq {send(R2ureq_o);}
  s400 -> s393 [order 3] : R2d {send(R2d_o);}
  s393 -> s400 [order 4] : R2u {send(R2u_o);}
  s393 -> s400 [order 5] : R2ureq {send(R2ureq_o);}
  s395 -> s394 [order 7] : R3d {send(R3d_o);}
  s397 -> s394 [order 7] : R3l {send(R3l_o);}
  s408 -> s394 [order 3] : R2l {send(R2l_o);}
  s444 -> s394 [order 1] : R1d {send(R1d_o);}
  s394 -> s444 [order 3] : R1u {send(R1u_o);}
  s394 -> s408 [order 6] : R2r {send(R2r_o);}
  s394 -> s397 [order 7] : R3r {send(R3r_o);}
  s394 -> s395 [order 8] : R3u {send(R3u_o);}
  s396 -> s395 [order 6] : R3d {send(R3d_o);}
  s398 -> s395 [order 6] : R3l {send(R3l_o);}
  s409 -> s395 [order 3] : R2l {send(R2l_o);}
  s445 -> s395 [order 1] : R1d {send(R1d_o);}
  s395 -> s445 [order 3] : R1u {send(R1u_o);}
  s395 -> s409 [order 6] : R2r {send(R2r_o);}
  s395 -> s398 [order 8] : R3r {send(R3r_o);}
  s395 -> s396 [order 9] : R3u {send(R3u_o);}
  s410 -> s396 [order 3] : R2l {send(R2l_o);}
  s446 -> s396 [order 1] : R1d {send(R1d_o);}
  s396 -> s446 [order 3] : R1u {send(R1u_o);}
  s396 -> s410 [order 5] : R2r {send(R2r_o);}
  s398 -> s397 [order 5] : R3d {send(R3d_o);}
  s399 -> s397 [order 6] : R3l {send(R3l_o);}
  s411 -> s397 [order 3] : R2l {send(R2l_o);}
  s447 -> s397 [order 1] : R1d {send(R1d_o);}
  s397 -> s447 [order 3] : R1u {send(R1u_o);}
  s397 -> s411 [order 6] : R2r {send(R2r_o);}
  s397 -> s399 [order 8] : R3r {send(R3r_o);}
  s397 -> s398 [order 9] : R3u {send(R3u_o);}
  s412 -> s398 [order 2] : R2l {send(R2l_o);}
  s448 -> s398 [order 1] : R1d {send(R1d_o);}
  s398 -> s448 [order 2] : R1u {send(R1u_o);}
  s398 -> s412 [order 4] : R2r {send(R2r_o);}
  s414 -> s399 [order 2] : R2l {send(R2l_o);}
  s449 -> s399 [order 1] : R1d {send(R1d_o);}
  s399 -> s449 [order 2] : R1u {send(R1u_o);}
  s399 -> s414 [order 5] : R2r {send(R2r_o);}
  s402 -> s401 [order 4] : R3d {send(R3d_o);}
  s404 -> s401 [order 3] : R3l {send(R3l_o);}
  s450 -> s401 [order 1] : R1d {send(R1d_o);}
  s401 -> s450 [order 2] : R1u {send(R1u_o);}
  s401 -> s404 [order 4] : R3r {send(R3r_o);}
  s401 -> s402 [order 5] : R3u {send(R3u_o);}
  s403 -> s402 [order 4] : R3d {send(R3d_o);}
  s405 -> s402 [order 4] : R3l {send(R3l_o);}
  s451 -> s402 [order 1] : R1d {send(R1d_o);}
  s402 -> s451 [order 2] : R1u {send(R1u_o);}
  s402 -> s405 [order 5] : R3r {send(R3r_o);}
  s402 -> s403 [order 6] : R3u {send(R3u_o);}
  s406 -> s403 [order 5] : R3l {send(R3l_o);}
  s452 -> s403 [order 1] : R1d {send(R1d_o);}
  s403 -> s452 [order 2] : R1u {send(R1u_o);}
  s403 -> s406 [order 5] : R3r {send(R3r_o);}
  s405 -> s404 [order 3] : R3d {send(R3d_o);}
  s453 -> s404 [order 1] : R1d {send(R1d_o);}
  s404 -> s453 [order 2] : R1u {send(R1u_o);}
  s404 -> s405 [order 4] : R3u {send(R3u_o);}
  s406 -> s405 [order 4] : R3d {send(R3d_o);}
  s454 -> s405 [order 1] : R1d {send(R1d_o);}
  s405 -> s454 [order 1] : R1u {send(R1u_o);}
  s405 -> s406 [order 5] : R3u {send(R3u_o);}
  s407 -> s406 [order 3] : R3l {send(R3l_o);}
  s455 -> s406 [order 1] : R1d {send(R1d_o);}
  s406 -> s455 [order 2] : R1u {send(R1u_o);}
  s406 -> s407 [order 6] : R3r {send(R3r_o);}
  s409 -> s408 [order 4] : R3d {send(R3d_o);}
  s411 -> s408 [order 4] : R3l {send(R3l_o);}
  s408 -> s411 [order 4] : R3r {send(R3r_o);}
  s408 -> s409 [order 5] : R3u {send(R3u_o);}
  s410 -> s409 [order 4] : R3d {send(R3d_o);}
  s412 -> s409 [order 4] : R3l {send(R3l_o);}
  s409 -> s412 [order 5] : R3r {send(R3r_o);}
  s409 -> s410 [order 6] : R3u {send(R3u_o);}
  s413 -> s410 [order 4] : R3l {send(R3l_o);}
  s410 -> s413 [order 5] : R3r {send(R3r_o);}
  s412 -> s411 [order 3] : R3d {send(R3d_o);}
  s414 -> s411 [order 3] : R3l {send(R3l_o);}
  s411 -> s414 [order 5] : R3r {send(R3r_o);}
  s411 -> s412 [order 6] : R3u {send(R3u_o);}
  s413 -> s412 [order 3] : R3d {send(R3d_o);}
  s412 -> s413 [order 5] : R3u {send(R3u_o);}
  s416 -> s415 [order 5] : R3d {send(R3d_o);}
  s418 -> s415 [order 6] : R3l {send(R3l_o);}
  s434 -> s415 [order 3] : R2l {send(R2l_o);}
  s415 -> s434 [order 3] : R2r {send(R2r_o);}
  s415 -> s418 [order 4] : R3r {send(R3r_o);}
  s415 -> s416 [order 5] : R3u {send(R3u_o);}
  s419 -> s416 [order 5] : R3l {send(R3l_o);}
  s422 -> s416 [order 3] : R2d {send(R2d_o);}
  s435 -> s416 [order 3] : R2l {send(R2l_o);}
  s416 -> s435 [order 3] : R2r {send(R2r_o);}
  s416 -> s422 [order 4] : R2u {send(R2u_o);}
  s416 -> s419 [order 6] : R3r {send(R3r_o);}
  s418 -> s417 [order 5] : R3d {send(R3d_o);}
  s420 -> s417 [order 5] : R3l {send(R3l_o);}
  s423 -> s417 [order 3] : R2d {send(R2d_o);}
  s417 -> s423 [order 3] : R2u {send(R2u_o);}
  s417 -> s420 [order 4] : R3r {send(R3r_o);}
  s417 -> s418 [order 5] : R3u {send(R3u_o);}
  s419 -> s418 [order 4] : R3d {send(R3d_o);}
  s424 -> s418 [order 3] : R2d {send(R2d_o);}
  s436 -> s418 [order 3] : R2l {send(R2l_o);}
  s418 -> s436 [order 3] : R2r {send(R2r_o);}
  s418 -> s424 [order 4] : R2u {send(R2u_o);}
  s418 -> s419 [order 7] : R3u {send(R3u_o);}
  s425 -> s419 [order 2] : R2d {send(R2d_o);}
  s437 -> s419 [order 2] : R2l {send(R2l_o);}
  s419 -> s437 [order 2] : R2r {send(R2r_o);}
  s419 -> s425 [order 3] : R2u {send(R2u_o);}
  s426 -> s420 [order 3] : R2d {send(R2d_o);}
  s438 -> s420 [order 3] : R2l {send(R2l_o);}
  s420 -> s438 [order 3] : R2r {send(R2r_o);}
  s420 -> s426 [order 4] : R2u {send(R2u_o);}
  s423 -> s421 [order 6] : R3l {send(R3l_o);}
  s427 -> s421 [order 3] : R2d {send(R2d_o);}
  s439 -> s421 [order 3] : R2l {send(R2l_o);}
  s421 -> s439 [order 3] : R2r {send(R2r_o);}
  s421 -> s427 [order 4] : R2u {send(R2u_o);}
  s421 -> s423 [order 5] : R3r {send(R3r_o);}
  s425 -> s422 [order 5] : R3l {send(R3l_o);}
  s441 -> s422 [order 3] : R2l {send(R2l_o);}
  s422 -> s441 [order 4] : R2r {send(R2r_o);}
  s422 -> s425 [order 5] : R3r {send(R3r_o);}
  s424 -> s423 [order 5] : R3d {send(R3d_o);}
  s426 -> s423 [order 6] : R3l {send(R3l_o);}
  s429 -> s423 [order 3] : R2d {send(R2d_o);}
  s442 -> s423 [order 2] : R2l {send(R2l_o);}
  s423 -> s442 [order 4] : R2r {send(R2r_o);}
  s423 -> s429 [order 5] : R2u {send(R2u_o);}
  s423 -> s426 [order 7] : R3r {send(R3r_o);}
  s423 -> s424 [order 8] : R3u {send(R3u_o);}
  s425 -> s424 [order 4] : R3d {send(R3d_o);}
  s430 -> s424 [order 3] : R2d {send(R2d_o);}
  s424 -> s430 [order 4] : R2u {send(R2u_o);}
  s424 -> s425 [order 6] : R3u {send(R3u_o);}
  s431 -> s425 [order 2] : R2d {send(R2d_o);}
  s425 -> s431 [order 3] : R2u {send(R2u_o);}
  s432 -> s426 [order 3] : R2d {send(R2d_o);}
  s443 -> s426 [order 3] : R2l {send(R2l_o);}
  s426 -> s443 [order 4] : R2r {send(R2r_o);}
  s426 -> s432 [order 5] : R2u {send(R2u_o);}
  s428 -> s427 [order 4] : R3d {send(R3d_o);}
  s429 -> s427 [order 5] : R3l {send(R3l_o);}
  s444 -> s427 [order 3] : R2l {send(R2l_o);}
  s427 -> s444 [order 4] : R2r {send(R2r_o);}
  s427 -> s429 [order 5] : R3r {send(R3r_o);}
  s427 -> s428 [order 6] : R3u {send(R3u_o);}
  s430 -> s428 [order 6] : R3l {send(R3l_o);}
  s445 -> s428 [order 3] : R2l {send(R2l_o);}
  s428 -> s445 [order 3] : R2r {send(R2r_o);}
  s428 -> s430 [order 5] : R3r {send(R3r_o);}
  s430 -> s429 [order 5] : R3d {send(R3d_o);}
  s432 -> s429 [order 5] : R3l {send(R3l_o);}
  s447 -> s429 [order 3] : R2l {send(R2l_o);}
  s429 -> s447 [order 4] : R2r {send(R2r_o);}
  s429 -> s432 [order 6] : R3r {send(R3r_o);}
  s429 -> s430 [order 7] : R3u {send(R3u_o);}
  s431 -> s430 [order 3] : R3d {send(R3d_o);}
  s448 -> s430 [order 2] : R2l {send(R2l_o);}
  s430 -> s448 [order 4] : R2r {send(R2r_o);}
  s430 -> s431 [order 7] : R3u {send(R3u_o);}
  s449 -> s432 [order 3] : R2l {send(R2l_o);}
  s432 -> s449 [order 4] : R2r {send(R2r_o);}
  s434 -> s433 [order 6] : R3d {send(R3d_o);}
  s439 -> s433 [order 2] : R2d {send(R2d_o);}
  s450 -> s433 [order 3] : R2l {send(R2l_o);}
  s433 -> s450 [order 3] : R2r {send(R2r_o);}
  s433 -> s439 [order 4] : R2u {send(R2u_o);}
  s433 -> s434 [order 5] : R3u {send(R3u_o);}
  s435 -> s434 [order 6] : R3d {send(R3d_o);}
  s436 -> s434 [order 5] : R3l {send(R3l_o);}
  s440 -> s434 [order 2] : R2d {send(R2d_o);}
  s451 -> s434 [order 3] : R2l {send(R2l_o);}
  s434 -> s451 [order 4] : R2r {send(R2r_o);}
  s434 -> s440 [order 5] : R2u {send(R2u_o);}
  s434 -> s436 [order 7] : R3r {send(R3r_o);}
  s434 -> s435 [order 8] : R3u {send(R3u_o);}
  s437 -> s435 [order 5] : R3l {send(R3l_o);}
  s441 -> s435 [order 2] : R2d {send(R2d_o);}
  s452 -> s435 [order 3] : R2l {send(R2l_o);}
  s435 -> s452 [order 4] : R2r {send(R2r_o);}
  s435 -> s441 [order 5] : R2u {send(R2u_o);}
  s435 -> s437 [order 7] : R3r {send(R3r_o);}
  s437 -> s436 [order 4] : R3d {send(R3d_o);}
  s454 -> s436 [order 3] : R2l {send(R2l_o);}
  s436 -> s454 [order 4] : R2r {send(R2r_o);}
  s436 -> s437 [order 6] : R3u {send(R3u_o);}
  s455 -> s437 [order 2] : R2l {send(R2l_o);}
  s437 -> s455 [order 3] : R2r {send(R2r_o);}
  s443 -> s438 [order 2] : R2d {send(R2d_o);}
  s438 -> s443 [order 4] : R2u {send(R2u_o);}
  s440 -> s439 [order 6] : R3d {send(R3d_o);}
  s442 -> s439 [order 6] : R3l {send(R3l_o);}
  s444 -> s439 [order 2] : R2d {send(R2d_o);}
  s456 -> s439 [order 3] : R2l {send(R2l_o);}
  s439 -> s456 [order 4] : R2r {send(R2r_o);}
  s439 -> s444 [order 5] : R2u {send(R2u_o);}
  s439 -> s444 [order 6] : R2ureq {send(R2ureq_o);}
  s439 -> s442 [order 7] : R3r {send(R3r_o);}
  s439 -> s440 [order 8] : R3u {send(R3u_o);}
  s441 -> s440 [order 7] : R3d {send(R3d_o);}
  s445 -> s440 [order 2] : R2d {send(R2d_o);}
  s457 -> s440 [order 3] : R2l {send(R2l_o);}
  s440 -> s457 [order 3] : R2r {send(R2r_o);}
  s440 -> s445 [order 4] : R2u {send(R2u_o);}
  s440 -> s445 [order 5] : R2ureq {send(R2ureq_o);}
  s440 -> s441 [order 7] : R3u {send(R3u_o);}
  s446 -> s441 [order 2] : R2d {send(R2d_o);}
  s458 -> s441 [order 3] : R2l {send(R2l_o);}
  s441 -> s458 [order 4] : R2r {send(R2r_o);}
  s441 -> s446 [order 5] : R2u {send(R2u_o);}
  s441 -> s446 [order 6] : R2ureq {send(R2ureq_o);}
  s443 -> s442 [order 7] : R3l {send(R3l_o);}
  s447 -> s442 [order 2] : R2d {send(R2d_o);}
  s459 -> s442 [order 3] : R2l {send(R2l_o);}
  s442 -> s459 [order 3] : R2r {send(R2r_o);}
  s442 -> s447 [order 4] : R2u {send(R2u_o);}
  s442 -> s447 [order 5] : R2ureq {send(R2ureq_o);}
  s442 -> s443 [order 7] : R3r {send(R3r_o);}
  s449 -> s443 [order 2] : R2d {send(R2d_o);}
  s462 -> s443 [order 2] : R2l {send(R2l_o);}
  s443 -> s462 [order 4] : R2r {send(R2r_o);}
  s443 -> s449 [order 5] : R2u {send(R2u_o);}
  s443 -> s449 [order 6] : R2ureq {send(R2ureq_o);}
  s445 -> s444 [order 4] : R3d {send(R3d_o);}
  s447 -> s444 [order 4] : R3l {send(R3l_o);}
  s444 -> s447 [order 4] : R3r {send(R3r_o);}
  s444 -> s445 [order 5] : R3u {send(R3u_o);}
  s446 -> s445 [order 3] : R3d {send(R3d_o);}
  s448 -> s445 [order 4] : R3l {send(R3l_o);}
  s445 -> s448 [order 5] : R3r {send(R3r_o);}
  s445 -> s446 [order 6] : R3u {send(R3u_o);}
  s448 -> s447 [order 3] : R3d {send(R3d_o);}
  s449 -> s447 [order 4] : R3l {send(R3l_o);}
  s447 -> s449 [order 5] : R3r {send(R3r_o);}
  s447 -> s448 [order 6] : R3u {send(R3u_o);}
  s451 -> s450 [order 5] : R3d {send(R3d_o);}
  s453 -> s450 [order 4] : R3l {send(R3l_o);}
  s456 -> s450 [order 2] : R2d {send(R2d_o);}
  s450 -> s456 [order 4] : R2u {send(R2u_o);}
  s450 -> s453 [order 5] : R3r {send(R3r_o);}
  s450 -> s451 [order 6] : R3u {send(R3u_o);}
  s452 -> s451 [order 5] : R3d {send(R3d_o);}
  s454 -> s451 [order 6] : R3l {send(R3l_o);}
  s457 -> s451 [order 2] : R2d {send(R2d_o);}
  s451 -> s457 [order 4] : R2u {send(R2u_o);}
  s451 -> s454 [order 6] : R3r {send(R3r_o);}
  s451 -> s452 [order 7] : R3u {send(R3u_o);}
  s455 -> s452 [order 5] : R3l {send(R3l_o);}
  s458 -> s452 [order 2] : R2d {send(R2d_o);}
  s452 -> s458 [order 4] : R2u {send(R2u_o);}
  s452 -> s455 [order 6] : R3r {send(R3r_o);}
  s454 -> s453 [order 5] : R3d {send(R3d_o);}
  s459 -> s453 [order 2] : R2d {send(R2d_o);}
  s453 -> s459 [order 3] : R2u {send(R2u_o);}
  s453 -> s454 [order 5] : R3u {send(R3u_o);}
  s455 -> s454 [order 4] : R3d {send(R3d_o);}
  s460 -> s454 [order 2] : R2d {send(R2d_o);}
  s454 -> s460 [order 4] : R2u {send(R2u_o);}
  s454 -> s455 [order 7] : R3u {send(R3u_o);}
  s461 -> s455 [order 1] : R2d {send(R2d_o);}
  s455 -> s461 [order 3] : R2u {send(R2u_o);}
  s457 -> s456 [order 4] : R3d {send(R3d_o);}
  s459 -> s456 [order 4] : R3l {send(R3l_o);}
  s456 -> s459 [order 4] : R3r {send(R3r_o);}
  s456 -> s457 [order 5] : R3u {send(R3u_o);}
  s458 -> s457 [order 4] : R3d {send(R3d_o);}
  s460 -> s457 [order 4] : R3l {send(R3l_o);}
  s457 -> s460 [order 5] : R3r {send(R3r_o);}
  s457 -> s458 [order 6] : R3u {send(R3u_o);}
  s461 -> s458 [order 3] : R3l {send(R3l_o);}
  s458 -> s461 [order 5] : R3r {send(R3r_o);}
  s460 -> s459 [order 3] : R3d {send(R3d_o);}
  s462 -> s459 [order 3] : R3l {send(R3l_o);}
  s459 -> s462 [order 5] : R3r {send(R3r_o);}
  s459 -> s460 [order 6] : R3u {send(R3u_o);}
  s461 -> s460 [order 2] : R3d {send(R3d_o);}
  s460 -> s461 [order 5] : R3u {send(R3u_o);}
  events: R1d input RISING_EDGE_EVENT; R1d_o output FUNCTION_CALL_EVENT; R1l input RISING_EDGE_EVENT; R1l_o output FUNCTION_CALL_EVENT; R1r input RISING_EDGE_EVENT; R1r_o output FUNCTION_CALL_EVENT; R1u input RISING_EDGE_EVENT; R1u_o output FUNCTION_CALL_EVENT; R1ureq input RISING_EDGE_EVENT; R1ureq_o output FUNCTION_CALL_EVENT; R2d input RISING_EDGE_EVENT; R2d_o output FUNCTION_CALL_EVENT; R2l input RISING_EDGE_EVENT; R2l_o output FUNCTION_CALL_EVENT; R2r input RISING_EDGE_EVENT; R2r_o output FUNCTION_CALL_EVENT; R2u input RISING_EDGE_EVENT; R2u_o output FUNCTION_CALL_EVENT; R2ureq input RISING_EDGE_EVENT; R2ureq_o output FUNCTION_CALL_EVENT; R3d input RISING_EDGE_EVENT; R3d_o output FUNCTION_CALL_EVENT; R3l input RISING_EDGE_EVENT; R3l_o output FUNCTION_CALL_EVENT; R3r input RISING_EDGE_EVENT; R3r_o output FUNCTION_CALL_EVENT; R3u input RISING_EDGE_EVENT; R3u_o output FUNCTION_CALL_EVENT; R3ureq input RISING_EDGE_EVENT; R3ureq_o output FUNCTION_CALL_EVENT
